simulink model "Adaptive_CT_ur10v"  (R2021b)
settings: Solver=VariableStepAuto  StartTime=0.0  StopTime=15  FixedStep=1e-4  RelTol=1e1
values from neighbouring files (symbols this model uses):
  Kp = [100 0 0 0 0 0 0 250 0 0 0 0 ... (36 elements, 6x6)]    [ACT_workspace.mat]    (also in GuadagniControllore.m = 100 * diag([1 1 2 4 5 5]))
  Kv = [100 0 0 0 0 0 0 100 0 0 0 0 ... (36 elements, 6x6)]    [ACT_workspace.mat]    (also in GuadagniControllore.m = 100 * diag([1 1 3 3 5 5]))
  l1 = 0.1273    [ACT_workspace.mat]
  l2 = -0.612    [ACT_workspace.mat]
  l3 = -0.5723    [ACT_workspace.mat]
  l4 = 0.1639    [ACT_workspace.mat]
  l5 = 0.1157    [ACT_workspace.mat]
  l6 = 0.0922    [ACT_workspace.mat]
  m1 = 7.1    [ACT_workspace.mat]
  m2 = 12.7    [ACT_workspace.mat]
  m3 = 4.27    [ACT_workspace.mat]
  m4 = 2    [ACT_workspace.mat]
  m5 = 2    [ACT_workspace.mat]
  m6 = 0.365    [ACT_workspace.mat]
  q0 = [0 0 0 0 0 0]    [ACT_workspace.mat]
  r = 0.02    [ACT_workspace.mat]
undefined symbols (not defined in the file or in its folder): B, Spline
libraries: roblocks x2, robotcorelib x1, simulink x1
(part 17 of 20)

== matlab function Adaptive_CT_ur10v/CTA control/Subsystem/reg ==
  data: q input; Y output; qd input; qdd input
function Y = reg(q, qd, qdd)
%#codegen
q1 = q(1);
q2 = q(2);
q3 = q(3);
q4 = q(4);
q5 = q(5);
q6 = q(6);
qd1 = qd(1);
qd2 = qd(2);
qd3 = qd(3);
qd4 = qd(4);
qd5 = qd(5);
qd6 = qd(6);
qdd1 = qdd(1);
qdd2 = qdd(2);
qdd3 = qdd(3);
qdd4 = qdd(4);
qdd5 = qdd(5);
qdd6 = qdd(6);

%    This function was generated by the Symbolic Math Toolbox version 9.0.
%    26-Sep-2022 09:29:38

t2 = cos(q1);
t3 = cos(q2);
t4 = cos(q3);
t5 = cos(q4);
t6 = cos(q5);
t7 = cos(q6);
t8 = sin(q1);
t9 = sin(q2);
t10 = sin(q3);
t11 = sin(q4);
t12 = sin(q5);
t13 = sin(q6);
t14 = q2+q3;
t23 = -q5;
t15 = t2.^2;
t16 = t6.^2;
t17 = t8.^2;
t18 = t9.^2;
t19 = t12.^2;
t20 = cos(t14);
t21 = q4+t14;
t22 = sin(t14);
t24 = t2.*t6;
t26 = t2.*t12;
t27 = t6.*t8;
t30 = t8.*t12;
t33 = t3.*6.12e+3;
t34 = t9.*6.12e+3;
t56 = t3.*(1.53e+2./2.5e+2);
t57 = t2.*(1.53e+2./5.0e+2);
t63 = t9.*(1.53e+2./2.5e+2);
t64 = t8.*(1.53e+2./5.0e+2);
t90 = t2.*t3.*(-1.53e+2./2.5e+2);
t91 = t3.*t8.*(-1.53e+2./2.5e+2);
t92 = t2.*1.639e-1;
t93 = t2.*2.8615e-1;
t94 = t8.*1.639e-1;
t95 = t8.*2.8615e-1;
t119 = t3.*6.00372;
t138 = t8.*t9.*t10.*5.723e-1;
t148 = t2.*t3.*t4.*5.723e-1;
t152 = t2.*t3.*t10.*5.723e-1;
t153 = t2.*t4.*t9.*5.723e-1;
t154 = t3.*t4.*t8.*5.723e-1;
t157 = t2.*t9.*t10.*5.723e-1;
t158 = t3.*t8.*t10.*5.723e-1;
t159 = t4.*t8.*t9.*5.723e-1;
t25 = cos(t21);
t28 = q5+t21;
t29 = sin(t21);
t31 = t22.^2;
t41 = t21+t23;
t42 = t20.*5.723e+3;
t43 = t22.*5.723e+3;
t44 = t15+t17;
t71 = t2.*t56;
t74 = t2.*t63;
t75 = t8.*t56;
t79 = t8.*t63;
t109 = t20.*5.723e-1;
t110 = t24.*1.383e-1;
t111 = t24.*5.785e-2;
t112 = t22.*5.723e-1;
t113 = t26.*1.383e-1;
t114 = t27.*1.383e-1;
t115 = t26.*5.785e-2;
t116 = t27.*5.785e-2;
t117 = t30.*1.383e-1;
t118 = t30.*5.785e-2;
t122 = t5.*t20.*9.22e-2;
t123 = t11.*t20.*9.22e-2;
t124 = t5.*t22.*9.22e-2;
t125 = t11.*t22.*9.22e-2;
t127 = -t119;
t147 = t5.*t20.*1.157e-1;
t149 = t11.*t20.*1.157e-1;
t150 = t5.*t22.*1.157e-1;
t155 = t11.*t22.*1.157e-1;
t161 = -t138;
t172 = -t148;
t175 = t2.*t22.*(-5.723e-1);
t177 = t8.*t22.*(-5.723e-1);
t196 = t20.*5.614263;
t215 = t8.*t11.*t20.*(-1.157e-1);
t216 = t2.*t11.*t22.*(-1.157e-1);
t217 = t5.*t8.*t22.*(-1.157e-1);
t218 = t8.*t11.*t22.*(-1.157e-1);
t259 = t57+t91;
t32 = sin(t28);
t35 = t25.^2;
t36 = t29.^2;
t37 = t7.*t25;
t38 = t13.*t25;
t39 = t7.*t29;
t40 = t13.*t29;
t45 = sin(t41);
t46 = t24.*t25;
t49 = t25.*t26;
t50 = t25.*t27;
t58 = t25.*t30;
t87 = t25.*t29.*2.0;
t96 = t6.*t25.*t29;
t97 = t12.*t25.*t29;
t126 = -t109;
t128 = t25.*1.157e-1;
t129 = t25.*8.195e-2;
t130 = t29.*1.157e-1;
t131 = t29.*8.195e-2;
t137 = -t125;
t139 = t12.*t25.*4.61e-2;
t140 = t6.*t29.*4.61e-2;
t141 = t12.*t29.*4.61e-2;
t145 = t33+t42;
t146 = t34+t43;
t151 = t2.*t112;
t156 = t8.*t112;
t164 = t12.*t25.*5.785e-2;
t167 = t12.*t29.*5.785e-2;
t173 = -t149;
t174 = -t150;
t176 = -t155;
t178 = t15.*t112;
t179 = t17.*t112;
t181 = t8.*t29.*(-8.195e-2);
t182 = t2.*t147;
t183 = t2.*t149;
t184 = t8.*t147;
t185 = t2.*t150;
t186 = t8.*t149;
t187 = t2.*t155;
t188 = t8.*t150;
t191 = t8.*t155;
t206 = t29.*t113;
t208 = t29.*t115;
t209 = t29.*t117;
t210 = t29.*t118;
t211 = (t15.*t44)./5.0e+3;
t212 = (t17.*t44)./5.0e+3;
t220 = -t196;
t228 = t29.*1.135017;
t229 = t29.*8.039295e-1;
t234 = (t19.*t25.*t29)./2.5e+3;
t235 = (t19.*t25.*t29)./5.0e+3;
t251 = t64+t71;
t274 = t56+t109;
t275 = t63+t112;
t297 = t8.*t259;
t332 = t123+t124;
t345 = t17.*t25.*t29.*3.35790125e-3;
t346 = t17.*t25.*t29.*1.007370375e-2;
t354 = t15.*t25.*t29.*3.35790125e-3;
t355 = t15.*t25.*t29.*1.007370375e-2;
t374 = t3.*t57.*t259;
t375 = t74.*t259;
t480 = t25.*t29.*4.277201666666666e-3;
t487 = t25.*t29.*2.138600833333333e-3;
t514 = t25.*t29.*1.215540833333333e-3;
t515 = t25.*t29.*2.431081666666667e-3;
t519 = t15.*t44.*2.338600833333333e-3;
t521 = t17.*t44.*2.338600833333333e-3;
t47 = t2.*t37;
t48 = t6.*t37;
t51 = t2.*t38;
t52 = t8.*t37;
t53 = t2.*t39;
t54 = t6.*t38;
t55 = t6.*t39;
t59 = t8.*t38;
t60 = t2.*t40;
t61 = t8.*t39;
t62 = t6.*t40;
t65 = t8.*t40;
t66 = t6.*t35;
t67 = t12.*t35;
t68 = t6.*t36;
t69 = t12.*t36;
t70 = t24.*t39;
t72 = t24.*t40;
t73 = t27.*t39;
t76 = t15.*t36;
t78 = t27.*t40;
t80 = t17.*t36;
t81 = t19.*t36;
t82 = -t49;
t83 = -t50;
t98 = -t87;
t120 = t12.*t29.*t37;
t121 = t12.*t29.*t38;
t132 = t24+t58;
t133 = t30+t46;
t134 = t15.*t87;
t135 = t17.*t87;
t136 = t19.*t87;
t142 = -t128;
t143 = -t130;
t144 = -t131;
t163 = t2.*t129;
t165 = t8.*t129;
t166 = t2.*t131;
t168 = t8.*t131;
t180 = -t164;
t199 = t46.*1.383e-1;
t200 = t46.*5.785e-2;
t201 = t49.*1.383e-1;
t202 = t50.*1.383e-1;
t203 = t49.*5.785e-2;
t204 = t50.*5.785e-2;
t205 = t58.*1.383e-1;
t207 = t58.*5.785e-2;
t213 = t15.*t129;
t214 = t17.*t129;
t240 = t36.*t111;
t241 = t36.*t116;
t242 = -t234;
t243 = -t235;
t244 = t32.*6.783615e-1;
t245 = t32.*2.8375425e-1;
t250 = t27.*t36.*(-5.785e-2);
t264 = t45.*6.783615e-1;
t265 = t45.*2.8375425e-1;
t277 = t2.*t251;
t294 = (t2.*t145)./1.0e+4;
t295 = (t8.*t145)./1.0e+4;
t296 = (t2.*t146)./1.0e+4;
t299 = (t8.*t146)./1.0e+4;
t300 = t275.^2;
t315 = (t15.*t146)./1.0e+4;
t320 = (t17.*t146)./1.0e+4;
t322 = -t297;
t339 = t122+t137;
t342 = t112+t129;
t351 = t126+t131;
t357 = t6.*t332;
t358 = t12.*t332;
t361 = t128+t167;
t365 = t3.*t64.*t251;
t366 = t79.*t251;
t387 = t178+t179;
t405 = t129+t275;
t444 = t179.*t275;
t450 = t15.*t22.*t274.*2.8615e-1;
t452 = t15.*t20.*t275.*2.8615e-1;
t453 = t17.*t22.*t274.*2.8615e-1;
t458 = t178.*t275;
t459 = t17.*t20.*t275.*2.8615e-1;
t478 = t35.*1.215540833333333e-3;
t490 = t2.*t36.*1.215540833333333e-3;
t492 = t8.*t36.*1.215540833333333e-3;
t516 = t16.*t36.*1.215540833333333e-3;
t524 = -t515;
t525 = -t514;
t534 = t2.*t514;
t535 = t8.*t514;
t549 = t16.*t514;
t550 = t16.*t515;
t574 = t182+t206+t216;
t575 = t182+t208+t216;
t576 = t184+t209+t218;
t577 = t184+t210+t218;
t646 = t92+t154+t161+t181;
t77 = -t48;
t84 = -t60;
t85 = -t61;
t86 = -t62;
t88 = -t68;
t89 = -t69;
t99 = t12.*t68.*2.0;
t100 = t17.*t69;
t101 = t13.*t81;
t102 = -t72;
t103 = -t78;
t105 = t15.*t68;
t106 = t17.*t68;
t107 = t15.*t69;
t108 = t7.*t81;
t160 = t132.^2;
t162 = t81./5.0e+3;
t169 = (t12.*t68)./2.5e+3;
t170 = t26+t83;
t171 = t27+t82;
t189 = t2.*t132;
t190 = t7.*t133;
t192 = t38+t55;
t193 = t39+t54;
t194 = t8.*t133;
t195 = t13.*t133;
t221 = -t201;
t222 = -t202;
t223 = -t203;
t224 = -t204;
t249 = t51+t70;
t252 = t59+t73;
t255 = -t244;
t256 = -t245;
t257 = t8.*t81.*1.383e-1;
t258 = t8.*t29.*t132;
t260 = t2.*t25.*t133;
t261 = t2.*t81.*1.383e-1;
t262 = t8.*t25.*t132;
t263 = t2.*t29.*t133;
t278 = t61.*t132;
t282 = t65.*t132;
t298 = t29.*t30.*t132.*2.0;
t303 = -t295;
t308 = -t296;
t311 = -t299;
t323 = (t12.*t29.*t132)./5.0e+3;
t324 = (t12.*t29.*t133)./5.0e+3;
t327 = (t12.*t25.*t132)./5.0e+3;
t328 = (t6.*t29.*t132)./5.0e+3;
t338 = t35+t76+t80;
t356 = t342.^2;
t362 = t12.*t339;
t368 = t130+t180;
t369 = t110+t205;
t370 = t117+t199;
t371 = t118+t200;
t376 = t132.*t206;
t377 = t361.^2;
t400 = t95+t294;
t402 = t213+t214;
t420 = t144+t274;
t421 = t2.*t25.*t361;
t422 = t8.*t25.*t361;
t423 = t2.*t29.*t361;
t424 = t8.*t29.*t361;
t429 = t405.^2;
t431 = -t2.*(t296-t2.*t9.*(1.53e+2./2.5e+2));
t437 = -t8.*(t299-t8.*t9.*(1.53e+2./2.5e+2));
t461 = t98+t134+t135;
t479 = t112+t361;
t481 = t109+t143+t164;
t488 = t2.*t478;
t489 = t8.*t478;
t491 = t140+t357;
t493 = t213.*t342;
t494 = t214.*t342;
t495 = t15.*t131.*t342;
t496 = t15.*t29.*t342.*4.0975e-2;
t498 = t17.*t131.*t342;
t499 = t17.*t29.*t342.*4.0975e-2;
t500 = -t490;
t501 = -t492;
t502 = t152+t153+t163;
t505 = t213.*t351;
t506 = t15.*t25.*t351.*4.0975e-2;
t507 = t214.*t351;
t508 = t17.*t25.*t351.*4.0975e-2;
t513 = t158+t159+t165;
t536 = t277+t322;
t537 = t16.*t490;
t538 = t16.*t492;
t558 = t6.*t15.*t29.*t361.*5.785e-2;
t559 = t6.*t15.*t29.*t361.*2.8925e-2;
t560 = t6.*t17.*t29.*t361.*5.785e-2;
t561 = t6.*t17.*t29.*t361.*2.8925e-2;
t568 = t315+t320;
t580 = t275+t361;
t581 = t143+t164+t274;
t583 = t213.*t405;
t584 = t214.*t405;
t585 = t15.*t131.*t405;
t586 = t15.*t29.*t405.*4.0975e-2;
t588 = t17.*t131.*t405;
t589 = t17.*t29.*t405.*4.0975e-2;
t590 = t2.*t574;
t591 = t2.*t575;
t592 = t8.*t576;
t593 = t8.*t577;
t613 = t6.*t25.*t133.*1.215540833333333e-3;
t614 = t6.*t29.*t132.*1.015540833333333e-3;
t615 = t6.*t29.*t133.*1.215540833333333e-3;
t616 = t12.*t29.*t133.*1.015540833333333e-3;
t618 = t25.*t574;
t619 = t25.*t575;
t620 = t25.*t576;
t621 = t25.*t577;
t632 = t94+t157+t166+t172;
t639 = t8.*t29.*t574;
t640 = t8.*t29.*t575;
t642 = t2.*t29.*t576;
t643 = t2.*t29.*t577;
t654 = t8.*t646;
t667 = t365+t374;
t674 = t366+t375;
t690 = t111+t207+t215+t217;
t700 = t15.*t342.*t405;
t701 = t17.*t342.*t405;
t702 = t75+t646;
t752 = (t15.*t351.*t405)./2.0;
t754 = (t17.*t351.*t405)./2.0;
t773 = t141+t147+t176+t358;
t828 = t158+t159+t576;
t829 = t158+t159+t577;
t835 = t152+t153+t574;
t836 = t152+t153+t575;
t886 = (t8.*t361.*t575)./2.0;
t887 = (t2.*t361.*t577)./2.0;
t1073 = t234+t524+t550;
t104 = -t99;
t197 = t171.^2;
t198 = t8.*t162;
t219 = t2.*t162;
t225 = t7.*t160;
t226 = t192.^2;
t227 = t13.*t160;
t230 = t7.*t189;
t231 = t13.*t189;
t232 = t2.*t170;
t233 = t7.*t170;
t236 = t37+t86;
t237 = t40+t77;
t238 = t8.*t171;
t239 = t13.*t170;
t266 = t25.*t192;
t267 = t25.*t193;
t268 = t29.*t192;
t269 = t47+t102;
t270 = t52+t103;
t271 = -t261;
t272 = t8.*t29.*t170;
t273 = -t258;
t276 = t8.*t249;
t279 = t2.*t252;
t280 = t2.*t25.*t171;
t281 = -t260;
t283 = t8.*t25.*t170;
t284 = t2.*t29.*t171;
t285 = -t262;
t286 = -t263;
t290 = t12.*t29.*t193;
t301 = t53.*t171;
t304 = t60.*t171;
t305 = t85.*t132;
t309 = -t298;
t310 = -t282;
t321 = t26.*t29.*t171.*2.0;
t325 = t53+t195;
t329 = -t323;
t330 = -t324;
t331 = t8.*t29.*t252;
t334 = t2.*t29.*t249;
t335 = -t327;
t336 = (t12.*t29.*t170)./5.0e+3;
t337 = (t12.*t29.*t171)./5.0e+3;
t340 = t84+t190;
t343 = (t12.*t25.*t171)./5.0e+3;
t344 = (t6.*t29.*t171)./5.0e+3;
t364 = -t8.*(t60-t190);
t372 = t132.*t170.*2.0;
t373 = t133.*t171.*2.0;
t378 = t113+t222;
t379 = t114+t221;
t380 = t115+t224;
t384 = t171.*t209;
t385 = t2.*t370;
t386 = t2.*t371;
t388 = t132.*t252;
t390 = -t2.*t25.*(t60-t190);
t392 = -t2.*t29.*(t60-t190);
t399 = t74+t308;
t401 = t79+t311;
t403 = t25.*t370;
t404 = t25.*t371;
t406 = t93+t303;
t407 = t171.*t249;
t410 = -t26.*t29.*(t60-t190);
t411 = t2.*t29.*(t60-t190);
t425 = t8.*t29.*t370;
t426 = t12.*t29.*t369;
t427 = t12.*t29.*t370;
t428 = t8.*t29.*t371;
t432 = t2.*t29.*t368;
t433 = t2.*t400;
t434 = t8.*t29.*t368;
t436 = t26.*t29.*(t60-t190);
t440 = t12.*t25.*t369;
t441 = t6.*t29.*t369;
t445 = -t421;
t446 = -t422;
t447 = -t423;
t463 = t26.*t29.*t369;
t474 = -t133.*(t60-t190);
t482 = -t171.*(t60-t190);
t483 = t133.*(t60-t190);
t497 = t479.^2;
t509 = -t496;
t510 = t132.*t370;
t511 = t133.*t369;
t512 = -t499;
t517 = t90+t400;
t520 = -t506;
t522 = -t508;
t532 = t171.*t369;
t547 = t2.*t502;
t548 = t8.*t513;
t562 = t8.*t109.*t400;
t563 = t20.*t95.*t400;
t565 = t156.*t400;
t578 = t2.*t29.*t491;
Y = ft_1({qd1,qd2,qd3,qd4,qd5,qd6,qdd1,qdd2,qdd3,qdd4,qdd5,qdd6,t100,t101,t104,t105,t106,t107,t1073,t108,t109,t111,t112,t116,t12,t120,t121,t127,t13,t130,t132,t133,t136,t139,t142,t144,t146,t15,t151,t154,t157,t160,t161,t162,t163,t165,t166,t168,t169,t17,t170,t171,t172,t173,t174,t175,t177,t178,t179,t18,t183,t185,t189,t190,t192,t193,t194,t197,t198,t2,t20,t211,t212,t213,t214,t215,t217,t219,t22,t220,t223,t225,t226,t227,t228,t229,t230,t231,t232,t233,t235,t236,t237,t238,t239,t24,t240,t241,t242,t243,t249,t25,t250,t251,t252,t255,t256,t257,t259,t26,t261,t264,t265,t266,t267,t268,t269,t27,t270,t271,t272,t273,t274,t275,t276,t277,t279,t280,t281,t283,t284,t285,t286,t29,t290,t294,t296,t297,t299,t3,t30,t300,t301,t303,t304,t305,t309,t31,t310,t321,t323,t324,t325,t328,t329,t330,t331,t334,t335,t336,t337,t338,t342,t343,t344,t345,t346,t35,t351,t354,t355,t356,t36,t361,t362,t364,t368,t369,t370,t371,t372,t373,t376,t377,t378,t379,t380,t384,t385,t386,t387,t388,t39,t390,t399,t40,t400,t401,t402,t403,t404,t405,t406,t407,t411,t420,t421,t423,t424,t425,t426,t427,t428,t429,t431,t432,t433,t434,t436,t437,t440,t441,t444,t445,t446,t447,t450,t452,t453,t458,t459,t461,t463,t478,t479,t480,t481,t482,t483,t487,t488,t489,t491,t493,t494,t495,t496,t497,t498,t499,t500,t501,t502,t505,t506,t507,t508,t509,t510,t511,t512,t513,t516,t517,t519,t520,t521,t522,t525,t532,t534,t535,t536,t537,t538,t547,t548,t549,t558,t559,t560,t561,t562,t563,t565,t568,t574,t575,t576,t577,t578,t580,t581,t583,t584,t585,t586,t588,t589,t590,t591,t592,t593,t6,t60,t61,t613,t614,t615,t616,t618,t619,t620,t621,t63,t632,t639,t640,t642,t643,t65,t654,t66,t667,t67,t674,t68,t690,t7,t700,t701,t702,t71,t74,t75,t752,t754,t773,t79,t8,t81,t828,t829,t835,t836,t85,t88,t886,t887,t89,t9,t90,t92,t93,t94,t96,t97});
end
function Y = ft_1(ct)
qd1 = ct{1};
qd2 = ct{2};
qd3 = ct{3};
qd4 = ct{4};
qd5 = ct{5};
qd6 = ct{6};
qdd1 = ct{7};
qdd2 = ct{8};
qdd3 = ct{9};
qdd4 = ct{10};
qdd5 = ct{11};
qdd6 = ct{12};
t100 = ct{13};
t101 = ct{14};
t104 = ct{15};
t105 = ct{16};
t106 = ct{17};
t107 = ct{18};
t1073 = ct{19};
t108 = ct{20};
t109 = ct{21};
t111 = ct{22};
t112 = ct{23};
t116 = ct{24};
t12 = ct{25};
t120 = ct{26};
t121 = ct{27};
t127 = ct{28};
t13 = ct{29};
t130 = ct{30};
t132 = ct{31};
t133 = ct{32};
t136 = ct{33};
t139 = ct{34};
t142 = ct{35};
t144 = ct{36};
t146 = ct{37};
t15 = ct{38};
t151 = ct{39};
t154 = ct{40};
t157 = ct{41};
t160 = ct{42};
t161 = ct{43};
t162 = ct{44};
t163 = ct{45};
t165 = ct{46};
t166 = ct{47};
t168 = ct{48};
t169 = ct{49};
t17 = ct{50};
t170 = ct{51};
t171 = ct{52};
t172 = ct{53};
t173 = ct{54};
t174 = ct{55};
t175 = ct{56};
t177 = ct{57};
t178 = ct{58};
t179 = ct{59};
t18 = ct{60};
t183 = ct{61};
t185 = ct{62};
t189 = ct{63};
t190 = ct{64};
t192 = ct{65};
t193 = ct{66};
t194 = ct{67};
t197 = ct{68};
t198 = ct{69};
t2 = ct{70};
t20 = ct{71};
t211 = ct{72};
t212 = ct{73};
t213 = ct{74};
t214 = ct{75};
t215 = ct{76};
t217 = ct{77};
t219 = ct{78};
t22 = ct{79};
t220 = ct{80};
t223 = ct{81};
t225 = ct{82};
t226 = ct{83};
t227 = ct{84};
t228 = ct{85};
t229 = ct{86};
t230 = ct{87};
t231 = ct{88};
t232 = ct{89};
t233 = ct{90};
t235 = ct{91};
t236 = ct{92};
t237 = ct{93};
t238 = ct{94};
t239 = ct{95};
t24 = ct{96};
t240 = ct{97};
t241 = ct{98};
t242 = ct{99};
t243 = ct{100};
t249 = ct{101};
t25 = ct{102};
t250 = ct{103};
t251 = ct{104};
t252 = ct{105};
t255 = ct{106};
t256 = ct{107};
t257 = ct{108};
t259 = ct{109};
t26 = ct{110};
t261 = ct{111};
t264 = ct{112};
t265 = ct{113};
t266 = ct{114};
t267 = ct{115};
t268 = ct{116};
t269 = ct{117};
t27 = ct{118};
t270 = ct{119};
t271 = ct{120};
t272 = ct{121};
t273 = ct{122};
t274 = ct{123};
t275 = ct{124};
t276 = ct{125};
t277 = ct{126};
t279 = ct{127};
t280 = ct{128};
t281 = ct{129};
t283 = ct{130};
t284 = ct{131};
t285 = ct{132};
t286 = ct{133};
t29 = ct{134};
t290 = ct{135};
t294 = ct{136};
t296 = ct{137};
t297 = ct{138};
t299 = ct{139};
t3 = ct{140};
t30 = ct{141};
t300 = ct{142};
t301 = ct{143};
t303 = ct{144};
t304 = ct{145};
t305 = ct{146};
t309 = ct{147};
t31 = ct{148};
t310 = ct{149};
t321 = ct{150};
t323 = ct{151};
t324 = ct{152};
t325 = ct{153};
t328 = ct{154};
t329 = ct{155};
t330 = ct{156};
t331 = ct{157};
t334 = ct{158};
t335 = ct{159};
t336 = ct{160};
t337 = ct{161};
t338 = ct{162};
t342 = ct{163};
t343 = ct{164};
t344 = ct{165};
t345 = ct{166};
t346 = ct{167};
t35 = ct{168};
t351 = ct{169};
t354 = ct{170};
t355 = ct{171};
t356 = ct{172};
t36 = ct{173};
t361 = ct{174};
t362 = ct{175};
t364 = ct{176};
t368 = ct{177};
t369 = ct{178};
t370 = ct{179};
t371 = ct{180};
t372 = ct{181};
t373 = ct{182};
t376 = ct{183};
t377 = ct{184};
t378 = ct{185};
t379 = ct{186};
t380 = ct{187};
t384 = ct{188};
t385 = ct{189};
t386 = ct{190};
t387 = ct{191};
t388 = ct{192};
t39 = ct{193};
t390 = ct{194};
t399 = ct{195};
t40 = ct{196};
t400 = ct{197};
t401 = ct{198};
t402 = ct{199};
t403 = ct{200};
t404 = ct{201};
t405 = ct{202};
t406 = ct{203};
t407 = ct{204};
t411 = ct{205};
t420 = ct{206};
t421 = ct{207};
t423 = ct{208};
t424 = ct{209};
t425 = ct{210};
t426 = ct{211};
t427 = ct{212};
t428 = ct{213};
t429 = ct{214};
t431 = ct{215};
t432 = ct{216};
t433 = ct{217};
t434 = ct{218};
t436 = ct{219};
t437 = ct{220};
t440 = ct{221};
t441 = ct{222};
t444 = ct{223};
t445 = ct{224};
t446 = ct{225};
t447 = ct{226};
t450 = ct{227};
t452 = ct{228};
t453 = ct{229};
t458 = ct{230};
t459 = ct{231};
t461 = ct{232};
t463 = ct{233};
t478 = ct{234};
t479 = ct{235};
t480 = ct{236};
t481 = ct{237};
t482 = ct{238};
t483 = ct{239};
t487 = ct{240};
t488 = ct{241};
t489 = ct{242};
t491 = ct{243};
t493 = ct{244};
t494 = ct{245};
t495 = ct{246};
t496 = ct{247};
t497 = ct{248};
t498 = ct{249};
t499 = ct{250};
t500 = ct{251};
t501 = ct{252};
t502 = ct{253};
t505 = ct{254};
t506 = ct{255};
t507 = ct{256};
t508 = ct{257};
t509 = ct{258};
t510 = ct{259};
t511 = ct{260};
t512 = ct{261};
t513 = ct{262};
t516 = ct{263};
t517 = ct{264};
t519 = ct{265};
t520 = ct{266};
t521 = ct{267};
t522 = ct{268};
t525 = ct{269};
t532 = ct{270};
t534 = ct{271};
t535 = ct{272};
t536 = ct{273};
t537 = ct{274};
t538 = ct{275};
t547 = ct{276};
t548 = ct{277};
t549 = ct{278};
t558 = ct{279};
t559 = ct{280};
t560 = ct{281};
t561 = ct{282};
t562 = ct{283};
t563 = ct{284};
t565 = ct{285};
t568 = ct{286};
t574 = ct{287};
t575 = ct{288};
t576 = ct{289};
t577 = ct{290};
t578 = ct{291};
t580 = ct{292};
t581 = ct{293};
t583 = ct{294};
t584 = ct{295};
t585 = ct{296};
t586 = ct{297};
t588 = ct{298};
t589 = ct{299};
t590 = ct{300};
t591 = ct{301};
t592 = ct{302};
t593 = ct{303};
t6 = ct{304};
t60 = ct{305};
t61 = ct{306};
t613 = ct{307};
t614 = ct{308};
t615 = ct{309};
t616 = ct{310};
t618 = ct{311};
t619 = ct{312};
t620 = ct{313};
t621 = ct{314};
t63 = ct{315};
t632 = ct{316};
t639 = ct{317};
t640 = ct{318};
t642 = ct{319};
t643 = ct{320};
t65 = ct{321};
t654 = ct{322};
t66 = ct{323};
t667 = ct{324};
t67 = ct{325};
t674 = ct{326};
t68 = ct{327};
t690 = ct{328};
t7 = ct{329};
t700 = ct{330};
t701 = ct{331};
t702 = ct{332};
t71 = ct{333};
t74 = ct{334};
t75 = ct{335};
t752 = ct{336};
t754 = ct{337};
t773 = ct{338};
t79 = ct{339};
t8 = ct{340};
t81 = ct{341};
t828 = ct{342};
t829 = ct{343};
t835 = ct{344};
t836 = ct{345};
t85 = ct{346};
t88 = ct{347};
t886 = ct{348};
t887 = ct{349};
t89 = ct{350};
t9 = ct{351};
t90 = ct{352};
t92 = ct{353};
t93 = ct{354};
t94 = ct{355};
t96 = ct{356};
t97 = ct{357};
t579 = t8.*t29.*t491;
t587 = t580.^2;
t594 = t15.*t25.*t420.*4.0975e-2;
t595 = t17.*t25.*t420.*4.0975e-2;
t596 = -t586;
t597 = -t589;
t605 = t74+t502;
t606 = t79+t513;
t628 = -t613;
t629 = -t614;
t630 = -t615;
t635 = t6.*t25.*t170.*1.215540833333333e-3;
t636 = t6.*t29.*t170.*1.215540833333333e-3;
t637 = t6.*t29.*t171.*1.015540833333333e-3;
t638 = t12.*t29.*t170.*1.015540833333333e-3;
t641 = -t618;
t647 = t132.*t491;
t649 = t2.*t632;
t650 = t8.*t275.*t400;
t651 = -t642;
t652 = -t643;
t653 = t171.*t491;
t656 = t175+t502;
t657 = t177+t513;
t660 = t165.*t502;
t661 = t8.*t25.*t502.*4.0975e-2;
t662 = t12.*t39.*t192.*1.616806666666667e-3;
t663 = t163.*t513;
t664 = t2.*t25.*t513.*4.0975e-2;
t668 = t8.*t25.*t502.*(-8.195e-2);
t669 = t6.*t15.*t29.*t479.*5.785e-2;
t670 = t6.*t15.*t29.*t479.*2.8925e-2;
t672 = t6.*t17.*t29.*t479.*5.785e-2;
t673 = t6.*t17.*t29.*t479.*2.8925e-2;
t675 = -t654;
t676 = (t8.*t274.*t400)./2.0;
t679 = t8.*t361.*t371;
t687 = t116+t183+t185+t223;
t689 = t215+t217+t369;
t696 = (t15.*t361.*t368)./2.0;
t697 = t15.*t361.*t368.*(3.0./2.0);
t698 = (t17.*t361.*t368)./2.0;
t699 = t17.*t361.*t368.*(3.0./2.0);
t707 = t7.*t132.*t192.*8.084033333333334e-4;
t708 = t90+t632;
t709 = t25.*t338.*1.215540833333333e-3;
t710 = t29.*t338.*6.077704166666666e-4;
t711 = t29.*t338.*1.215540833333333e-3;
t723 = t6.*t15.*t29.*t580.*5.785e-2;
t724 = t6.*t15.*t29.*t580.*2.8925e-2;
t726 = t6.*t17.*t29.*t580.*5.785e-2;
t727 = t6.*t17.*t29.*t580.*2.8925e-2;
t730 = t7.*t171.*t192.*8.084033333333334e-4;
t734 = t25.*t690;
t737 = t29.*t690;
t744 = t8.*t702;
t750 = (t15.*t342.*t420)./2.0;
t753 = (t17.*t342.*t420)./2.0;
t761 = t12.*t39.*(t60-t190).*(-8.084033333333334e-4);
t770 = t192.*t249.*8.084033333333334e-4;
t771 = t192.*t252.*8.084033333333334e-4;
t776 = t8.*t371.*t479;
t777 = t773.^2;
t781 = t431+t437;
t785 = t139+t173+t174+t362;
t786 = t15.*t361.*t479;
t788 = t17.*t361.*t479;
t793 = t15.*t361.*t481;
t794 = t15.*t368.*t479;
t795 = t17.*t361.*t481;
t796 = t17.*t368.*t479;
t797 = (t8.*t342.*t502)./2.0;
t800 = (t2.*t342.*t513)./2.0;
t830 = t25.*t461.*6.077704166666666e-4;
t831 = t25.*t461.*1.215540833333333e-3;
t833 = t192.*(t60-t190).*(-8.084033333333334e-4);
t839 = t2.*t25.*t773;
t840 = t8.*t25.*t773;
t841 = t2.*t29.*t773;
t842 = t8.*t29.*t773;
t843 = t192.*(t60-t190).*8.084033333333334e-4;
t846 = t2.*t29.*t461.*1.215540833333333e-3;
t847 = t8.*t29.*t461.*1.215540833333333e-3;
t853 = t2.*t835;
t854 = t2.*t836;
t859 = t8.*t828;
t860 = t8.*t829;
t862 = t2.*t405.*t513;
t866 = t163.*t702;
t867 = t166.*t702;
t868 = t2.*t29.*t702.*4.0975e-2;
t870 = t8.*t405.*t502;
t873 = t8.*t371.*t580;
t874 = t15.*t361.*t580;
t876 = t17.*t361.*t580;
t884 = t15.*t368.*t580;
t885 = t17.*t368.*t580;
t890 = t112+t773;
t895 = -t886;
t905 = (t15.*t361.*t581)./2.0;
t906 = (t17.*t361.*t581)./2.0;
t910 = t142+t773;
t915 = t74+t835;
t916 = t74+t836;
t917 = t79+t828;
t918 = t79+t829;
t927 = t303+t702;
t939 = t177+t828;
t940 = t177+t829;
t942 = t275+t773;
t944 = t175+t835;
t945 = t175+t836;
t951 = t8.*t479.*t575;
t952 = t2.*t479.*t577;
t961 = t2.*t342.*t702;
t962 = t15.*t479.*t580;
t965 = t17.*t479.*t580;
t968 = t2.*t351.*t702;
t992 = (t15.*t479.*t581)./2.0;
t993 = (t15.*t481.*t580)./2.0;
t994 = (t17.*t479.*t581)./2.0;
t995 = (t17.*t481.*t580)./2.0;
t1006 = t2.*t577.*t580;
t1009 = t162+t478+t516;
t1020 = t8.*t575.*t580;
t1022 = t92+t154+t161+t690;
t1028 = t2.*t405.*t702;
t1039 = t8.*t370.*t773;
t1040 = t590+t592;
t1041 = t591+t593;
t1053 = (t2.*t420.*t702)./2.0;
t1067 = t8.*t361.*t836;
t1072 = t2.*t361.*t829;
t1124 = t25.*t1073;
t1139 = t15.*t491.*t773;
t1140 = t17.*t491.*t773;
t1166 = (t8.*t479.*t836)./2.0;
t1167 = (t2.*t479.*t829)./2.0;
t1175 = (t8.*t574.*t773)./2.0;
t1176 = (t2.*t576.*t773)./2.0;
t1191 = t2.*t580.*t829;
t1200 = t8.*t580.*t836;
t1337 = t8.*t773.*t835;
t1338 = t2.*t773.*t828;
t246 = t7.*t197;
t247 = t236.^2;
t248 = t13.*t197;
t253 = t7.*t238;
t254 = t13.*t238;
t287 = t12.*t266;
t288 = t6.*t268;
t289 = t12.*t268;
t291 = t25.*t236;
t292 = t25.*t237;
t293 = t29.*t236;
t302 = t8.*t269;
t306 = t2.*t270;
t307 = -t279;
t317 = t12.*t29.*t237;
t319 = -t290;
t341 = t65+t233;
t347 = -t336;
t348 = t8.*t29.*t270;
t349 = -t331;
t350 = t8.*t325;
t352 = t2.*t29.*t269;
t353 = -t334;
t359 = t85+t239;
t381 = -t2.*(t61-t239);
t382 = t2.*t25.*t325;
t383 = t2.*t29.*t325;
t389 = t26.*t29.*t325;
t394 = t8.*t378;
t395 = t8.*t380;
t397 = t189+t238;
t398 = t194+t232;
t408 = t132.*t270;
t409 = -t388;
t413 = -t8.*t25.*(t61-t239);
t417 = -t8.*t29.*(t61-t239);
t418 = t25.*t378;
t419 = t25.*t380;
t430 = t171.*t269;
t438 = -t29.*t30.*(t61-t239);
t439 = t8.*t29.*(t61-t239);
t442 = t12.*t29.*t378;
t443 = t12.*t29.*t379;
t448 = t8.*t406;
t454 = t2.*t29.*t378;
t455 = t12.*t25.*t379;
t456 = t6.*t29.*t379;
t457 = t2.*t29.*t380;
t460 = -t426;
t462 = t29.*t30.*(t61-t239);
t464 = -t440;
t465 = -t441;
t467 = t133.*t325;
t469 = t29.*t30.*t379;
t472 = -t463;
t473 = t171.*t325;
t485 = -t132.*(t61-t239);
t486 = t81+t160+t197;
t503 = -t170.*(t61-t239);
t518 = t75+t406;
t523 = t132.*t379;
t529 = t170.*(t61-t239);
t533 = -t511;
t545 = t170.*t379;
t546 = t171.*t378;
t555 = t2.*t517;
t556 = -t532;
t570 = t2.*t109.*t406;
t571 = t20.*t93.*t406;
t572 = t151.*t406;
t582 = -t579;
t601 = t226.*8.084033333333334e-4;
t602 = t240+t404;
t622 = t96+t272+t286;
t624 = t97+t273+t284;
t634 = t8.*t606;
t644 = t2.*t605;
t648 = -t637;
t655 = t2.*t275.*t406;
t665 = t120+t301+t305;
t666 = t121+t304+t310;
t671 = -t662;
t677 = t12.*t40.*t236.*1.616806666666667e-3;
t678 = t136+t309+t321;
t680 = (t2.*t274.*t406)./2.0;
t683 = t2.*t656;
t684 = t8.*t657;
t685 = t2.*t361.*t380;
t686 = t183+t185+t379;
t693 = t679./2.0;
t714 = -t707;
t716 = t25.*t687;
t718 = t29.*t687;
t719 = -t711;
t720 = -t710;
t731 = t12.*t40.*t325.*8.084033333333334e-4;
t732 = t13.*t132.*t236.*8.084033333333334e-4;
t733 = t25.*t689;
t735 = t2.*t709;
t736 = t29.*t689;
t738 = t8.*t709;
t739 = t2.*t711;
t740 = t8.*t711;
t741 = t2.*t708;
t742 = t163.*t606;
t743 = t2.*t25.*t606.*4.0975e-2;
t747 = -t730;
t755 = t192.*t237.*8.084033333333334e-4;
t756 = t192.*t237.*1.616806666666667e-3;
t757 = t193.*t236.*8.084033333333334e-4;
t758 = t193.*t236.*1.616806666666667e-3;
t759 = t165.*t605;
t760 = t8.*t25.*t605.*4.0975e-2;
t763 = t2.*t734;
t765 = t13.*t171.*t236.*8.084033333333334e-4;
t767 = t2.*t737;
t768 = t8.*t25.*t605.*(-8.195e-2);
t769 = -t744;
t772 = t12.*t40.*(t61-t239).*(-8.084033333333334e-4);
t774 = t104+t372+t373;
t779 = t236.*t269.*8.084033333333334e-4;
t780 = t236.*t270.*8.084033333333334e-4;
t787 = t2.*t380.*t479;
t809 = t776./2.0;
t810 = t193.*t325.*8.084033333333334e-4;
t811 = -t797;
t820 = t399+t502;
t823 = t401+t513;
t824 = t793./2.0;
t825 = t794./2.0;
t826 = t795./2.0;
t827 = t796./2.0;
t832 = t236.*t325.*8.084033333333334e-4;
t848 = t237.*(t60-t190).*(-8.084033333333334e-4);
t850 = t193.*(t61-t239).*(-8.084033333333334e-4);
t855 = t2.*t29.*t785;
t856 = t8.*t29.*t785;
t857 = -t840;
t858 = -t841;
t863 = t165.*t708;
t864 = t168.*t708;
t865 = t8.*t29.*t708.*4.0975e-2;
t869 = t236.*(t61-t239).*(-8.084033333333334e-4);
t875 = t2.*t380.*t580;
t880 = t8.*t342.*t605;
t881 = -t870;
t882 = t2.*t342.*t606;
t883 = t862./2.0;
t889 = t870./2.0;
t891 = t873./2.0;
t899 = t66+t88+t105+t106+t281+t283;
t901 = t67+t89+t100+t107+t280+t285;
t902 = t403+t578;
t904 = t109+t785;
t907 = t884./2.0;
t908 = t885./2.0;
t909 = t890.^2;
t913 = t130+t785;
t920 = t294+t708;
t928 = t2.*t915;
t929 = t2.*t916;
t930 = t8.*t917;
t931 = t8.*t918;
t937 = t8.*t927;
t947 = (t8.*t405.*t605)./2.0;
t948 = t547+t548;
t949 = (t2.*t405.*t606)./2.0;
t953 = t274+t785;
t955 = t26.*t29.*t910;
t956 = t942.^2;
t957 = t29.*t30.*t910;
t958 = t8.*t342.*t708;
t959 = t2.*t944;
t960 = t2.*t945;
t963 = t8.*t939;
t964 = t8.*t940;
t966 = -t951;
t967 = t8.*t351.*t708;
t974 = t951./2.0;
t975 = t952./2.0;
t990 = t968./2.0;
t1001 = t132.*t910;
t1002 = t133.*t910;
t1011 = t94+t157+t172+t687;
t1012 = t170.*t910;
t1013 = t171.*t910;
t1021 = t92+t154+t161+t689;
t1027 = t8.*t405.*t708;
t1030 = -t1020;
t1031 = t1006./2.0;
t1036 = t424+t734;
t1038 = t1020./2.0;
t1047 = t8.*t1022;
t1049 = t2.*t378.*t773;
t1052 = (t8.*t420.*t708)./2.0;
t1054 = t29.*t1009;
t1057 = t1039./2.0;
t1079 = t401+t828;
t1080 = t401+t829;
t1081 = -t1067;
t1088 = t399+t835;
t1089 = t399+t836;
t1091 = t1067./2.0;
t1093 = t1072./2.0;
t1098 = t629+t638;
t1102 = t75+t1022;
t1116 = -t2.*(t614-t638);
t1125 = t8.*t370.*t890;
t1129 = t2.*(t614-t638).*(-1.0./2.0);
t1131 = t1124./2.0;
t1132 = t2.*t378.*t890;
t1133 = (t2.*(t614-t638))./2.0;
t1137 = t8.*t361.*t916;
t1138 = t649+t675;
t1141 = t2.*t361.*t918;
t1152 = t1139./2.0;
t1155 = t1140./2.0;
t1168 = t8.*t370.*t942;
t1169 = -t1167;
t1170 = t2.*t378.*t942;
t1181 = -t1175;
t1183 = t337+t534+t630;
t1184 = t329+t535+t636;
t1207 = -t1191;
t1208 = t8.*t479.*t916;
t1212 = t15.*t491.*t890;
t1213 = t17.*t491.*t890;
t1214 = t2.*t479.*t918;
t1215 = t1191./2.0;
t1220 = t1200./2.0;
t1246 = t8.*t574.*t890;
t1247 = t2.*t576.*t890;
t1268 = t15.*t491.*t942;
t1270 = t17.*t491.*t942;
t1287 = (t2.*t580.*t918)./2.0;
t1292 = (t8.*t580.*t916)./2.0;
t1304 = t8.*t574.*t942;
t1306 = t2.*t576.*t942;
t1339 = (t15.*t773.*t785)./2.0;
t1340 = t15.*t773.*t785.*(3.0./2.0);
t1341 = (t17.*t773.*t785)./2.0;
t1342 = t17.*t773.*t785.*(3.0./2.0);
t1348 = t1337./2.0;
t1350 = t1338./2.0;
t1392 = t15.*t773.*t890;
t1393 = t17.*t773.*t890;
t1395 = t853+t859;
t1396 = t854+t860;
t1402 = t8.*t773.*t915;
t1406 = t2.*t773.*t917;
t1407 = t15.*t785.*t890;
t1409 = t17.*t785.*t890;
t1440 = (t8.*t835.*t890)./2.0;
t1441 = (t2.*t828.*t890)./2.0;
t1448 = t15.*t773.*t942;
t1449 = t17.*t773.*t942;
t1454 = t17.*t785.*t942;
t1458 = t15.*t785.*t942;
t1465 = t8.*t835.*t942;
t1468 = t2.*t828.*t942;
t1476 = t8.*t890.*t915;
t1478 = t2.*t890.*t917;
t1493 = t15.*t890.*t942;
t1494 = t17.*t890.*t942;
t1506 = (t2.*t917.*t942)./2.0;
t1512 = (t8.*t915.*t942)./2.0;
t1566 = t434+t446+t621+t737;
t1675 = t219+t343+t488+t500+t537+t628;
t1677 = t198+t335+t489+t501+t538+t635;
t312 = t12.*t291;
t313 = t6.*t293;
t314 = -t288;
t316 = t12.*t293;
t318 = -t289;
t326 = -t306;
t333 = -t317;
t360 = -t348;
t363 = t2.*t341;
t367 = -t352;
t391 = -t382;
t393 = t8.*t25.*t341;
t396 = t8.*t29.*t341;
t412 = t29.*t30.*t341;
t415 = -t394;
t416 = -t395;
t435 = -t408;
t449 = t230+t253;
t451 = t231+t254;
t466 = -t443;
t468 = -t448;
t470 = -t455;
t471 = -t456;
t475 = -t467;
t476 = t132.*t341;
t477 = -t469;
t484 = t170.*t341;
t526 = t276+t307;
t527 = (t12.*t25.*t397)./5.0e+3;
t528 = (t6.*t29.*t397)./5.0e+3;
t530 = (t12.*t29.*t397)./5.0e+3;
t531 = (t12.*t29.*t398)./5.0e+3;
t540 = (t12.*t25.*t397)./1.0e+4;
t541 = (t6.*t29.*t397)./1.0e+4;
t544 = (t12.*t29.*t398)./1.0e+4;
t551 = (t26.*t29.*t397)./5.0e+3;
t552 = (t29.*t30.*t397)./5.0e+3;
t557 = t8.*t518;
t567 = -t546;
t598 = (t132.*t397)./5.0e+3;
t599 = (t133.*t397)./5.0e+3;
t600 = (t132.*t398)./5.0e+3;
t607 = (t12.*t25.*t486)./5.0e+3;
t608 = (t6.*t29.*t486)./5.0e+3;
t609 = (t12.*t29.*t486)./5.0e+3;
t610 = (t170.*t397)./5.0e+3;
t611 = (t171.*t397)./5.0e+3;
t612 = (t171.*t398)./5.0e+3;
t617 = t247.*8.084033333333334e-4;
t623 = (t12.*t25.*t486)./1.0e+4;
t625 = t250+t419;
t631 = (t26.*t29.*t486)./5.0e+3;
t633 = (t29.*t30.*t486)./5.0e+3;
t658 = t350+t381;
t681 = (t132.*t486)./5.0e+3;
t682 = (t133.*t486)./5.0e+3;
t691 = (t170.*t486)./5.0e+3;
t692 = (t171.*t486)./5.0e+3;
t695 = t685./2.0;
t703 = (t12.*t25.*t624)./5.0e+3;
t704 = (t6.*t29.*t624)./5.0e+3;
t705 = (t12.*t29.*t622)./5.0e+3;
t706 = (t12.*t29.*t624)./5.0e+3;
t713 = (t12.*t25.*t624)./1.0e+4;
t715 = t25.*t686;
t717 = t29.*t686;
t725 = (t26.*t29.*t624)./5.0e+3;
t728 = (t29.*t30.*t624)./5.0e+3;
t746 = t8.*t716;
t749 = t8.*t718;
t751 = -t718;
t762 = t2.*t733;
t764 = t12.*t39.*t341.*8.084033333333334e-4;
t766 = t2.*t736;
t775 = (t12.*t29.*t678)./5.0e+3;
t778 = (t12.*t29.*t678)./1.0e+4;
t782 = (t132.*t622)./5.0e+3;
t783 = (t132.*t624)./5.0e+3;
t784 = (t133.*t624)./5.0e+3;
t789 = t425+t454;
t790 = t428+t457;
t798 = t6.*t25.*t398.*6.077704166666666e-4;
t799 = t6.*t25.*t398.*1.215540833333333e-3;
t801 = t6.*t29.*t397.*5.077704166666666e-4;
t802 = t6.*t29.*t397.*1.015540833333333e-3;
t803 = t6.*t29.*t398.*1.215540833333333e-3;
t804 = (t171.*t622)./5.0e+3;
Y = ft_2({qd1,qd2,qd3,qd4,qd5,qd6,qdd1,qdd2,qdd3,qdd4,qdd5,qdd6,t1001,t1002,t1006,t1009,t101,t1011,t1012,t1013,t1021,t1027,t1028,t1030,t1031,t1036,t1038,t1039,t1040,t1041,t1047,t1049,t1052,t1053,t1054,t1057,t1072,t1073,t1079,t108,t1080,t1081,t1088,t1089,t109,t1091,t1093,t1102,t111,t1116,t1124,t1125,t1129,t1131,t1132,t1133,t1137,t1138,t1139,t1140,t1141,t1152,t1155,t116,t1166,t1168,t1169,t1170,t1176,t1181,t1183,t1184,t12,t1200,t1207,t1208,t1212,t1213,t1214,t1215,t1220,t1246,t1247,t1268,t127,t1270,t1287,t1292,t13,t130,t1304,t1306,t132,t133,t1337,t1338,t1339,t1340,t1341,t1342,t1348,t1350,t1392,t1393,t1395,t1396,t1402,t1406,t1407,t1409,t144,t1440,t1441,t1448,t1449,t1454,t1458,t146,t1465,t1468,t1476,t1478,t1493,t1494,t15,t1506,t151,t1512,t1566,t157,t162,t163,t1675,t1677,t169,t17,t170,t171,t172,t177,t178,t179,t18,t190,t192,t193,t198,t2,t20,t211,t212,t213,t214,t219,t22,t220,t225,t227,t228,t229,t235,t236,t237,t239,t24,t241,t242,t243,t246,t248,t249,t25,t251,t252,t255,t256,t257,t259,t26,t261,t264,t265,t266,t267,t268,t269,t27,t270,t271,t274,t275,t277,t287,t289,t29,t291,t292,t293,t294,t296,t297,t299,t3,t30,t300,t302,t303,t31,t312,t313,t314,t316,t318,t319,t323,t324,t325,t326,t328,t329,t330,t331,t333,t334,t335,t337,t341,t342,t343,t344,t345,t346,t347,t348,t349,t35,t351,t352,t353,t354,t355,t356,t36,t360,t361,t363,t364,t367,t368,t370,t371,t376,t377,t378,t380,t382,t383,t384,t385,t386,t387,t389,t39,t390,t391,t393,t396,t397,t398,t40,t400,t402,t405,t406,t407,t409,t411,t412,t413,t415,t416,t418,t419,t420,t421,t423,t426,t427,t429,t430,t432,t433,t435,t436,t439,t441,t442,t443,t444,t445,t447,t448,t449,t450,t451,t452,t453,t455,t458,t459,t460,t462,t464,t465,t466,t468,t470,t471,t472,t473,t475,t476,t477,t479,t480,t481,t482,t483,t484,t485,t486,t487,t491,t493,t494,t495,t496,t497,t498,t499,t502,t505,t506,t507,t508,t509,t510,t512,t513,t519,t520,t521,t522,t523,t525,t526,t527,t528,t529,t530,t531,t533,t536,t540,t541,t544,t545,t549,t551,t552,t555,t556,t557,t558,t559,t560,t561,t562,t563,t565,t567,t568,t570,t571,t572,t574,t575,t576,t577,t580,t581,t582,t583,t584,t585,t586,t587,t588,t589,t594,t595,t596,t597,t598,t599,t6,t60,t600,t601,t602,t605,t606,t607,t608,t609,t61,t610,t611,t612,t614,t616,t617,t619,t620,t622,t623,t624,t63,t631,t633,t634,t638,t639,t640,t641,t644,t647,t648,t650,t651,t652,t653,t655,t658,t661,t662,t663,t664,t665,t666,t667,t668,t669,t670,t671,t672,t673,t674,t676,t677,t678,t679,t68,t680,t681,t682,t683,t684,t685,t686,t691,t692,t693,t695,t696,t697,t698,t699,t7,t700,t701,t702,t703,t704,t705,t706,t708,t709,t71,t710,t711,t713,t714,t715,t716,t717,t718,t719,t723,t724,t725,t726,t727,t728,t730,t731,t732,t733,t735,t736,t738,t739,t740,t741,t742,t743,t744,t746,t747,t749,t75,t750,t751,t752,t753,t754,t755,t756,t757,t758,t760,t761,t762,t763,t764,t765,t766,t767,t768,t769,t770,t771,t772,t773,t774,t775,t776,t777,t778,t779,t780,t782,t783,t784,t785,t786,t787,t788,t789,t79,t790,t793,t794,t795,t796,t798,t799,t8,t800,t801,t802,t803,t804,t809,t810,t811,t820,t823,t824,t825,t826,t827,t828,t829,t830,t831,t832,t835,t836,t839,t842,t843,t846,t847,t848,t850,t855,t856,t857,t858,t862,t863,t864,t865,t866,t867,t868,t869,t873,t874,t875,t876,t880,t881,t882,t883,t884,t885,t887,t889,t890,t891,t895,t899,t9,t90,t901,t902,t904,t905,t906,t907,t908,t909,t913,t915,t916,t917,t918,t92,t920,t928,t929,t930,t931,t937,t94,t942,t947,t948,t949,t952,t953,t955,t956,t957,t958,t959,t960,t961,t962,t963,t964,t965,t966,t967,t968,t974,t975,t990,t992,t993,t994,t995});
end
function Y = ft_2(ct)
qd1 = ct{1};
qd2 = ct{2};
qd3 = ct{3};
qd4 = ct{4};
qd5 = ct{5};
qd6 = ct{6};
qdd1 = ct{7};
qdd2 = ct{8};
qdd3 = ct{9};
qdd4 = ct{10};
qdd5 = ct{11};
qdd6 = ct{12};
t1001 = ct{13};
t1002 = ct{14};
t1006 = ct{15};
t1009 = ct{16};
t101 = ct{17};
t1011 = ct{18};
t1012 = ct{19};
t1013 = ct{20};
t1021 = ct{21};
t1027 = ct{22};
t1028 = ct{23};
t1030 = ct{24};
t1031 = ct{25};
t1036 = ct{26};
t1038 = ct{27};
t1039 = ct{28};
t1040 = ct{29};
t1041 = ct{30};
t1047 = ct{31};
t1049 = ct{32};
t1052 = ct{33};
t1053 = ct{34};
t1054 = ct{35};
t1057 = ct{36};
t1072 = ct{37};
t1073 = ct{38};
t1079 = ct{39};
t108 = ct{40};
t1080 = ct{41};
t1081 = ct{42};
t1088 = ct{43};
t1089 = ct{44};
t109 = ct{45};
t1091 = ct{46};
t1093 = ct{47};
t1102 = ct{48};
t111 = ct{49};
t1116 = ct{50};
t1124 = ct{51};
t1125 = ct{52};
t1129 = ct{53};
t1131 = ct{54};
t1132 = ct{55};
t1133 = ct{56};
t1137 = ct{57};
t1138 = ct{58};
t1139 = ct{59};
t1140 = ct{60};
t1141 = ct{61};
t1152 = ct{62};
t1155 = ct{63};
t116 = ct{64};
t1166 = ct{65};
t1168 = ct{66};
t1169 = ct{67};
t1170 = ct{68};
t1176 = ct{69};
t1181 = ct{70};
t1183 = ct{71};
t1184 = ct{72};
t12 = ct{73};
t1200 = ct{74};
t1207 = ct{75};
t1208 = ct{76};
t1212 = ct{77};
t1213 = ct{78};
t1214 = ct{79};
t1215 = ct{80};
t1220 = ct{81};
t1246 = ct{82};
t1247 = ct{83};
t1268 = ct{84};
t127 = ct{85};
t1270 = ct{86};
t1287 = ct{87};
t1292 = ct{88};
t13 = ct{89};
t130 = ct{90};
t1304 = ct{91};
t1306 = ct{92};
t132 = ct{93};
t133 = ct{94};
t1337 = ct{95};
t1338 = ct{96};
t1339 = ct{97};
t1340 = ct{98};
t1341 = ct{99};
t1342 = ct{100};
t1348 = ct{101};
t1350 = ct{102};
t1392 = ct{103};
t1393 = ct{104};
t1395 = ct{105};
t1396 = ct{106};
t1402 = ct{107};
t1406 = ct{108};
t1407 = ct{109};
t1409 = ct{110};
t144 = ct{111};
t1440 = ct{112};
t1441 = ct{113};
t1448 = ct{114};
t1449 = ct{115};
t1454 = ct{116};
t1458 = ct{117};
t146 = ct{118};
t1465 = ct{119};
t1468 = ct{120};
t1476 = ct{121};
t1478 = ct{122};
t1493 = ct{123};
t1494 = ct{124};
t15 = ct{125};
t1506 = ct{126};
t151 = ct{127};
t1512 = ct{128};
t1566 = ct{129};
t157 = ct{130};
t162 = ct{131};
t163 = ct{132};
t1675 = ct{133};
t1677 = ct{134};
t169 = ct{135};
t17 = ct{136};
t170 = ct{137};
t171 = ct{138};
t172 = ct{139};
t177 = ct{140};
t178 = ct{141};
t179 = ct{142};
t18 = ct{143};
t190 = ct{144};
t192 = ct{145};
t193 = ct{146};
t198 = ct{147};
t2 = ct{148};
t20 = ct{149};
t211 = ct{150};
t212 = ct{151};
t213 = ct{152};
t214 = ct{153};
t219 = ct{154};
t22 = ct{155};
t220 = ct{156};
t225 = ct{157};
t227 = ct{158};
t228 = ct{159};
t229 = ct{160};
t235 = ct{161};
t236 = ct{162};
t237 = ct{163};
t239 = ct{164};
t24 = ct{165};
t241 = ct{166};
t242 = ct{167};
t243 = ct{168};
t246 = ct{169};
t248 = ct{170};
t249 = ct{171};
t25 = ct{172};
t251 = ct{173};
t252 = ct{174};
t255 = ct{175};
t256 = ct{176};
t257 = ct{177};
t259 = ct{178};
t26 = ct{179};
t261 = ct{180};
t264 = ct{181};
t265 = ct{182};
t266 = ct{183};
t267 = ct{184};
t268 = ct{185};
t269 = ct{186};
t27 = ct{187};
t270 = ct{188};
t271 = ct{189};
t274 = ct{190};
t275 = ct{191};
t277 = ct{192};
t287 = ct{193};
t289 = ct{194};
t29 = ct{195};
t291 = ct{196};
t292 = ct{197};
t293 = ct{198};
t294 = ct{199};
t296 = ct{200};
t297 = ct{201};
t299 = ct{202};
t3 = ct{203};
t30 = ct{204};
t300 = ct{205};
t302 = ct{206};
t303 = ct{207};
t31 = ct{208};
t312 = ct{209};
t313 = ct{210};
t314 = ct{211};
t316 = ct{212};
t318 = ct{213};
t319 = ct{214};
t323 = ct{215};
t324 = ct{216};
t325 = ct{217};
t326 = ct{218};
t328 = ct{219};
t329 = ct{220};
t330 = ct{221};
t331 = ct{222};
t333 = ct{223};
t334 = ct{224};
t335 = ct{225};
t337 = ct{226};
t341 = ct{227};
t342 = ct{228};
t343 = ct{229};
t344 = ct{230};
t345 = ct{231};
t346 = ct{232};
t347 = ct{233};
t348 = ct{234};
t349 = ct{235};
t35 = ct{236};
t351 = ct{237};
t352 = ct{238};
t353 = ct{239};
t354 = ct{240};
t355 = ct{241};
t356 = ct{242};
t36 = ct{243};
t360 = ct{244};
t361 = ct{245};
t363 = ct{246};
t364 = ct{247};
t367 = ct{248};
t368 = ct{249};
t370 = ct{250};
t371 = ct{251};
t376 = ct{252};
t377 = ct{253};
t378 = ct{254};
t380 = ct{255};
t382 = ct{256};
t383 = ct{257};
t384 = ct{258};
t385 = ct{259};
t386 = ct{260};
t387 = ct{261};
t389 = ct{262};
t39 = ct{263};
t390 = ct{264};
t391 = ct{265};
t393 = ct{266};
t396 = ct{267};
t397 = ct{268};
t398 = ct{269};
t40 = ct{270};
t400 = ct{271};
t402 = ct{272};
t405 = ct{273};
t406 = ct{274};
t407 = ct{275};
t409 = ct{276};
t411 = ct{277};
t412 = ct{278};
t413 = ct{279};
t415 = ct{280};
t416 = ct{281};
t418 = ct{282};
t419 = ct{283};
t420 = ct{284};
t421 = ct{285};
t423 = ct{286};
t426 = ct{287};
t427 = ct{288};
t429 = ct{289};
t430 = ct{290};
t432 = ct{291};
t433 = ct{292};
t435 = ct{293};
t436 = ct{294};
t439 = ct{295};
t441 = ct{296};
t442 = ct{297};
t443 = ct{298};
t444 = ct{299};
t445 = ct{300};
t447 = ct{301};
t448 = ct{302};
t449 = ct{303};
t450 = ct{304};
t451 = ct{305};
t452 = ct{306};
t453 = ct{307};
t455 = ct{308};
t458 = ct{309};
t459 = ct{310};
t460 = ct{311};
t462 = ct{312};
t464 = ct{313};
t465 = ct{314};
t466 = ct{315};
t468 = ct{316};
t470 = ct{317};
t471 = ct{318};
t472 = ct{319};
t473 = ct{320};
t475 = ct{321};
t476 = ct{322};
t477 = ct{323};
t479 = ct{324};
t480 = ct{325};
t481 = ct{326};
t482 = ct{327};
t483 = ct{328};
t484 = ct{329};
t485 = ct{330};
t486 = ct{331};
t487 = ct{332};
t491 = ct{333};
t493 = ct{334};
t494 = ct{335};
t495 = ct{336};
t496 = ct{337};
t497 = ct{338};
t498 = ct{339};
t499 = ct{340};
t502 = ct{341};
t505 = ct{342};
t506 = ct{343};
t507 = ct{344};
t508 = ct{345};
t509 = ct{346};
t510 = ct{347};
t512 = ct{348};
t513 = ct{349};
t519 = ct{350};
t520 = ct{351};
t521 = ct{352};
t522 = ct{353};
t523 = ct{354};
t525 = ct{355};
t526 = ct{356};
t527 = ct{357};
t528 = ct{358};
t529 = ct{359};
t530 = ct{360};
t531 = ct{361};
t533 = ct{362};
t536 = ct{363};
t540 = ct{364};
t541 = ct{365};
t544 = ct{366};
t545 = ct{367};
t549 = ct{368};
t551 = ct{369};
t552 = ct{370};
t555 = ct{371};
t556 = ct{372};
t557 = ct{373};
t558 = ct{374};
t559 = ct{375};
t560 = ct{376};
t561 = ct{377};
t562 = ct{378};
t563 = ct{379};
t565 = ct{380};
t567 = ct{381};
t568 = ct{382};
t570 = ct{383};
t571 = ct{384};
t572 = ct{385};
t574 = ct{386};
t575 = ct{387};
t576 = ct{388};
t577 = ct{389};
t580 = ct{390};
t581 = ct{391};
t582 = ct{392};
t583 = ct{393};
t584 = ct{394};
t585 = ct{395};
t586 = ct{396};
t587 = ct{397};
t588 = ct{398};
t589 = ct{399};
t594 = ct{400};
t595 = ct{401};
t596 = ct{402};
t597 = ct{403};
t598 = ct{404};
t599 = ct{405};
t6 = ct{406};
t60 = ct{407};
t600 = ct{408};
t601 = ct{409};
t602 = ct{410};
t605 = ct{411};
t606 = ct{412};
t607 = ct{413};
t608 = ct{414};
t609 = ct{415};
t61 = ct{416};
t610 = ct{417};
t611 = ct{418};
t612 = ct{419};
t614 = ct{420};
t616 = ct{421};
t617 = ct{422};
t619 = ct{423};
t620 = ct{424};
t622 = ct{425};
t623 = ct{426};
t624 = ct{427};
t63 = ct{428};
t631 = ct{429};
t633 = ct{430};
t634 = ct{431};
t638 = ct{432};
t639 = ct{433};
t640 = ct{434};
t641 = ct{435};
t644 = ct{436};
t647 = ct{437};
t648 = ct{438};
t650 = ct{439};
t651 = ct{440};
t652 = ct{441};
t653 = ct{442};
t655 = ct{443};
t658 = ct{444};
t661 = ct{445};
t662 = ct{446};
t663 = ct{447};
t664 = ct{448};
t665 = ct{449};
t666 = ct{450};
t667 = ct{451};
t668 = ct{452};
t669 = ct{453};
t670 = ct{454};
t671 = ct{455};
t672 = ct{456};
t673 = ct{457};
t674 = ct{458};
t676 = ct{459};
t677 = ct{460};
t678 = ct{461};
t679 = ct{462};
t68 = ct{463};
t680 = ct{464};
t681 = ct{465};
t682 = ct{466};
t683 = ct{467};
t684 = ct{468};
t685 = ct{469};
t686 = ct{470};
t691 = ct{471};
t692 = ct{472};
t693 = ct{473};
t695 = ct{474};
t696 = ct{475};
t697 = ct{476};
t698 = ct{477};
t699 = ct{478};
t7 = ct{479};
t700 = ct{480};
t701 = ct{481};
t702 = ct{482};
t703 = ct{483};
t704 = ct{484};
t705 = ct{485};
t706 = ct{486};
t708 = ct{487};
t709 = ct{488};
t71 = ct{489};
t710 = ct{490};
t711 = ct{491};
t713 = ct{492};
t714 = ct{493};
t715 = ct{494};
t716 = ct{495};
t717 = ct{496};
t718 = ct{497};
t719 = ct{498};
t723 = ct{499};
t724 = ct{500};
t725 = ct{501};
t726 = ct{502};
t727 = ct{503};
t728 = ct{504};
t730 = ct{505};
t731 = ct{506};
t732 = ct{507};
t733 = ct{508};
t735 = ct{509};
t736 = ct{510};
t738 = ct{511};
t739 = ct{512};
t740 = ct{513};
t741 = ct{514};
t742 = ct{515};
t743 = ct{516};
t744 = ct{517};
t746 = ct{518};
t747 = ct{519};
t749 = ct{520};
t75 = ct{521};
t750 = ct{522};
t751 = ct{523};
t752 = ct{524};
t753 = ct{525};
t754 = ct{526};
t755 = ct{527};
t756 = ct{528};
t757 = ct{529};
t758 = ct{530};
t760 = ct{531};
t761 = ct{532};
t762 = ct{533};
t763 = ct{534};
t764 = ct{535};
t765 = ct{536};
t766 = ct{537};
t767 = ct{538};
t768 = ct{539};
t769 = ct{540};
t770 = ct{541};
t771 = ct{542};
t772 = ct{543};
t773 = ct{544};
t774 = ct{545};
t775 = ct{546};
t776 = ct{547};
t777 = ct{548};
t778 = ct{549};
t779 = ct{550};
t780 = ct{551};
t782 = ct{552};
t783 = ct{553};
t784 = ct{554};
t785 = ct{555};
t786 = ct{556};
t787 = ct{557};
t788 = ct{558};
t789 = ct{559};
t79 = ct{560};
t790 = ct{561};
t793 = ct{562};
t794 = ct{563};
t795 = ct{564};
t796 = ct{565};
t798 = ct{566};
t799 = ct{567};
t8 = ct{568};
t800 = ct{569};
t801 = ct{570};
t802 = ct{571};
t803 = ct{572};
t804 = ct{573};
t809 = ct{574};
t810 = ct{575};
t811 = ct{576};
t820 = ct{577};
t823 = ct{578};
t824 = ct{579};
t825 = ct{580};
t826 = ct{581};
t827 = ct{582};
t828 = ct{583};
t829 = ct{584};
t830 = ct{585};
t831 = ct{586};
t832 = ct{587};
t835 = ct{588};
t836 = ct{589};
t839 = ct{590};
t842 = ct{591};
t843 = ct{592};
t846 = ct{593};
t847 = ct{594};
t848 = ct{595};
t850 = ct{596};
t855 = ct{597};
t856 = ct{598};
t857 = ct{599};
t858 = ct{600};
t862 = ct{601};
t863 = ct{602};
t864 = ct{603};
t865 = ct{604};
t866 = ct{605};
t867 = ct{606};
t868 = ct{607};
t869 = ct{608};
t873 = ct{609};
t874 = ct{610};
t875 = ct{611};
t876 = ct{612};
t880 = ct{613};
t881 = ct{614};
t882 = ct{615};
t883 = ct{616};
t884 = ct{617};
t885 = ct{618};
t887 = ct{619};
t889 = ct{620};
t890 = ct{621};
t891 = ct{622};
t895 = ct{623};
t899 = ct{624};
t9 = ct{625};
t90 = ct{626};
t901 = ct{627};
t902 = ct{628};
t904 = ct{629};
t905 = ct{630};
t906 = ct{631};
t907 = ct{632};
t908 = ct{633};
t909 = ct{634};
t913 = ct{635};
t915 = ct{636};
t916 = ct{637};
t917 = ct{638};
t918 = ct{639};
t92 = ct{640};
t920 = ct{641};
t928 = ct{642};
t929 = ct{643};
t930 = ct{644};
t931 = ct{645};
t937 = ct{646};
t94 = ct{647};
t942 = ct{648};
t947 = ct{649};
t948 = ct{650};
t949 = ct{651};
t952 = ct{652};
t953 = ct{653};
t955 = ct{654};
t956 = ct{655};
t957 = ct{656};
t958 = ct{657};
t959 = ct{658};
t960 = ct{659};
t961 = ct{660};
t962 = ct{661};
t963 = ct{662};
t964 = ct{663};
t965 = ct{664};
t966 = ct{665};
t967 = ct{666};
t968 = ct{667};
t974 = ct{668};
t975 = ct{669};
t990 = ct{670};
t992 = ct{671};
t993 = ct{672};
t994 = ct{673};
t995 = ct{674};
t805 = t12.*t29.*t398.*5.077704166666666e-4;
t806 = t12.*t29.*t398.*1.015540833333333e-3;
t807 = (t170.*t624)./5.0e+3;
t808 = (t171.*t624)./5.0e+3;
t818 = t787./2.0;
t819 = -t810;
t821 = t24.*t29.*t398.*1.215540833333333e-3;
t822 = t27.*t29.*t398.*1.215540833333333e-3;
t834 = t192.*t341.*8.084033333333334e-4;
t837 = -t825;
t838 = -t827;
t845 = t8.*t823;
t849 = t237.*t341.*8.084033333333334e-4;
t851 = t2.*t820;
t852 = (t132.*t678)./5.0e+3;
t871 = (t171.*t678)./5.0e+3;
t872 = -t856;
t877 = t133.*t397.*1.015540833333333e-3;
t878 = t132.*t398.*1.015540833333333e-3;
t879 = t133.*t398.*1.215540833333333e-3;
t888 = (t12.*t29.*t774)./5.0e+3;
t892 = t170.*t397.*1.015540833333333e-3;
t893 = t170.*t398.*1.215540833333333e-3;
t894 = t171.*t398.*1.015540833333333e-3;
t897 = -t880;
t898 = t875./2.0;
t900 = t880./2.0;
t903 = t882./2.0;
t911 = -t907;
t912 = -t908;
t914 = t418+t582;
t919 = (t8.*t361.*t602)./2.0;
t924 = t2.*t361.*(t241-t419).*(-1.0./2.0);
t934 = (t132.*t774)./5.0e+3;
t935 = t291+t383+t439;
t936 = t2.*t920;
t941 = (t171.*t774)./5.0e+3;
t943 = t523+t556;
t954 = -t949;
t969 = t6.*t25.*t622.*6.077704166666666e-4;
t970 = t6.*t25.*t622.*1.215540833333333e-3;
t971 = t6.*t29.*t622.*1.215540833333333e-3;
t972 = t6.*t29.*t624.*1.015540833333333e-3;
t973 = t12.*t29.*t622.*1.015540833333333e-3;
t976 = -t957;
t979 = (t12.*t29.*t901)./5.0e+3;
t981 = t565+t572;
t983 = (t12.*t29.*t901)./1.0e+4;
t984 = t24.*t29.*t622.*1.215540833333333e-3;
t985 = t27.*t29.*t622.*1.215540833333333e-3;
t987 = t562+t570;
t988 = t563+t571;
t989 = t967./2.0;
t1003 = (t8.*t479.*t602)./2.0;
t1004 = t132.*t913;
t1010 = t94+t157+t172+t686;
t1014 = -t1002;
t1015 = t2.*t479.*(t241-t419).*(-1.0./2.0);
t1023 = t171.*t913;
t1024 = t132.*t622.*1.015540833333333e-3;
t1025 = t133.*t622.*1.215540833333333e-3;
t1026 = t133.*t624.*1.015540833333333e-3;
t1029 = -t1012;
t1035 = t2.*t1011;
t1037 = (t132.*t901)./5.0e+3;
t1042 = t170.*t622.*1.215540833333333e-3;
t1043 = t171.*t622.*1.015540833333333e-3;
t1044 = t170.*t624.*1.015540833333333e-3;
t1045 = t447+t716;
t1046 = t8.*t1021;
t1051 = (t171.*t901)./5.0e+3;
t1056 = -t1047;
t1062 = t1049./2.0;
t1063 = -t1054;
t1065 = (t8.*t580.*t602)./2.0;
t1070 = t1054./2.0;
t1078 = t2.*t580.*(t241-t419).*(-1.0./2.0);
t1083 = t192.*t665.*8.084033333333334e-4;
t1097 = t616+t648;
t1100 = t90+t1011;
t1101 = t75+t1021;
t1103 = t236.*t666.*8.084033333333334e-4;
t1106 = t2.*t1088;
t1107 = t2.*t1089;
t1108 = t634+t644;
t1110 = t8.*t1079;
t1111 = t8.*t1080;
t1123 = t8.*t1102;
t1128 = t650+t655;
t1135 = t1125./2.0;
t1142 = t325.*t666.*8.084033333333334e-4;
t1143 = t1132./2.0;
t1146 = -t1137;
t1147 = t29.*t111.*t1036;
t1148 = t24.*t29.*t1036.*2.8925e-2;
t1149 = t665.*(t60-t190).*(-8.084033333333334e-4);
t1150 = t341.*t665.*8.084033333333334e-4;
t1151 = t1137./2.0;
t1153 = -t29.*t116.*(t423-t716);
t1154 = t27.*t29.*(t423-t716).*(-2.8925e-2);
t1156 = t1141./2.0;
t1161 = t27.*t29.*(t423-t716).*2.8925e-2;
t1162 = t676+t680;
t1163 = t666.*(t61-t239).*(-8.084033333333334e-4);
t1165 = t683+t684;
t1173 = t6.*t29.*t899.*6.077704166666666e-4;
t1174 = t6.*t29.*t899.*1.215540833333333e-3;
t1180 = t1168./2.0;
t1182 = t1170./2.0;
t1189 = t29.*t111.*t1102;
t1190 = t24.*t29.*t1102.*2.8925e-2;
t1197 = t24.*t29.*t1102.*(-5.785e-2);
t1204 = t2.*t1184;
t1205 = t8.*t1183;
t1225 = -t1214;
t1227 = t1208./2.0;
t1228 = t1212./2.0;
t1229 = t1213./2.0;
t1230 = t1214./2.0;
t1231 = t133.*t899.*1.215540833333333e-3;
t1235 = t2.*t25.*t1183;
t1238 = t8.*t25.*t1184;
t1239 = t2.*t361.*t1036;
t1241 = t303+t1102;
t1242 = t169+t671+t677;
t1243 = t170.*t899.*1.215540833333333e-3;
t1244 = -t8.*t361.*(t423-t716);
t1245 = t2.*t368.*t1036;
t1248 = -t8.*t368.*(t423-t716);
t1256 = t371.*(t423-t716).*(-1.0./2.0);
t1259 = (t380.*t1036)./2.0;
t1260 = t8.*t368.*(t423-t716);
t1262 = t1246./2.0;
t1265 = t1247./2.0;
t1266 = t460+t1001;
t1274 = t741+t769;
t1284 = t1268./2.0;
t1286 = t1270./2.0;
t1294 = -t1287;
t1299 = t2.*t361.*t1102;
t1307 = t2.*t368.*t1102;
t1314 = t733+t842;
t1315 = t1304./2.0;
t1317 = t1306./2.0;
t1319 = t2.*t479.*t1036;
t1322 = -t8.*t479.*(t423-t716);
t1323 = t2.*t481.*t1036;
t1325 = -t8.*t481.*(t423-t716);
t1333 = t8.*t481.*(t423-t716).*(-1.0./2.0);
t1343 = -t1340;
t1344 = -t1342;
t1346 = t402.*t1138;
t1349 = t577.*t1036;
t1351 = -t575.*(t423-t716);
t1353 = t2.*t479.*t1102;
t1354 = t242+t756+t758;
t1356 = t2.*t580.*t1036;
t1360 = -t8.*t580.*(t423-t716);
t1363 = t2.*t481.*t1102;
t1364 = t575.*(t423-t716).*(-1.0./2.0);
t1377 = (t2.*t581.*t1036)./2.0;
t1387 = t8.*t581.*(t423-t716).*(-1.0./2.0);
t1401 = (t8.*t773.*t902)./2.0;
t1405 = t15.*t773.*t904;
t1408 = t17.*t773.*t904;
t1410 = t864+t867;
t1411 = t865+t868;
t1415 = t863+t866;
t1423 = t2.*t580.*t1102;
t1424 = t1402./2.0;
t1427 = t1406./2.0;
t1428 = t1407./2.0;
t1430 = t1409./2.0;
t1443 = (t2.*t581.*t1102)./2.0;
t1445 = -t1440;
t1459 = -t378.*(t426-t1001);
t1461 = t1102.*(t241-t419).*(-1.0./2.0);
t1462 = -t370.*(t443-t1013);
t1463 = t1454./2.0;
t1467 = (t15.*t773.*t953)./2.0;
t1469 = (t17.*t773.*t953)./2.0;
t1470 = t1458./2.0;
t1471 = t378.*(t426-t1001).*(-1.0./2.0);
t1475 = (t8.*t890.*t902)./2.0;
t1481 = t370.*(t443-t1013).*(-1.0./2.0);
t1482 = t1465./2.0;
t1483 = t1468./2.0;
t1487 = t1476./2.0;
t1489 = t1478./2.0;
t1495 = t928+t930;
t1496 = t929+t931;
t1499 = t829.*t1036;
t1500 = (t8.*t902.*t942)./2.0;
t1501 = t337+t832+t843;
t1502 = -t836.*(t423-t716);
t1504 = -t2.*t491.*(t426-t1001);
t1507 = (t17.*t904.*t942)./2.0;
t1513 = (t15.*t890.*t953)./2.0;
t1514 = (t15.*t904.*t942)./2.0;
t1515 = (t17.*t890.*t953)./2.0;
t1517 = -t1512;
t1519 = t836.*(t423-t716).*(-1.0./2.0);
t1520 = t2.*t491.*(t426-t1001).*(-1.0./2.0);
t1521 = -t8.*t491.*(t443-t1013);
t1527 = t8.*t491.*(t443-t1013).*(-1.0./2.0);
t1528 = -t576.*(t426-t1001);
t1532 = t958+t961;
t1534 = t959+t963;
t1535 = t960+t964;
t1536 = -t574.*(t443-t1013);
t1538 = t576.*(t426-t1001).*(-1.0./2.0);
t1543 = t918.*t1036;
t1551 = -t916.*(t423-t716);
t1552 = t574.*(t443-t1013).*(-1.0./2.0);
t1565 = t916.*(t423-t716).*(-1.0./2.0);
t1590 = t1027+t1028;
t1610 = -t2.*t773.*(t426-t1001);
t1614 = -t2.*t785.*(t426-t1001);
t1616 = -t8.*t773.*(t443-t1013);
t1617 = t2.*t785.*(t426-t1001).*(-1.0./2.0);
t1618 = -t8.*t785.*(t443-t1013);
t1619 = -t828.*(t426-t1001);
t1620 = t1036.*t1102;
t1625 = t8.*t785.*(t443-t1013).*(-1.0./2.0);
t1626 = -t835.*(t443-t1013);
t1628 = t828.*(t426-t1001).*(-1.0./2.0);
t1632 = t835.*(t443-t1013).*(-1.0./2.0);
t1635 = t236.*(-t267-t293+t348+t352+t382+t8.*t25.*(t61-t239)).*(-4.042016666666667e-4);
t1636 = t236.*(-t267-t293+t348+t352+t382+t8.*t25.*(t61-t239)).*(-8.084033333333334e-4);
t1642 = -t2.*t890.*(t426-t1001);
t1647 = -t2.*t904.*(t426-t1001);
t1651 = -t917.*(t426-t1001);
t1653 = -t8.*t890.*(t443-t1013);
t1656 = t2.*t361.*t1566;
t1659 = -t8.*t361.*(t421-t432-t619+t718);
t1662 = t2.*t904.*(t426-t1001).*(-1.0./2.0);
t1663 = -t8.*t904.*(t443-t1013);
t1664 = t902.*(t443-t1013).*(-1.0./2.0);
t1666 = -t915.*(t443-t1013);
t1667 = t325.*(-t267-t293+t348+t352+t382+t8.*t25.*(t61-t239)).*(-8.084033333333334e-4);
t1670 = t917.*(t426-t1001).*(-1.0./2.0);
t1671 = t325.*(-t267-t293+t348+t352+t382+t8.*t25.*(t61-t239)).*8.084033333333334e-4;
t1673 = t8.*t361.*(t421-t432-t619+t718).*(-1.0./2.0);
t1676 = t8.*t904.*(t443-t1013).*(-1.0./2.0);
t1678 = t915.*(t443-t1013).*(-1.0./2.0);
t1682 = (t61-t239).*(-t267-t293+t348+t352+t382+t8.*t25.*(t61-t239)).*8.084033333333334e-4;
t1683 = -t2.*t942.*(t426-t1001);
t1686 = t8.*t1675;
t1687 = t2.*t1677;
t1700 = -t8.*t942.*(t443-t1013);
t1710 = t2.*t953.*(t426-t1001).*(-1.0./2.0);
t1714 = t2.*t29.*t1675;
t1716 = t8.*t29.*t1677;
t1719 = t8.*t953.*(t443-t1013).*(-1.0./2.0);
t1720 = t2.*t479.*t1566;
t1723 = -t8.*t479.*(t421-t432-t619+t718);
t1730 = t8.*t479.*(t421-t432-t619+t718).*(-1.0./2.0);
t1734 = (t8.*t479.*(t421-t432-t619+t718))./2.0;
t1746 = t2.*t580.*t1566;
t1747 = -t8.*t580.*(t421-t432-t619+t718);
t1756 = t8.*t580.*(t421-t432-t619+t718).*(-1.0./2.0);
t1763 = (t8.*t580.*(t421-t432-t619+t718))./2.0;
t1828 = t1036.*t1566;
t1839 = (t423-t716).*(t421-t432-t619+t718);
t1863 = t1102.*t1566;
t1867 = -t2.*t773.*(t441-t442-t647+t1012);
t1879 = t2.*t773.*(t441-t442-t647+t1012).*(-1.0./2.0);
t1895 = -t2.*t890.*(t441-t442-t647+t1012);
t1897 = t2.*t890.*(t441-t442-t647+t1012).*(-1.0./2.0);
t1903 = t330+t344+t731+t747+t761+t765;
t1908 = -t8.*(t324-t344+t730-t731-t765+t12.*t39.*(t60-t190).*8.084033333333334e-4);
t1910 = -t2.*t942.*(t441-t442-t647+t1012);
t1917 = t8.*(t324-t344+t730-t731-t765+t12.*t39.*(t60-t190).*8.084033333333334e-4).*(-1.0./2.0);
t1919 = t2.*t942.*(t441-t442-t647+t1012).*(-1.0./2.0);
t414 = -t393;
t504 = -t484;
t539 = -t527;
t542 = -t530;
t543 = -t531;
t553 = -t540;
t554 = -t544;
t564 = -t551;
t566 = -t552;
t569 = t302+t326;
t573 = -t557;
t603 = -t599;
t604 = -t600;
t626 = -t610;
t627 = -t612;
t645 = -t633;
t659 = t363+t364;
t688 = -t682;
t694 = -t691;
t712 = -t703;
t721 = t385+t415;
t722 = t386+t416;
t729 = -t713;
t745 = t8.*t715;
t748 = t8.*t717;
t791 = -t783;
t792 = -t784;
t812 = t433+t468;
t813 = -t799;
t814 = -t798;
t815 = -t801;
t816 = -t806;
t817 = -t807;
t844 = -t834;
t861 = -t849;
t896 = -t888;
t921 = t192.*t449.*4.042016666666667e-4;
t922 = t192.*t449.*8.084033333333334e-4;
t923 = t266+t396+t411;
t932 = t236.*t451.*4.042016666666667e-4;
t933 = t236.*t451.*8.084033333333334e-4;
t938 = -t934;
t946 = -t936;
t950 = -t941;
t977 = t192.*t526.*4.042016666666667e-4;
t978 = t192.*t526.*8.084033333333334e-4;
t982 = -t979;
t986 = t325.*t451.*8.084033333333334e-4;
t991 = -t983;
t996 = t449.*(t60-t190).*(-8.084033333333334e-4);
t997 = t341.*t449.*8.084033333333334e-4;
t998 = qd3.*t987;
t999 = qd1.*t988;
t1000 = qd3.*t988;
t1005 = t451.*(t61-t239).*(-8.084033333333334e-4);
t1018 = t12.*t40.*t658.*4.042016666666667e-4;
t1019 = t12.*t40.*t658.*8.084033333333334e-4;
t1032 = -t1025;
t1033 = -t1026;
t1034 = t2.*t1010;
t1048 = -t1037;
t1050 = -t1044;
t1055 = -t1046;
t1058 = t526.*(t60-t190).*(-8.084033333333334e-4);
t1059 = t316+t473+t485;
t1060 = t318+t476+t482;
t1061 = t341.*t526.*8.084033333333334e-4;
t1064 = t526.*(t60-t190).*8.084033333333334e-4;
t1069 = t13.*t132.*t658.*8.084033333333334e-4;
t1074 = -t1070;
t1075 = t193.*t658.*4.042016666666667e-4;
t1076 = t193.*t658.*8.084033333333334e-4;
t1084 = t13.*t171.*t658.*8.084033333333334e-4;
t1092 = -t1083;
t1094 = t236.*t658.*8.084033333333334e-4;
t1099 = t90+t1010;
t1117 = t8.*t1097;
t1119 = t2.*t1100;
t1120 = t269.*t658.*8.084033333333334e-4;
t1121 = t270.*t658.*8.084033333333334e-4;
t1122 = t8.*t1101;
t1127 = -t1123;
t1136 = t325.*t658.*8.084033333333334e-4;
t1157 = -t1148;
t1158 = t658.*(t61-t239).*(-8.084033333333334e-4);
t1164 = t162+t601+t617;
t1178 = -t25.*(t530-t803);
t1179 = -t29.*(t530-t803);
t1186 = t29.*(t530-t803);
t1187 = t29.*t116.*t1100;
t1188 = t27.*t29.*t1100.*2.8925e-2;
t1195 = t27.*t29.*t1100.*(-5.785e-2);
t1198 = -t1190;
t1202 = t8.*(t551-t821).*(-1.0./2.0);
t1203 = t2.*(t552-t822).*(-1.0./2.0);
t1209 = (t8.*(t551-t821))./2.0;
t1211 = (t2.*(t552-t822))./2.0;
t1219 = -t2.*t29.*(t551-t821);
t1221 = -t1205;
t1222 = -t8.*t29.*(t552-t822);
t1226 = t12.*t40.*t935.*8.084033333333334e-4;
t1233 = t294+t1100;
t1234 = t2.*t29.*(t551-t821).*(-1.0./2.0);
t1236 = t8.*t29.*(t552-t822).*(-1.0./2.0);
t1237 = -t1231;
t1240 = t303+t1101;
t1251 = t1235./2.0;
t1252 = t1238./2.0;
t1253 = t598+t893;
t1254 = t611+t879;
t1255 = -t1245;
t1258 = t8.*t1241;
t1261 = t1245./2.0;
t1264 = t749+t767;
t1267 = t1260.*(-1.0./2.0);
t1275 = t1260./2.0;
t1281 = t13.*t132.*t935.*8.084033333333334e-4;
t1282 = t466+t1013;
t1283 = t376+t384+t472+t477;
t1288 = t193.*t935.*4.042016666666667e-4;
t1289 = t193.*t935.*8.084033333333334e-4;
t1293 = t13.*t171.*t935.*8.084033333333334e-4;
t1297 = t236.*t935.*8.084033333333334e-4;
t1298 = t8.*t361.*t1100;
t1305 = t8.*t368.*t1100;
t1310 = t269.*t935.*8.084033333333334e-4;
t1311 = t270.*t935.*8.084033333333334e-4;
t1318 = t1307./2.0;
t1321 = t715+t858;
t1327 = t12.*t39.*(t289-t476+t171.*(t60-t190)).*(-8.084033333333334e-4);
t1329 = t325.*t935.*8.084033333333334e-4;
t1332 = t1323./2.0;
t1347 = t935.*(t61-t239).*(-8.084033333333334e-4);
t1352 = -t1346;
t1355 = -t1349;
t1357 = t1346./2.0;
t1358 = t8.*t479.*t1100;
t1359 = t1349./2.0;
t1362 = t8.*t481.*t1100;
t1365 = t7.*t132.*(t289-t476+t171.*(t60-t190)).*(-8.084033333333334e-4);
t1369 = t2.*t491.*t1101;
t1371 = t101+t227+t248+t313+t475+t529;
t1372 = t192.*(t289-t476+t171.*(t60-t190)).*(-8.084033333333334e-4);
t1375 = t845+t851;
t1376 = t7.*t171.*(t289-t476+t171.*(t60-t190)).*(-8.084033333333334e-4);
t1381 = t192.*(t289-t476+t171.*(t60-t190)).*8.084033333333334e-4;
t1386 = t1363./2.0;
t1390 = t237.*(t289-t476+t171.*(t60-t190)).*(-4.042016666666667e-4);
t1391 = t237.*(t289-t476+t171.*(t60-t190)).*(-8.084033333333334e-4);
t1398 = t25.*t1354;
t1403 = t249.*(t289-t476+t171.*(t60-t190)).*(-8.084033333333334e-4);
t1404 = t252.*(t289-t476+t171.*(t60-t190)).*(-8.084033333333334e-4);
t1413 = t249.*(t289-t476+t171.*(t60-t190)).*8.084033333333334e-4;
t1414 = t12.*t29.*t1354;
t1420 = t8.*t580.*t1100;
t1422 = (t2.*t773.*t914)./2.0;
t1426 = t1405./2.0;
t1429 = t1408./2.0;
t1431 = qd4.*t1410;
t1432 = qd1.*t1411;
t1435 = -t1428;
t1437 = -t1430;
t1442 = (t8.*t581.*t1100)./2.0;
t1446 = t877+t894;
t1447 = t878+t892;
t1450 = (t60-t190).*(t289-t476+t171.*(t60-t190)).*8.084033333333334e-4;
t1451 = t341.*(t289-t476+t171.*(t60-t190)).*(-8.084033333333334e-4);
t1452 = (t602.*t1100)./2.0;
t1453 = t267+t293+t360+t367+t391+t413;
t1455 = (t789.*t943)./2.0;
t1472 = -t1463;
t1474 = -t1470;
t1480 = t402.*t1274;
t1486 = (t2.*t890.*t914)./2.0;
t1498 = (t378.*t1314)./2.0;
t1503 = t510+t533+t545+t567;
t1505 = -t1499;
t1508 = t1499./2.0;
t1511 = (t2.*t914.*t942)./2.0;
t1518 = t8.*t1501;
t1523 = t2.*t773.*t1101;
t1524 = -t2.*(t329+t834+t236.*(t61-t239).*8.084033333333334e-4);
t1526 = t2.*t785.*t1101;
t1529 = t287+t333+t407+t409+t412+t436;
t1530 = t2.*t25.*t1501;
t1539 = t26.*t29.*t1501;
t1542 = -t8.*t25.*(t329+t834+t236.*(t61-t239).*8.084033333333334e-4);
t1545 = t312+t319+t389+t430+t435+t462;
t1546 = t2.*t491.*t1314;
t1550 = -t29.*t30.*(t329+t834+t236.*(t61-t239).*8.084033333333334e-4);
t1553 = -t1543;
t1556 = t8.*t25.*(t329+t834+t236.*(t61-t239).*8.084033333333334e-4).*(-1.0./2.0);
t1557 = t1543./2.0;
t1564 = t29.*t30.*(t329+t834+t236.*(t61-t239).*8.084033333333334e-4).*(-1.0./2.0);
t1568 = t576.*t1314;
t1569 = t432+t445+t619+t751;
t1570 = t943.*t1040;
t1573 = t2.*t890.*t1101;
t1579 = t2.*t904.*t1101;
t1585 = (t914.*t1101)./2.0;
t1591 = t2.*t942.*t1101;
t1603 = t1035+t1056;
t1605 = (t2.*t953.*t1101)./2.0;
t1607 = -t8.*(t1026-t1043);
t1612 = t8.*(t1026-t1043);
t1621 = t192.*(-t268-t292+t331+t334+t393+t2.*t25.*(t60-t190)).*(-4.042016666666667e-4);
t1622 = t192.*(-t268-t292+t331+t334+t393+t2.*t25.*(t60-t190)).*(-8.084033333333334e-4);
t1623 = -t1100.*(t423-t716);
t1627 = -t402.*(t936-t937);
t1631 = t2.*t773.*t1314;
t1633 = t402.*(t936-t937).*(-1.0./2.0);
t1638 = (t402.*(t936-t937))./2.0;
t1639 = t2.*t785.*t1314;
t1641 = t828.*t1314;
t1648 = t1106+t1110;
t1649 = t1107+t1111;
t1654 = (t60-t190).*(-t268-t292+t331+t334+t393+t2.*t25.*(t60-t190)).*8.084033333333334e-4;
t1655 = t341.*(-t268-t292+t331+t334+t393+t2.*t25.*(t60-t190)).*(-8.084033333333334e-4);
t1658 = t706+t709+t971;
t1660 = t341.*(-t268-t292+t331+t334+t393+t2.*t25.*(t60-t190)).*8.084033333333334e-4;
t1665 = t914.*(t426-t1001).*(-1.0./2.0);
t1668 = -t1656;
t1672 = t1656./2.0;
t1685 = t2.*t890.*t1314;
t1689 = t943.*(t384+t472+t477+t26.*t29.*t132.*1.383e-1);
t1690 = (t1108.*t1138)./2.0;
Y = ft_3({qd1,qd2,qd3,qd4,qd5,qd6,qdd1,qdd2,qdd3,qdd4,qdd5,qdd6,t1000,t1001,t1003,t1004,t1005,t1006,t1009,t1012,t1013,t1014,t1015,t1018,t1019,t1023,t1024,t1026,t1029,t1030,t1031,t1032,t1033,t1034,t1036,t1038,t1039,t1040,t1041,t1042,t1043,t1048,t1049,t1050,t1051,t1052,t1053,t1054,t1055,t1057,t1059,t1061,t1062,t1064,t1065,t1069,t1070,t1072,t1073,t1074,t1075,t1076,t1078,t108,t1081,t1083,t1084,t109,t1091,t1092,t1093,t1094,t1097,t1099,t1100,t1101,t1102,t1103,t1108,t1116,t1117,t1119,t1120,t1121,t1122,t1124,t1125,t1127,t1128,t1129,t1131,t1132,t1133,t1135,t1136,t1138,t1139,t1140,t1141,t1142,t1143,t1146,t1147,t1148,t1149,t1150,t1151,t1152,t1153,t1154,t1155,t1156,t1157,t1158,t1161,t1162,t1163,t1164,t1165,t1166,t1168,t1169,t1170,t1173,t1174,t1176,t1178,t1179,t1180,t1181,t1182,t1183,t1184,t1186,t1187,t1188,t1189,t1190,t1198,t12,t1200,t1202,t1203,t1204,t1207,t1208,t1209,t1211,t1212,t1213,t1215,t1220,t1221,t1225,t1226,t1227,t1228,t1229,t1230,t1233,t1234,t1235,t1236,t1237,t1238,t1239,t1240,t1242,t1243,t1244,t1246,t1247,t1251,t1252,t1253,t1254,t1255,t1256,t1258,t1259,t1260,t1261,t1262,t1264,t1265,t1267,t1268,t127,t1270,t1274,t1275,t1281,t1284,t1286,t1288,t1289,t1292,t1293,t1294,t1297,t1298,t1299,t13,t130,t1304,t1305,t1306,t1307,t1310,t1311,t1314,t1315,t1317,t1318,t1319,t132,t1321,t1322,t1323,t1325,t1327,t1329,t133,t1332,t1333,t1337,t1338,t1339,t1341,t1343,t1344,t1346,t1347,t1348,t1349,t1350,t1352,t1353,t1354,t1356,t1357,t1358,t1359,t1360,t1362,t1363,t1365,t1369,t1371,t1375,t1376,t1377,t1381,t1386,t1387,t1390,t1391,t1392,t1393,t1395,t1396,t1398,t1401,t1402,t1404,t1405,t1406,t1407,t1408,t1409,t1410,t1411,t1413,t1414,t1415,t1420,t1422,t1423,t1424,t1426,t1427,t1428,t1429,t1430,t1431,t1432,t1435,t1437,t144,t1441,t1442,t1443,t1445,t1446,t1447,t1448,t1449,t1450,t1451,t1452,t1454,t1455,t1458,t146,t1461,t1463,t1465,t1467,t1468,t1469,t1470,t1472,t1474,t1475,t1476,t1478,t1480,t1482,t1483,t1486,t1487,t1489,t1493,t1494,t1495,t1496,t1498,t1499,t15,t1500,t1501,t1502,t1503,t1505,t1506,t1507,t1508,t151,t1511,t1513,t1514,t1515,t1517,t1518,t1523,t1526,t1528,t1529,t1530,t1532,t1534,t1535,t1538,t1539,t1542,t1543,t1545,t1546,t1551,t1553,t1556,t1557,t1565,t1568,t1570,t1573,t1579,t1585,t1590,t1591,t1603,t1605,t1610,t1612,t1614,t1616,t1617,t1618,t1619,t1620,t1622,t1623,t1625,t1627,t1628,t163,t1631,t1633,t1636,t1638,t1639,t1641,t1642,t1647,t1648,t1649,t1651,t1653,t1654,t1656,t1658,t1659,t1660,t1662,t1663,t1664,t1665,t1668,t1670,t1671,t1672,t1673,t1676,t1682,t1683,t1685,t1686,t1687,t1689,t169,t1690,t17,t170,t1700,t171,t1710,t1714,t1716,t1719,t1720,t1723,t1730,t1734,t1746,t1747,t1756,t1763,t177,t178,t179,t18,t1828,t1839,t1863,t190,t1908,t192,t193,t198,t2,t20,t211,t212,t213,t214,t219,t22,t220,t225,t228,t229,t235,t236,t237,t239,t241,t243,t246,t249,t25,t251,t252,t255,t256,t257,t259,t26,t261,t264,t265,t267,t268,t269,t270,t271,t274,t275,t277,t289,t29,t292,t293,t294,t296,t297,t299,t3,t30,t300,t31,t314,t323,t324,t325,t328,t329,t331,t334,t335,t341,t342,t343,t344,t345,t346,t347,t348,t349,t35,t351,t352,t353,t354,t355,t356,t36,t361,t368,t370,t371,t377,t378,t380,t382,t384,t387,t39,t390,t393,t40,t400,t405,t406,t414,t419,t420,t421,t423,t426,t427,t429,t432,t433,t441,t442,t443,t444,t448,t449,t450,t451,t452,t453,t455,t458,t459,t464,t465,t470,t471,t472,t476,t477,t479,t480,t481,t483,t486,t487,t491,t493,t494,t495,t496,t497,t498,t499,t502,t504,t505,t506,t507,t508,t509,t512,t513,t519,t520,t521,t522,t525,t527,t528,t530,t536,t539,t540,t541,t542,t543,t549,t551,t552,t553,t554,t555,t558,t559,t560,t561,t564,t566,t568,t569,t573,t574,t575,t576,t577,t580,t581,t583,t584,t585,t586,t587,t588,t589,t594,t595,t596,t597,t598,t599,t6,t60,t600,t602,t603,t604,t605,t606,t607,t608,t609,t61,t610,t611,t612,t614,t619,t620,t622,t623,t624,t626,t627,t63,t631,t633,t638,t639,t640,t641,t645,t647,t651,t652,t653,t659,t661,t662,t663,t664,t665,t666,t667,t668,t669,t670,t672,t673,t674,t677,t679,t68,t681,t682,t685,t688,t691,t692,t693,t694,t695,t696,t697,t698,t699,t7,t700,t701,t702,t703,t704,t705,t706,t708,t71,t710,t711,t712,t713,t714,t716,t717,t718,t719,t721,t722,t723,t724,t725,t726,t727,t728,t729,t730,t731,t732,t735,t736,t738,t739,t740,t742,t743,t744,t745,t746,t748,t75,t750,t752,t753,t754,t755,t757,t760,t762,t763,t764,t765,t766,t768,t770,t771,t772,t773,t774,t775,t776,t777,t778,t779,t780,t782,t783,t784,t785,t786,t787,t788,t789,t79,t790,t791,t792,t793,t794,t795,t796,t798,t799,t8,t800,t801,t802,t803,t804,t805,t806,t808,t809,t811,t812,t813,t814,t815,t816,t817,t818,t819,t821,t822,t824,t825,t826,t827,t828,t829,t830,t831,t834,t835,t836,t837,t838,t839,t844,t846,t847,t848,t850,t852,t855,t857,t861,t862,t869,t871,t872,t873,t874,t875,t876,t881,t882,t883,t884,t885,t887,t888,t889,t890,t891,t895,t896,t897,t898,t9,t900,t902,t903,t904,t905,t906,t907,t908,t909,t911,t912,t914,t915,t916,t917,t918,t919,t92,t921,t922,t923,t924,t932,t933,t934,t935,t936,t937,t938,t941,t942,t943,t946,t947,t948,t950,t952,t953,t954,t955,t956,t962,t965,t966,t967,t968,t969,t970,t972,t973,t974,t975,t976,t977,t978,t979,t981,t982,t983,t984,t985,t986,t987,t988,t989,t990,t991,t992,t993,t994,t995,t996,t997,t998,t999});
end
function Y = ft_3(ct)
qd1 = ct{1};
qd2 = ct{2};
qd3 = ct{3};
qd4 = ct{4};
qd5 = ct{5};
qd6 = ct{6};
qdd1 = ct{7};
qdd2 = ct{8};
qdd3 = ct{9};
qdd4 = ct{10};
qdd5 = ct{11};
qdd6 = ct{12};
t1000 = ct{13};
t1001 = ct{14};
t1003 = ct{15};
t1004 = ct{16};
t1005 = ct{17};
t1006 = ct{18};
t1009 = ct{19};
t1012 = ct{20};
t1013 = ct{21};
t1014 = ct{22};
t1015 = ct{23};
t1018 = ct{24};
t1019 = ct{25};
t1023 = ct{26};
t1024 = ct{27};
t1026 = ct{28};
t1029 = ct{29};
t1030 = ct{30};
t1031 = ct{31};
t1032 = ct{32};
t1033 = ct{33};
t1034 = ct{34};
t1036 = ct{35};
t1038 = ct{36};
t1039 = ct{37};
t1040 = ct{38};
t1041 = ct{39};
t1042 = ct{40};
t1043 = ct{41};
t1048 = ct{42};
t1049 = ct{43};
t1050 = ct{44};
t1051 = ct{45};
t1052 = ct{46};
t1053 = ct{47};
t1054 = ct{48};
t1055 = ct{49};
t1057 = ct{50};
t1059 = ct{51};
t1061 = ct{52};
t1062 = ct{53};
t1064 = ct{54};
t1065 = ct{55};
t1069 = ct{56};
t1070 = ct{57};
t1072 = ct{58};
t1073 = ct{59};
t1074 = ct{60};
t1075 = ct{61};
t1076 = ct{62};
t1078 = ct{63};
t108 = ct{64};
t1081 = ct{65};
t1083 = ct{66};
t1084 = ct{67};
t109 = ct{68};
t1091 = ct{69};
t1092 = ct{70};
t1093 = ct{71};
t1094 = ct{72};
t1097 = ct{73};
t1099 = ct{74};
t1100 = ct{75};
t1101 = ct{76};
t1102 = ct{77};
t1103 = ct{78};
t1108 = ct{79};
t1116 = ct{80};
t1117 = ct{81};
t1119 = ct{82};
t1120 = ct{83};
t1121 = ct{84};
t1122 = ct{85};
t1124 = ct{86};
t1125 = ct{87};
t1127 = ct{88};
t1128 = ct{89};
t1129 = ct{90};
t1131 = ct{91};
t1132 = ct{92};
t1133 = ct{93};
t1135 = ct{94};
t1136 = ct{95};
t1138 = ct{96};
t1139 = ct{97};
t1140 = ct{98};
t1141 = ct{99};
t1142 = ct{100};
t1143 = ct{101};
t1146 = ct{102};
t1147 = ct{103};
t1148 = ct{104};
t1149 = ct{105};
t1150 = ct{106};
t1151 = ct{107};
t1152 = ct{108};
t1153 = ct{109};
t1154 = ct{110};
t1155 = ct{111};
t1156 = ct{112};
t1157 = ct{113};
t1158 = ct{114};
t1161 = ct{115};
t1162 = ct{116};
t1163 = ct{117};
t1164 = ct{118};
t1165 = ct{119};
t1166 = ct{120};
t1168 = ct{121};
t1169 = ct{122};
t1170 = ct{123};
t1173 = ct{124};
t1174 = ct{125};
t1176 = ct{126};
t1178 = ct{127};
t1179 = ct{128};
t1180 = ct{129};
t1181 = ct{130};
t1182 = ct{131};
t1183 = ct{132};
t1184 = ct{133};
t1186 = ct{134};
t1187 = ct{135};
t1188 = ct{136};
t1189 = ct{137};
t1190 = ct{138};
t1198 = ct{139};
t12 = ct{140};
t1200 = ct{141};
t1202 = ct{142};
t1203 = ct{143};
t1204 = ct{144};
t1207 = ct{145};
t1208 = ct{146};
t1209 = ct{147};
t1211 = ct{148};
t1212 = ct{149};
t1213 = ct{150};
t1215 = ct{151};
t1220 = ct{152};
t1221 = ct{153};
t1225 = ct{154};
t1226 = ct{155};
t1227 = ct{156};
t1228 = ct{157};
t1229 = ct{158};
t1230 = ct{159};
t1233 = ct{160};
t1234 = ct{161};
t1235 = ct{162};
t1236 = ct{163};
t1237 = ct{164};
t1238 = ct{165};
t1239 = ct{166};
t1240 = ct{167};
t1242 = ct{168};
t1243 = ct{169};
t1244 = ct{170};
t1246 = ct{171};
t1247 = ct{172};
t1251 = ct{173};
t1252 = ct{174};
t1253 = ct{175};
t1254 = ct{176};
t1255 = ct{177};
t1256 = ct{178};
t1258 = ct{179};
t1259 = ct{180};
t1260 = ct{181};
t1261 = ct{182};
t1262 = ct{183};
t1264 = ct{184};
t1265 = ct{185};
t1267 = ct{186};
t1268 = ct{187};
t127 = ct{188};
t1270 = ct{189};
t1274 = ct{190};
t1275 = ct{191};
t1281 = ct{192};
t1284 = ct{193};
t1286 = ct{194};
t1288 = ct{195};
t1289 = ct{196};
t1292 = ct{197};
t1293 = ct{198};
t1294 = ct{199};
t1297 = ct{200};
t1298 = ct{201};
t1299 = ct{202};
t13 = ct{203};
t130 = ct{204};
t1304 = ct{205};
t1305 = ct{206};
t1306 = ct{207};
t1307 = ct{208};
t1310 = ct{209};
t1311 = ct{210};
t1314 = ct{211};
t1315 = ct{212};
t1317 = ct{213};
t1318 = ct{214};
t1319 = ct{215};
t132 = ct{216};
t1321 = ct{217};
t1322 = ct{218};
t1323 = ct{219};
t1325 = ct{220};
t1327 = ct{221};
t1329 = ct{222};
t133 = ct{223};
t1332 = ct{224};
t1333 = ct{225};
t1337 = ct{226};
t1338 = ct{227};
t1339 = ct{228};
t1341 = ct{229};
t1343 = ct{230};
t1344 = ct{231};
t1346 = ct{232};
t1347 = ct{233};
t1348 = ct{234};
t1349 = ct{235};
t1350 = ct{236};
t1352 = ct{237};
t1353 = ct{238};
t1354 = ct{239};
t1356 = ct{240};
t1357 = ct{241};
t1358 = ct{242};
t1359 = ct{243};
t1360 = ct{244};
t1362 = ct{245};
t1363 = ct{246};
t1365 = ct{247};
t1369 = ct{248};
t1371 = ct{249};
t1375 = ct{250};
t1376 = ct{251};
t1377 = ct{252};
t1381 = ct{253};
t1386 = ct{254};
t1387 = ct{255};
t1390 = ct{256};
t1391 = ct{257};
t1392 = ct{258};
t1393 = ct{259};
t1395 = ct{260};
t1396 = ct{261};
t1398 = ct{262};
t1401 = ct{263};
t1402 = ct{264};
t1404 = ct{265};
t1405 = ct{266};
t1406 = ct{267};
t1407 = ct{268};
t1408 = ct{269};
t1409 = ct{270};
t1410 = ct{271};
t1411 = ct{272};
t1413 = ct{273};
t1414 = ct{274};
t1415 = ct{275};
t1420 = ct{276};
t1422 = ct{277};
t1423 = ct{278};
t1424 = ct{279};
t1426 = ct{280};
t1427 = ct{281};
t1428 = ct{282};
t1429 = ct{283};
t1430 = ct{284};
t1431 = ct{285};
t1432 = ct{286};
t1435 = ct{287};
t1437 = ct{288};
t144 = ct{289};
t1441 = ct{290};
t1442 = ct{291};
t1443 = ct{292};
t1445 = ct{293};
t1446 = ct{294};
t1447 = ct{295};
t1448 = ct{296};
t1449 = ct{297};
t1450 = ct{298};
t1451 = ct{299};
t1452 = ct{300};
t1454 = ct{301};
t1455 = ct{302};
t1458 = ct{303};
t146 = ct{304};
t1461 = ct{305};
t1463 = ct{306};
t1465 = ct{307};
t1467 = ct{308};
t1468 = ct{309};
t1469 = ct{310};
t1470 = ct{311};
t1472 = ct{312};
t1474 = ct{313};
t1475 = ct{314};
t1476 = ct{315};
t1478 = ct{316};
t1480 = ct{317};
t1482 = ct{318};
t1483 = ct{319};
t1486 = ct{320};
t1487 = ct{321};
t1489 = ct{322};
t1493 = ct{323};
t1494 = ct{324};
t1495 = ct{325};
t1496 = ct{326};
t1498 = ct{327};
t1499 = ct{328};
t15 = ct{329};
t1500 = ct{330};
t1501 = ct{331};
t1502 = ct{332};
t1503 = ct{333};
t1505 = ct{334};
t1506 = ct{335};
t1507 = ct{336};
t1508 = ct{337};
t151 = ct{338};
t1511 = ct{339};
t1513 = ct{340};
t1514 = ct{341};
t1515 = ct{342};
t1517 = ct{343};
t1518 = ct{344};
t1523 = ct{345};
t1526 = ct{346};
t1528 = ct{347};
t1529 = ct{348};
t1530 = ct{349};
t1532 = ct{350};
t1534 = ct{351};
t1535 = ct{352};
t1538 = ct{353};
t1539 = ct{354};
t1542 = ct{355};
t1543 = ct{356};
t1545 = ct{357};
t1546 = ct{358};
t1551 = ct{359};
t1553 = ct{360};
t1556 = ct{361};
t1557 = ct{362};
t1565 = ct{363};
t1568 = ct{364};
t1570 = ct{365};
t1573 = ct{366};
t1579 = ct{367};
t1585 = ct{368};
t1590 = ct{369};
t1591 = ct{370};
t1603 = ct{371};
t1605 = ct{372};
t1610 = ct{373};
t1612 = ct{374};
t1614 = ct{375};
t1616 = ct{376};
t1617 = ct{377};
t1618 = ct{378};
t1619 = ct{379};
t1620 = ct{380};
t1622 = ct{381};
t1623 = ct{382};
t1625 = ct{383};
t1627 = ct{384};
t1628 = ct{385};
t163 = ct{386};
t1631 = ct{387};
t1633 = ct{388};
t1636 = ct{389};
t1638 = ct{390};
t1639 = ct{391};
t1641 = ct{392};
t1642 = ct{393};
t1647 = ct{394};
t1648 = ct{395};
t1649 = ct{396};
t1651 = ct{397};
t1653 = ct{398};
t1654 = ct{399};
t1656 = ct{400};
t1658 = ct{401};
t1659 = ct{402};
t1660 = ct{403};
t1662 = ct{404};
t1663 = ct{405};
t1664 = ct{406};
t1665 = ct{407};
t1668 = ct{408};
t1670 = ct{409};
t1671 = ct{410};
t1672 = ct{411};
t1673 = ct{412};
t1676 = ct{413};
t1682 = ct{414};
t1683 = ct{415};
t1685 = ct{416};
t1686 = ct{417};
t1687 = ct{418};
t1689 = ct{419};
t169 = ct{420};
t1690 = ct{421};
t17 = ct{422};
t170 = ct{423};
t1700 = ct{424};
t171 = ct{425};
t1710 = ct{426};
t1714 = ct{427};
t1716 = ct{428};
t1719 = ct{429};
t1720 = ct{430};
t1723 = ct{431};
t1730 = ct{432};
t1734 = ct{433};
t1746 = ct{434};
t1747 = ct{435};
t1756 = ct{436};
t1763 = ct{437};
t177 = ct{438};
t178 = ct{439};
t179 = ct{440};
t18 = ct{441};
t1828 = ct{442};
t1839 = ct{443};
t1863 = ct{444};
t190 = ct{445};
t1908 = ct{446};
t192 = ct{447};
t193 = ct{448};
t198 = ct{449};
t2 = ct{450};
t20 = ct{451};
t211 = ct{452};
t212 = ct{453};
t213 = ct{454};
t214 = ct{455};
t219 = ct{456};
t22 = ct{457};
t220 = ct{458};
t225 = ct{459};
t228 = ct{460};
t229 = ct{461};
t235 = ct{462};
t236 = ct{463};
t237 = ct{464};
t239 = ct{465};
t241 = ct{466};
t243 = ct{467};
t246 = ct{468};
t249 = ct{469};
t25 = ct{470};
t251 = ct{471};
t252 = ct{472};
t255 = ct{473};
t256 = ct{474};
t257 = ct{475};
t259 = ct{476};
t26 = ct{477};
t261 = ct{478};
t264 = ct{479};
t265 = ct{480};
t267 = ct{481};
t268 = ct{482};
t269 = ct{483};
t270 = ct{484};
t271 = ct{485};
t274 = ct{486};
t275 = ct{487};
t277 = ct{488};
t289 = ct{489};
t29 = ct{490};
t292 = ct{491};
t293 = ct{492};
t294 = ct{493};
t296 = ct{494};
t297 = ct{495};
t299 = ct{496};
t3 = ct{497};
t30 = ct{498};
t300 = ct{499};
t31 = ct{500};
t314 = ct{501};
t323 = ct{502};
t324 = ct{503};
t325 = ct{504};
t328 = ct{505};
t329 = ct{506};
t331 = ct{507};
t334 = ct{508};
t335 = ct{509};
t341 = ct{510};
t342 = ct{511};
t343 = ct{512};
t344 = ct{513};
t345 = ct{514};
t346 = ct{515};
t347 = ct{516};
t348 = ct{517};
t349 = ct{518};
t35 = ct{519};
t351 = ct{520};
t352 = ct{521};
t353 = ct{522};
t354 = ct{523};
t355 = ct{524};
t356 = ct{525};
t36 = ct{526};
t361 = ct{527};
t368 = ct{528};
t370 = ct{529};
t371 = ct{530};
t377 = ct{531};
t378 = ct{532};
t380 = ct{533};
t382 = ct{534};
t384 = ct{535};
t387 = ct{536};
t39 = ct{537};
t390 = ct{538};
t393 = ct{539};
t40 = ct{540};
t400 = ct{541};
t405 = ct{542};
t406 = ct{543};
t414 = ct{544};
t419 = ct{545};
t420 = ct{546};
t421 = ct{547};
t423 = ct{548};
t426 = ct{549};
t427 = ct{550};
t429 = ct{551};
t432 = ct{552};
t433 = ct{553};
t441 = ct{554};
t442 = ct{555};
t443 = ct{556};
t444 = ct{557};
t448 = ct{558};
t449 = ct{559};
t450 = ct{560};
t451 = ct{561};
t452 = ct{562};
t453 = ct{563};
t455 = ct{564};
t458 = ct{565};
t459 = ct{566};
t464 = ct{567};
t465 = ct{568};
t470 = ct{569};
t471 = ct{570};
t472 = ct{571};
t476 = ct{572};
t477 = ct{573};
t479 = ct{574};
t480 = ct{575};
t481 = ct{576};
t483 = ct{577};
t486 = ct{578};
t487 = ct{579};
t491 = ct{580};
t493 = ct{581};
t494 = ct{582};
t495 = ct{583};
t496 = ct{584};
t497 = ct{585};
t498 = ct{586};
t499 = ct{587};
t502 = ct{588};
t504 = ct{589};
t505 = ct{590};
t506 = ct{591};
t507 = ct{592};
t508 = ct{593};
t509 = ct{594};
t512 = ct{595};
t513 = ct{596};
t519 = ct{597};
t520 = ct{598};
t521 = ct{599};
t522 = ct{600};
t525 = ct{601};
t527 = ct{602};
t528 = ct{603};
t530 = ct{604};
t536 = ct{605};
t539 = ct{606};
t540 = ct{607};
t541 = ct{608};
t542 = ct{609};
t543 = ct{610};
t549 = ct{611};
t551 = ct{612};
t552 = ct{613};
t553 = ct{614};
t554 = ct{615};
t555 = ct{616};
t558 = ct{617};
t559 = ct{618};
t560 = ct{619};
t561 = ct{620};
t564 = ct{621};
t566 = ct{622};
t568 = ct{623};
t569 = ct{624};
t573 = ct{625};
t574 = ct{626};
t575 = ct{627};
t576 = ct{628};
t577 = ct{629};
t580 = ct{630};
t581 = ct{631};
t583 = ct{632};
t584 = ct{633};
t585 = ct{634};
t586 = ct{635};
t587 = ct{636};
t588 = ct{637};
t589 = ct{638};
t594 = ct{639};
t595 = ct{640};
t596 = ct{641};
t597 = ct{642};
t598 = ct{643};
t599 = ct{644};
t6 = ct{645};
t60 = ct{646};
t600 = ct{647};
t602 = ct{648};
t603 = ct{649};
t604 = ct{650};
t605 = ct{651};
t606 = ct{652};
t607 = ct{653};
t608 = ct{654};
t609 = ct{655};
t61 = ct{656};
t610 = ct{657};
t611 = ct{658};
t612 = ct{659};
t614 = ct{660};
t619 = ct{661};
t620 = ct{662};
t622 = ct{663};
t623 = ct{664};
t624 = ct{665};
t626 = ct{666};
t627 = ct{667};
t63 = ct{668};
t631 = ct{669};
t633 = ct{670};
t638 = ct{671};
t639 = ct{672};
t640 = ct{673};
t641 = ct{674};
t645 = ct{675};
t647 = ct{676};
t651 = ct{677};
t652 = ct{678};
t653 = ct{679};
t659 = ct{680};
t661 = ct{681};
t662 = ct{682};
t663 = ct{683};
t664 = ct{684};
t665 = ct{685};
t666 = ct{686};
t667 = ct{687};
t668 = ct{688};
t669 = ct{689};
t670 = ct{690};
t672 = ct{691};
t673 = ct{692};
t674 = ct{693};
t677 = ct{694};
t679 = ct{695};
t68 = ct{696};
t681 = ct{697};
t682 = ct{698};
t685 = ct{699};
t688 = ct{700};
t691 = ct{701};
t692 = ct{702};
t693 = ct{703};
t694 = ct{704};
t695 = ct{705};
t696 = ct{706};
t697 = ct{707};
t698 = ct{708};
t699 = ct{709};
t7 = ct{710};
t700 = ct{711};
t701 = ct{712};
t702 = ct{713};
t703 = ct{714};
t704 = ct{715};
t705 = ct{716};
t706 = ct{717};
t708 = ct{718};
t71 = ct{719};
t710 = ct{720};
t711 = ct{721};
t712 = ct{722};
t713 = ct{723};
t714 = ct{724};
t716 = ct{725};
t717 = ct{726};
t718 = ct{727};
t719 = ct{728};
t721 = ct{729};
t722 = ct{730};
t723 = ct{731};
t724 = ct{732};
t725 = ct{733};
t726 = ct{734};
t727 = ct{735};
t728 = ct{736};
t729 = ct{737};
t730 = ct{738};
t731 = ct{739};
t732 = ct{740};
t735 = ct{741};
t736 = ct{742};
t738 = ct{743};
t739 = ct{744};
t740 = ct{745};
t742 = ct{746};
t743 = ct{747};
t744 = ct{748};
t745 = ct{749};
t746 = ct{750};
t748 = ct{751};
t75 = ct{752};
t750 = ct{753};
t752 = ct{754};
t753 = ct{755};
t754 = ct{756};
t755 = ct{757};
t757 = ct{758};
t760 = ct{759};
t762 = ct{760};
t763 = ct{761};
t764 = ct{762};
t765 = ct{763};
t766 = ct{764};
t768 = ct{765};
t770 = ct{766};
t771 = ct{767};
t772 = ct{768};
t773 = ct{769};
t774 = ct{770};
t775 = ct{771};
t776 = ct{772};
t777 = ct{773};
t778 = ct{774};
t779 = ct{775};
t780 = ct{776};
t782 = ct{777};
t783 = ct{778};
t784 = ct{779};
t785 = ct{780};
t786 = ct{781};
t787 = ct{782};
t788 = ct{783};
t789 = ct{784};
t79 = ct{785};
t790 = ct{786};
t791 = ct{787};
t792 = ct{788};
t793 = ct{789};
t794 = ct{790};
t795 = ct{791};
t796 = ct{792};
t798 = ct{793};
t799 = ct{794};
t8 = ct{795};
t800 = ct{796};
t801 = ct{797};
t802 = ct{798};
t803 = ct{799};
t804 = ct{800};
t805 = ct{801};
t806 = ct{802};
t808 = ct{803};
t809 = ct{804};
t811 = ct{805};
t812 = ct{806};
t813 = ct{807};
t814 = ct{808};
t815 = ct{809};
t816 = ct{810};
t817 = ct{811};
t818 = ct{812};
t819 = ct{813};
t821 = ct{814};
t822 = ct{815};
t824 = ct{816};
t825 = ct{817};
t826 = ct{818};
t827 = ct{819};
t828 = ct{820};
t829 = ct{821};
t830 = ct{822};
t831 = ct{823};
t834 = ct{824};
t835 = ct{825};
t836 = ct{826};
t837 = ct{827};
t838 = ct{828};
t839 = ct{829};
t844 = ct{830};
t846 = ct{831};
t847 = ct{832};
t848 = ct{833};
t850 = ct{834};
t852 = ct{835};
t855 = ct{836};
t857 = ct{837};
t861 = ct{838};
t862 = ct{839};
t869 = ct{840};
t871 = ct{841};
t872 = ct{842};
t873 = ct{843};
t874 = ct{844};
t875 = ct{845};
t876 = ct{846};
t881 = ct{847};
t882 = ct{848};
t883 = ct{849};
t884 = ct{850};
t885 = ct{851};
t887 = ct{852};
t888 = ct{853};
t889 = ct{854};
t890 = ct{855};
t891 = ct{856};
t895 = ct{857};
t896 = ct{858};
t897 = ct{859};
t898 = ct{860};
t9 = ct{861};
t900 = ct{862};
t902 = ct{863};
t903 = ct{864};
t904 = ct{865};
t905 = ct{866};
t906 = ct{867};
t907 = ct{868};
t908 = ct{869};
t909 = ct{870};
t911 = ct{871};
t912 = ct{872};
t914 = ct{873};
t915 = ct{874};
t916 = ct{875};
t917 = ct{876};
t918 = ct{877};
t919 = ct{878};
t92 = ct{879};
t921 = ct{880};
t922 = ct{881};
t923 = ct{882};
t924 = ct{883};
t932 = ct{884};
t933 = ct{885};
t934 = ct{886};
t935 = ct{887};
t936 = ct{888};
t937 = ct{889};
t938 = ct{890};
t941 = ct{891};
t942 = ct{892};
t943 = ct{893};
t946 = ct{894};
t947 = ct{895};
t948 = ct{896};
t950 = ct{897};
t952 = ct{898};
t953 = ct{899};
t954 = ct{900};
t955 = ct{901};
t956 = ct{902};
t962 = ct{903};
t965 = ct{904};
t966 = ct{905};
t967 = ct{906};
t968 = ct{907};
t969 = ct{908};
t970 = ct{909};
t972 = ct{910};
t973 = ct{911};
t974 = ct{912};
t975 = ct{913};
t976 = ct{914};
t977 = ct{915};
t978 = ct{916};
t979 = ct{917};
t981 = ct{918};
t982 = ct{919};
t983 = ct{920};
t984 = ct{921};
t985 = ct{922};
t986 = ct{923};
t987 = ct{924};
t988 = ct{925};
t989 = ct{926};
t990 = ct{927};
t991 = ct{928};
t992 = ct{929};
t993 = ct{930};
t994 = ct{931};
t995 = ct{932};
t996 = ct{933};
t997 = ct{934};
t998 = ct{935};
t999 = ct{936};
t1691 = t917.*t1314;
t1693 = t2.*t904.*t1314;
t1694 = t442+t465+t647+t1029;
t1695 = t427+t471+t653+t1014;
t1697 = (t948.*t1274)./2.0;
t1698 = -t1686;
t1699 = -t1687;
t1705 = t1686./2.0;
t1706 = t1687./2.0;
t1724 = t1714./2.0;
t1725 = t1716./2.0;
t1726 = t2.*t942.*t1314;
t1727 = -t1720;
t1729 = t1720./2.0;
t1737 = (t1138.*t1165)./2.0;
t1739 = (t2.*t953.*t1314)./2.0;
t1750 = -t1746;
t1753 = t1746./2.0;
t1758 = -t1101.*(t426-t1001);
t1762 = t640+t652+t746+t763;
t1764 = t943.*t1395;
t1768 = t257+t464+t976+t1004;
t1772 = t271+t470+t955+t1023;
t1774 = t1138.*t1274;
t1775 = t1101.*t1314;
t1777 = t1165.*t1274;
t1789 = (t943.*t1495)./2.0;
t1795 = -t948.*(t936-t937);
t1803 = t948.*(t936-t937).*(-1.0./2.0);
t1807 = t641+t717+t839+t855;
t1808 = (t948.*(t936-t937))./2.0;
t1811 = t943.*t1534;
t1813 = t620+t736+t857+t872;
t1815 = -t1314.*(t426-t1001);
t1827 = t1108.*(t936-t937).*(-1.0./2.0);
t1833 = t1828.*2.0;
t1837 = -t1828;
t1849 = t1839.*2.0;
t1851 = -t1138.*(t936-t937);
t1858 = t1138.*(t936-t937);
t1866 = -t1100.*(t421-t432-t619+t718);
t1872 = -t1863;
t1874 = t1863./2.0;
t1878 = t1100.*(t421-t432-t619+t718).*(-1.0./2.0);
t1899 = -t1274.*(t936-t937);
t1902 = t1274.*(t936-t937);
t1904 = t328+t347+t714+t732+t764+t772;
t1912 = -t8.*t773.*(t261+t455-t955-t1023);
t1921 = t8.*t773.*(t261+t455-t955-t1023).*(-1.0./2.0);
t1922 = (t8.*t773.*(t261+t455-t955-t1023))./2.0;
t1931 = -t8.*t890.*(t261+t455-t955-t1023);
t1932 = t219+t343+t770+t779+t819+t848;
t1936 = t8.*t890.*(t261+t455-t955-t1023).*(-1.0./2.0);
t1941 = (t8.*t890.*(t261+t455-t955-t1023))./2.0;
t1945 = t800+t811+t989+t990;
t1951 = -t1101.*(t441-t442-t647+t1012);
t1958 = t1101.*(t441-t442-t647+t1012);
t1965 = -t8.*t942.*(t261+t455-t955-t1023);
t1975 = t8.*t942.*(t261+t455-t955-t1023).*(-1.0./2.0);
t1980 = (t8.*t942.*(t261+t455-t955-t1023))./2.0;
t2056 = t1314.*(t441-t442-t647+t1012).*(-1.0./2.0);
t2058 = (t1314.*(t441-t442-t647+t1012))./2.0;
t2089 = (t443-t1013).*(t261+t455-t955-t1023);
t2095 = t947+t954+t1052+t1053;
t2216 = t703+t719+t831+t970+t979+t1174;
t925 = -t922;
t926 = -t921;
t980 = t555+t573;
t1007 = t236.*t569.*4.042016666666667e-4;
t1008 = t236.*t569.*8.084033333333334e-4;
t1016 = t12.*t39.*t659.*4.042016666666667e-4;
t1017 = t12.*t39.*t659.*8.084033333333334e-4;
t1066 = t387.*t812;
t1068 = t7.*t132.*t659.*8.084033333333334e-4;
t1071 = t325.*t569.*8.084033333333334e-4;
t1077 = t192.*t659.*8.084033333333334e-4;
t1082 = t7.*t171.*t659.*8.084033333333334e-4;
t1085 = -t1076;
t1086 = -t1075;
t1095 = t237.*t659.*4.042016666666667e-4;
t1096 = t237.*t659.*8.084033333333334e-4;
t1104 = t569.*(t61-t239).*(-8.084033333333334e-4);
t1105 = -t1094;
t1109 = t249.*t659.*8.084033333333334e-4;
t1112 = t252.*t659.*8.084033333333334e-4;
t1113 = t569.*(t61-t239).*8.084033333333334e-4;
t1118 = t2.*t1099;
t1126 = -t1122;
t1130 = t1117./2.0;
t1144 = t659.*(t60-t190).*(-8.084033333333334e-4);
t1145 = t341.*t659.*8.084033333333334e-4;
t1159 = t539+t799;
t1160 = t542+t803;
t1171 = t564+t821;
t1172 = t566+t822;
t1177 = -t25.*(t527+t813);
t1185 = t29.*t1164;
t1192 = t25.*(t527+t813).*(-1.0./2.0);
t1194 = t1186.*(-1.0./2.0);
t1196 = -t1188;
t1199 = t12.*t25.*t1164;
t1201 = t1186./2.0;
t1217 = t12.*t39.*t923.*8.084033333333334e-4;
t1232 = t294+t1099;
t1250 = t2.*t1233;
t1257 = t8.*t1240;
t1263 = t748+t766;
t1269 = t7.*t132.*t923.*8.084033333333334e-4;
t1271 = -t1261;
t1273 = -t1258;
t1277 = t2.*t1253;
t1278 = t8.*t1254;
t1279 = t192.*t923.*8.084033333333334e-4;
t1280 = t7.*t171.*t923.*8.084033333333334e-4;
t1290 = t237.*t923.*4.042016666666667e-4;
t1291 = t237.*t923.*8.084033333333334e-4;
t1295 = t249.*t923.*8.084033333333334e-4;
t1296 = t252.*t923.*8.084033333333334e-4;
t1300 = t2.*t25.*t1254;
t1301 = t8.*t25.*t1253;
t1302 = t2.*t29.*t1254;
t1303 = t8.*t29.*t1253;
t1316 = t1305./2.0;
t1328 = t12.*t40.*t1059.*8.084033333333334e-4;
t1330 = t923.*(t60-t190).*(-8.084033333333334e-4);
t1331 = t341.*t923.*8.084033333333334e-4;
t1334 = t923.*(t60-t190).*8.084033333333334e-4;
t1335 = t802+t816;
t1345 = t812.*(t2.*(t296-t2.*t9.*(1.53e+2./2.5e+2))+t8.*(t299-t8.*t9.*(1.53e+2./2.5e+2))).*(-1.0./2.0);
t1366 = -t1359;
t1367 = t13.*t132.*t1059.*8.084033333333334e-4;
t1368 = t8.*t491.*t1099;
t1370 = t108+t225+t246+t314+t483+t504;
t1373 = t193.*t1059.*4.042016666666667e-4;
t1374 = t193.*t1059.*8.084033333333334e-4;
t1378 = t13.*t171.*t1059.*8.084033333333334e-4;
t1384 = t1362./2.0;
t1385 = -t1369;
t1389 = t236.*t1059.*8.084033333333334e-4;
t1394 = t1369./2.0;
t1397 = t721.*t943;
t1417 = t269.*t1059.*8.084033333333334e-4;
t1418 = t270.*t1059.*8.084033333333334e-4;
t1419 = t1398./2.0;
t1433 = t1414./2.0;
t1434 = -t1426;
t1436 = -t1429;
t1438 = t268+t292+t349+t353+t390+t414;
t1439 = -t1432;
t1444 = t325.*t1059.*8.084033333333334e-4;
t1456 = t2.*t1447;
t1457 = t8.*t1446;
t1460 = t1059.*(t61-t239).*(-8.084033333333334e-4);
t1477 = t2.*t29.*t1446;
t1479 = t8.*t29.*t1447;
t1485 = -t1480;
t1491 = t1480./2.0;
t1497 = (t370.*t1321)./2.0;
t1509 = t937+t946;
t1510 = t323+t844+t869;
t1516 = -t1508;
t1522 = t8.*t773.*t1099;
t1525 = t8.*t785.*t1099;
t1533 = t1526./2.0;
t1541 = -t1530;
t1544 = t1530./2.0;
t1547 = -t1539;
t1549 = t8.*t491.*t1321;
t1554 = t1539./2.0;
t1555 = -t1546;
t1560 = t1546./2.0;
t1561 = -t1557;
t1571 = t574.*t1321;
t1572 = t8.*t890.*t1099;
t1574 = t1568./2.0;
t1576 = t1570./2.0;
t1577 = t8.*t904.*t1099;
t1578 = (t902.*t1099)./2.0;
t1584 = t1579./2.0;
t1589 = t722.*t1264;
t1592 = t8.*t942.*t1099;
t1597 = t1024+t1050;
t1598 = t1033+t1043;
t1601 = t236.*t1371.*8.084033333333334e-4;
t1602 = t1034+t1055;
t1604 = (t8.*t953.*t1099)./2.0;
t1609 = -t1605;
t1615 = t1612.*(-1.0./2.0);
t1624 = t325.*t1371.*8.084033333333334e-4;
t1634 = t8.*t773.*t1321;
t1637 = t1371.*(t61-t239).*(-8.084033333333334e-4);
t1640 = t8.*t785.*t1321;
t1643 = t1639./2.0;
t1645 = t835.*t1321;
t1652 = t1641./2.0;
t1674 = -t1672;
t1681 = t1119+t1127;
t1684 = t29.*t1658;
t1688 = t8.*t890.*t1321;
t1696 = t1689.*2.0;
t1701 = t8.*t904.*t1321;
t1703 = t915.*t1321;
t1704 = -t1697;
t1708 = -t1705;
t1709 = t1691./2.0;
t1711 = -t1706;
t1712 = t1693./2.0;
t1721 = t192.*t1529.*4.042016666666667e-4;
t1722 = t192.*t1529.*8.084033333333334e-4;
t1728 = t8.*t942.*t1321;
t1731 = -t1729;
t1733 = t1041.*t1264;
t1735 = t236.*t1545.*4.042016666666667e-4;
t1736 = t236.*t1545.*8.084033333333334e-4;
t1738 = -t1737;
t1742 = (t8.*t953.*t1321)./2.0;
t1744 = t739+t808+t1032;
t1745 = t740+t791+t1042;
t1751 = t1529.*(t60-t190).*(-8.084033333333334e-4);
t1752 = t341.*t1529.*8.084033333333334e-4;
t1754 = t1529.*(t60-t190).*8.084033333333334e-4;
t1759 = -t1753;
t1760 = t325.*t1545.*8.084033333333334e-4;
t1761 = t639+t651+t745+t762;
t1765 = -t1099.*(t443-t1013);
t1769 = t1545.*(t61-t239).*(-8.084033333333334e-4);
t1770 = t1764./2.0;
t1776 = t1099.*t1321;
t1778 = -t1777;
t1779 = t1777./2.0;
t1794 = t1138.*t1375;
t1797 = t722.*t1603;
t1814 = t1811./2.0;
t1817 = (t790.*t1603)./2.0;
t1818 = -t1321.*(t443-t1013);
t1826 = t1264.*t1396;
t1834 = (t1274.*t1375)./2.0;
t1838 = -t1833;
t1868 = t8.*t773.*t1695;
t1877 = -t1874;
t1885 = t1041.*t1603;
t1891 = t943.*t1648;
t1893 = (t1264.*t1496)./2.0;
t1896 = t8.*t890.*t1695;
t1905 = t2.*t773.*t1768;
t1907 = t1264.*t1535;
t1909 = t2.*t1904;
t1911 = t8.*t942.*t1695;
t1930 = t2.*t890.*t1768;
t1935 = t198+t335+t771+t780+t850+t861;
t1940 = t8.*t1932;
t1952 = t1099.*t1695;
t1956 = t2.*t942.*t1768;
t1957 = t2.*t29.*t1932;
t1961 = t1264.*t1603;
t1964 = t1958.*(-1.0./2.0);
t1968 = t1958./2.0;
t1984 = t8.*t773.*t1807;
t1992 = t171.*t1932;
t1993 = t2.*t773.*t1813;
t2006 = t1264.*t1649;
t2007 = t1101.*t1768;
t2010 = t8.*t890.*t1807;
t2011 = -t1099.*(t261+t455-t955-t1023);
t2016 = t2.*t890.*t1813;
t2017 = t1099.*(t261+t455-t955-t1023);
t2031 = t8.*t942.*t1807;
t2036 = t2.*t942.*t1813;
t2061 = (t1321.*t1695)./2.0;
t2073 = t1264.*t1762;
t2078 = -t1768.*(t426-t1001);
t2079 = t1768.*(t426-t1001).*-2.0;
t2081 = (t1496.*t1603)./2.0;
t2082 = t1099.*t1807;
t2086 = t1101.*t1813;
t2091 = t2089.*2.0;
t2097 = t1314.*t1768;
t2099 = -t2.*(-t681+t1059.*(t61-t239).*8.084033333333334e-4+t341.*(t289-t476+t171.*(t60-t190)).*8.084033333333334e-4);
t2100 = -t1321.*(t261+t455-t955-t1023);
t2103 = (t1535.*t1603)./2.0;
t2105 = t1321.*(t261+t455-t955-t1023).*(-1.0./2.0);
t2106 = -t8.*t25.*(-t681+t1059.*(t61-t239).*8.084033333333334e-4+t341.*(t289-t476+t171.*(t60-t190)).*8.084033333333334e-4);
t2110 = -t29.*t30.*(-t681+t1059.*(t61-t239).*8.084033333333334e-4+t341.*(t289-t476+t171.*(t60-t190)).*8.084033333333334e-4);
t2112 = t8.*t25.*(-t681+t1059.*(t61-t239).*8.084033333333334e-4+t341.*(t289-t476+t171.*(t60-t190)).*8.084033333333334e-4).*(-1.0./2.0);
t2114 = t29.*t30.*(-t681+t1059.*(t61-t239).*8.084033333333334e-4+t341.*(t289-t476+t171.*(t60-t190)).*8.084033333333334e-4);
t2128 = -t1813.*(t426-t1001);
t2129 = -t1807.*(t443-t1013);
t2130 = t1813.*(t426-t1001);
t2131 = t1807.*(t443-t1013);
t2139 = t1321.*t1807;
t2141 = t1314.*t1813;
t2144 = t1603.*t1649;
t2162 = t1603.*t1762;
t2177 = t519+t521+t700+t701+t1774;
t2179 = t493+t494+t519+t521+t1858;
t2213 = t519+t521+t583+t584+t1902;
t2227 = t25.*t2216;
t2237 = t728+t738+t847+t985+t1048+t1243;
t2238 = t725+t735+t846+t984+t1051+t1237;
t1087 = -t1077;
t1090 = t1066./2.0;
t1114 = -t1109;
t1115 = -t1112;
t1134 = -t1130;
t1193 = t387.*t980;
t1206 = t1185./2.0;
t1210 = -t1199;
t1218 = t1199./2.0;
t1223 = -t1217;
t1249 = t2.*t1232;
t1272 = -t1257;
t1276 = -t1269;
t1285 = -t1280;
t1308 = -t1300;
t1309 = -t1302;
t1312 = t1300./2.0;
t1313 = t1301./2.0;
t1324 = (t568.*t980)./2.0;
t1336 = -t1331;
t1361 = t25.*t1335;
t1380 = -t1368;
t1382 = -t1374;
t1383 = -t1373;
t1388 = t1368./2.0;
t1400 = -t1394;
t1412 = -t1397;
t1416 = t1397./2.0;
t1425 = -t1418;
t1464 = t1456./2.0;
t1466 = t1457./2.0;
t1473 = t812.*t980;
t1484 = -t1477;
t1488 = t1477./2.0;
t1490 = t1479./2.0;
t1531 = t1525./2.0;
t1540 = -t1533;
t1548 = -t1544;
t1558 = -t1554;
t1559 = -t1549;
t1562 = t1549./2.0;
t1563 = -t1560;
t1575 = -t1571;
t1580 = t1571./2.0;
t1581 = -t1576;
t1583 = t1577./2.0;
t1587 = -t1584;
t1588 = t721.*t1263;
t1593 = -t1589;
t1595 = t1589./2.0;
t1596 = t192.*t1370.*8.084033333333334e-4;
t1606 = t2.*t1597;
t1608 = -t1604;
t1629 = t1370.*(t60-t190).*(-8.084033333333334e-4);
t1630 = t341.*t1370.*8.084033333333334e-4;
t1644 = t1640./2.0;
t1646 = -t1643;
t1657 = -t1645;
t1661 = t1645./2.0;
t1679 = t943.*t1263;
t1680 = t1118+t1126;
t1692 = -t1684;
t1702 = t1684./2.0;
t1713 = -t1703;
t1715 = t1701./2.0;
t1717 = t1703./2.0;
t1732 = t1040.*t1263;
t1741 = t1733./2.0;
t1748 = t2.*t1745;
t1749 = t8.*t1744;
t1755 = -t1752;
t1766 = t2.*t25.*t1744;
t1767 = t8.*t25.*t1745;
t1793 = t1250+t1273;
t1796 = t721.*t1602;
t1798 = -t1794;
t1800 = -t1797;
t1801 = t1794./2.0;
t1804 = t1263.*(t384+t472+t477+t26.*t29.*t132.*1.383e-1);
t1806 = t1797./2.0;
t1816 = (t789.*t1602)./2.0;
t1819 = t611+t1136+t1144;
t1820 = t598+t1145+t1158;
t1824 = t722.*t1681;
t1825 = t1263.*t1395;
t1845 = t1826./2.0;
t1852 = t943.*t1602;
t1865 = (t790.*t1681)./2.0;
t1880 = t1868./2.0;
t1884 = t1040.*t1602;
t1886 = -t1885;
t1888 = t1885./2.0;
t1892 = (t1263.*t1495)./2.0;
t1894 = t1891./2.0;
t1898 = t1896./2.0;
t1901 = (t1263.*t1503)./2.0;
t1906 = t1263.*t1534;
t1913 = t1905./2.0;
t1916 = t1907./2.0;
t1918 = t1909./2.0;
t1920 = t1911./2.0;
t1924 = t1041.*t1681;
t1933 = t1930./2.0;
t1937 = t943.*t1761;
t1944 = -t1940;
t1946 = t2.*t1935;
t1950 = t1940./2.0;
t1960 = t1263.*t1602;
t1962 = -t1952;
t1963 = t706+t1279+t1297;
t1966 = t1952./2.0;
t1967 = -t1957;
t1969 = t1956./2.0;
t1970 = t8.*t29.*t1935;
t1972 = t1957./2.0;
t1977 = t1602.*(t384+t472+t477+t26.*t29.*t132.*1.383e-1);
t1989 = -t1984;
t1991 = t1984./2.0;
t1994 = t132.*t1935;
t1998 = -t1992;
t1999 = -t1993;
t2000 = t1992./2.0;
t2001 = t1993./2.0;
t2005 = t1263.*t1648;
t2009 = t2006./2.0;
t2012 = -t2007;
t2014 = -t2010;
t2015 = t2007./2.0;
t2019 = t1264.*t1681;
t2020 = t2010./2.0;
t2022 = t2017.*(-1.0./2.0);
t2024 = -t2016;
t2025 = t2017./2.0;
t2026 = t2016./2.0;
t2027 = t609+t1381+t1389;
t2034 = t808+t1329+t1334;
t2035 = -t2031;
t2037 = t2031./2.0;
t2041 = -t2036;
t2044 = t2036./2.0;
t2048 = -t2.*(t791+t1331+t935.*(t61-t239).*8.084033333333334e-4);
t2051 = t2.*(t791+t1331+t935.*(t61-t239).*8.084033333333334e-4);
t2062 = -t8.*t25.*(t791+t1331+t935.*(t61-t239).*8.084033333333334e-4);
t2064 = -t2061;
t2067 = -t29.*t30.*(t791+t1331+t935.*(t61-t239).*8.084033333333334e-4);
t2069 = t8.*t25.*(t791+t1331+t935.*(t61-t239).*8.084033333333334e-4).*(-1.0./2.0);
t2071 = t29.*t30.*(t791+t1331+t935.*(t61-t239).*8.084033333333334e-4).*(-1.0./2.0);
t2072 = t1263.*t1761;
t2075 = t2073.*2.0;
t2080 = (t1495.*t1602)./2.0;
t2084 = (t1396.*t1681)./2.0;
t2085 = t1503.*t1602;
t2087 = t2082./2.0;
t2093 = t2086./2.0;
t2094 = t692+t1444+t1450;
t2096 = t681+t1451+t1460;
t2101 = t2097./2.0;
t2102 = (t1534.*t1602)./2.0;
t2115 = t2114.*(-1.0./2.0);
t2116 = t2114./2.0;
t2127 = t1535.*t1681;
t2134 = t2130.*(-1.0./2.0);
t2135 = t2131.*(-1.0./2.0);
t2137 = t2130./2.0;
t2138 = t2131./2.0;
t2140 = t2139.*2.0;
t2142 = t2141.*2.0;
t2143 = t1602.*t1648;
t2148 = t2144./2.0;
t2154 = t1603.*t1681;
t2158 = (t1649.*t1681)./2.0;
t2161 = t1602.*t1761;
t2165 = t527+t978+t1008+t1085+t1096;
t2167 = t2162./2.0;
t2174 = t528+t543+t925+t933+t1017+t1019;
t2184 = t1681.*t1762;
t2214 = t603+t627+t986+t996+t1082+t1084;
t2215 = t604+t626+t997+t1005+t1068+t1069;
t2217 = -t8.*(t599+t612-t986-t1082-t1084+t449.*(t60-t190).*8.084033333333334e-4);
t2218 = -t2.*(t600+t610-t997-t1068-t1069+t451.*(t61-t239).*8.084033333333334e-4);
t2221 = t8.*(t599+t612-t986-t1082-t1084+t449.*(t60-t190).*8.084033333333334e-4).*(-1.0./2.0);
t2222 = t2.*(t600+t610-t997-t1068-t1069+t451.*(t61-t239).*8.084033333333334e-4).*(-1.0./2.0);
t2225 = -t8.*t29.*(t600+t610-t997-t1068-t1069+t451.*(t61-t239).*8.084033333333334e-4);
t2226 = -t2.*t29.*(t599+t612-t986-t1082-t1084+t449.*(t60-t190).*8.084033333333334e-4);
t2228 = t8.*t29.*(t600+t610-t997-t1068-t1069+t451.*(t61-t239).*8.084033333333334e-4);
t2230 = t2.*t29.*(t599+t612-t986-t1082-t1084+t449.*(t60-t190).*8.084033333333334e-4).*(-1.0./2.0);
t2231 = t2227./2.0;
t2232 = (t2.*t29.*(t599+t612-t986-t1082-t1084+t449.*(t60-t190).*8.084033333333334e-4))./2.0;
t2233 = -t132.*(t600+t610-t997-t1068-t1069+t451.*(t61-t239).*8.084033333333334e-4);
t2234 = -t171.*(t599+t612-t986-t1082-t1084+t449.*(t60-t190).*8.084033333333334e-4);
t2235 = t132.*(t600+t610-t997-t1068-t1069+t451.*(t61-t239).*8.084033333333334e-4).*(-1.0./2.0);
t2236 = t171.*(t599+t612-t986-t1082-t1084+t449.*(t60-t190).*8.084033333333334e-4).*(-1.0./2.0);
t2239 = t8.*t2238;
t2240 = t2.*t2237;
t2245 = t2.*t29.*t2238;
t2246 = t8.*t29.*t2237;
t2252 = -t8.*(t784-t804-t1142+t1280-t1293+t665.*(t60-t190).*8.084033333333334e-4);
t2254 = t8.*(t784-t804-t1142+t1280-t1293+t665.*(t60-t190).*8.084033333333334e-4).*(-1.0./2.0);
t2257 = t712+t982+t1289+t1291+t1622+t1636;
t2258 = -t25.*(t703+t979-t1289-t1291+t192.*(-t268-t292+t331+t334+t393+t2.*t25.*(t60-t190)).*8.084033333333334e-4+t236.*(-t267-t293+t348+t352+t382+t8.*t25.*(t61-t239)).*8.084033333333334e-4);
t2259 = -t12.*t29.*(t703+t979-t1289-t1291+t192.*(-t268-t292+t331+t334+t393+t2.*t25.*(t60-t190)).*8.084033333333334e-4+t236.*(-t267-t293+t348+t352+t382+t8.*t25.*(t61-t239)).*8.084033333333334e-4);
Y = ft_4({qd1,qd2,qd3,qd4,qd5,qd6,qdd1,qdd2,qdd3,qdd4,qdd5,qdd6,t1000,t1001,t1003,t1006,t1007,t1009,t1012,t1013,t1015,t1016,t1018,t1023,t1026,t1030,t1031,t1036,t1038,t1039,t1040,t1041,t1043,t1048,t1049,t1051,t1054,t1057,t1059,t1061,t1062,t1064,t1065,t1066,t1068,t1069,t1070,t1071,t1072,t1073,t1074,t1077,t1078,t1081,t1082,t1083,t1084,t1086,t1087,t109,t1090,t1091,t1092,t1093,t1094,t1095,t1097,t1099,t1100,t1101,t1102,t1103,t1105,t1108,t1113,t1114,t1115,t1116,t1117,t1120,t1121,t1124,t1125,t1128,t1129,t1130,t1131,t1132,t1133,t1134,t1135,t1138,t1139,t1140,t1141,t1142,t1143,t1146,t1147,t1148,t1149,t1150,t1151,t1152,t1153,t1154,t1155,t1156,t1157,t1159,t1160,t1161,t1162,t1163,t1164,t1165,t1166,t1168,t1169,t1170,t1173,t1174,t1176,t1178,t1179,t1180,t1181,t1182,t1183,t1184,t1185,t1187,t1188,t1189,t1190,t1192,t1193,t1196,t1198,t1199,t12,t1200,t1201,t1202,t1203,t1204,t1206,t1207,t1208,t1209,t1211,t1212,t1213,t1215,t1217,t1218,t1220,t1221,t1223,t1225,t1226,t1227,t1228,t1229,t1230,t1234,t1235,t1236,t1238,t1239,t1242,t1244,t1246,t1247,t1249,t1251,t1252,t1255,t1256,t1259,t1260,t1261,t1262,t1263,t1264,t1265,t1267,t1268,t127,t1270,t1271,t1272,t1274,t1275,t1276,t1277,t1278,t1280,t1281,t1284,t1285,t1286,t1288,t1289,t1290,t1291,t1292,t1293,t1294,t1295,t1296,t1298,t1299,t130,t1300,t1301,t1302,t1303,t1304,t1305,t1306,t1307,t1309,t1310,t1311,t1312,t1313,t1314,t1315,t1316,t1317,t1318,t1319,t132,t1321,t1322,t1323,t1324,t1325,t1327,t1328,t133,t1331,t1332,t1333,t1335,t1336,t1337,t1338,t1339,t1341,t1343,t1344,t1345,t1346,t1347,t1348,t1349,t1350,t1352,t1353,t1354,t1356,t1357,t1358,t1359,t1360,t1361,t1362,t1363,t1365,t1367,t1370,t1371,t1375,t1376,t1377,t1378,t1380,t1382,t1383,t1384,t1385,t1386,t1387,t1388,t1390,t1391,t1392,t1393,t1394,t1395,t1396,t1397,t1398,t1400,t1401,t1402,t1404,t1405,t1406,t1407,t1408,t1409,t1410,t1411,t1413,t1414,t1415,t1416,t1417,t1418,t1419,t1420,t1422,t1423,t1424,t1425,t1426,t1427,t1428,t1429,t1430,t1431,t1432,t1433,t1434,t1435,t1436,t1437,t1439,t144,t1441,t1442,t1443,t1445,t1448,t1449,t1452,t1454,t1455,t1456,t1457,t1458,t146,t1461,t1463,t1464,t1465,t1466,t1467,t1468,t1469,t1470,t1472,t1473,t1474,t1475,t1476,t1478,t1479,t1480,t1482,t1483,t1484,t1485,t1486,t1487,t1488,t1489,t1490,t1491,t1493,t1494,t1495,t1496,t1497,t1498,t1499,t15,t1500,t1501,t1502,t1503,t1505,t1506,t1507,t1508,t151,t1511,t1513,t1514,t1515,t1517,t1518,t1522,t1523,t1525,t1526,t1528,t1531,t1532,t1534,t1535,t1538,t1539,t1540,t1541,t1542,t1543,t1545,t1546,t1548,t1549,t1551,t1553,t1554,t1556,t1557,t1560,t1561,t1562,t1563,t1565,t1568,t1570,t1571,t1572,t1573,t1574,t1575,t1576,t1577,t1578,t1579,t1580,t1583,t1585,t1587,t1588,t1590,t1591,t1592,t1593,t1595,t1596,t1597,t1601,t1602,t1603,t1606,t1608,t1609,t1610,t1612,t1614,t1615,t1616,t1617,t1618,t1619,t1620,t1623,t1624,t1625,t1627,t1628,t1629,t163,t1630,t1631,t1633,t1634,t1637,t1638,t1639,t1640,t1641,t1642,t1643,t1644,t1645,t1646,t1647,t1648,t1649,t1651,t1652,t1653,t1654,t1656,t1657,t1658,t1659,t1660,t1661,t1662,t1663,t1664,t1665,t1668,t1670,t1671,t1672,t1673,t1674,t1676,t1679,t1680,t1681,t1682,t1683,t1685,t1686,t1687,t1688,t1689,t169,t1690,t1691,t1692,t1693,t1695,t1696,t1697,t1698,t1699,t17,t170,t1700,t1701,t1702,t1703,t1704,t1705,t1706,t1708,t1709,t171,t1710,t1711,t1712,t1713,t1714,t1715,t1716,t1717,t1719,t1720,t1721,t1722,t1723,t1724,t1725,t1726,t1727,t1728,t1729,t1730,t1731,t1732,t1733,t1734,t1735,t1736,t1737,t1738,t1739,t1741,t1742,t1744,t1745,t1746,t1747,t1748,t1749,t1750,t1752,t1753,t1754,t1755,t1756,t1759,t1760,t1761,t1762,t1763,t1764,t1766,t1767,t1769,t177,t1770,t1775,t1776,t1778,t1779,t178,t1789,t179,t1793,t1795,t1796,t1797,t1798,t18,t1800,t1801,t1803,t1804,t1806,t1808,t1811,t1814,t1816,t1817,t1819,t1820,t1824,t1825,t1826,t1834,t1837,t1838,t1839,t1845,t1849,t1852,t1863,t1865,t1866,t1868,t1872,t1874,t1877,t1878,t1880,t1884,t1885,t1886,t1888,t1891,t1892,t1893,t1894,t1896,t1898,t190,t1901,t1904,t1905,t1906,t1907,t1908,t1909,t1911,t1912,t1913,t1916,t1918,t192,t1920,t1921,t1922,t1924,t1930,t1931,t1933,t1936,t1937,t1941,t1944,t1945,t1946,t1950,t1951,t1952,t1956,t1958,t1960,t1961,t1963,t1964,t1965,t1966,t1967,t1969,t1970,t1972,t1975,t1977,t1980,t1989,t1991,t1992,t1994,t1999,t2,t20,t2000,t2001,t2005,t2006,t2009,t2012,t2014,t2015,t2017,t2019,t2020,t2024,t2025,t2026,t2027,t2034,t2035,t2037,t2041,t2044,t2051,t2058,t2064,t2071,t2072,t2073,t2075,t2078,t2079,t2080,t2081,t2082,t2084,t2085,t2086,t2087,t2089,t2091,t2093,t2094,t2095,t2097,t2100,t2101,t2102,t2103,t2105,t2106,t211,t2114,t2116,t212,t2127,t2128,t2129,t213,t2130,t2131,t2134,t2135,t2137,t2138,t2139,t214,t2140,t2141,t2142,t2143,t2144,t2148,t2154,t2158,t2161,t2162,t2165,t2167,t2174,t2177,t2179,t2184,t22,t220,t2213,t2216,t2217,t2218,t2221,t2222,t2225,t2227,t2228,t2231,t2232,t2239,t2240,t2245,t2246,t2252,t228,t229,t235,t236,t239,t241,t243,t25,t251,t252,t255,t256,t259,t26,t261,t264,t265,t267,t268,t274,t275,t277,t289,t29,t292,t293,t296,t297,t299,t3,t30,t300,t31,t324,t329,t331,t334,t341,t342,t344,t345,t346,t348,t35,t351,t352,t354,t355,t356,t36,t361,t368,t370,t371,t377,t378,t380,t382,t384,t39,t393,t40,t400,t405,t406,t419,t420,t421,t423,t426,t429,t432,t433,t441,t442,t443,t444,t448,t449,t450,t451,t452,t453,t455,t458,t459,t472,t476,t477,t479,t480,t481,t486,t487,t491,t495,t496,t497,t498,t499,t502,t505,t506,t507,t508,t509,t512,t513,t519,t520,t521,t522,t525,t527,t530,t536,t540,t541,t542,t549,t551,t552,t553,t554,t558,t559,t560,t561,t568,t574,t575,t576,t577,t580,t581,t585,t586,t587,t588,t589,t594,t595,t596,t597,t599,t6,t60,t600,t602,t605,t606,t607,t608,t61,t610,t612,t614,t619,t622,t623,t624,t63,t631,t633,t638,t645,t647,t661,t662,t663,t664,t665,t666,t667,t668,t669,t670,t672,t673,t674,t677,t679,t68,t681,t682,t685,t688,t691,t693,t694,t695,t696,t697,t698,t699,t7,t702,t703,t704,t705,t708,t71,t710,t711,t712,t713,t716,t718,t721,t722,t723,t724,t725,t726,t727,t728,t729,t730,t731,t742,t743,t744,t75,t750,t752,t753,t754,t755,t757,t760,t765,t768,t773,t774,t775,t776,t777,t778,t782,t783,t784,t785,t786,t787,t788,t789,t79,t790,t791,t792,t793,t794,t795,t796,t798,t8,t801,t802,t803,t804,t805,t806,t809,t812,t813,t814,t815,t817,t818,t821,t822,t824,t825,t826,t827,t828,t829,t830,t831,t834,t835,t836,t837,t838,t852,t862,t871,t873,t874,t875,t876,t881,t882,t883,t884,t885,t887,t888,t889,t890,t891,t895,t896,t897,t898,t9,t900,t902,t903,t904,t905,t906,t907,t908,t909,t911,t912,t914,t915,t916,t917,t918,t919,t92,t923,t924,t926,t932,t934,t935,t936,t937,t938,t941,t942,t943,t948,t950,t952,t953,t955,t956,t962,t965,t966,t967,t968,t969,t970,t972,t973,t974,t975,t977,t979,t980,t981,t982,t983,t986,t987,t988,t989,t990,t991,t992,t993,t994,t995,t997,t998,t999});
end
function Y = ft_4(ct)
qd1 = ct{1};
qd2 = ct{2};
qd3 = ct{3};
qd4 = ct{4};
qd5 = ct{5};
qd6 = ct{6};
qdd1 = ct{7};
qdd2 = ct{8};
qdd3 = ct{9};
qdd4 = ct{10};
qdd5 = ct{11};
qdd6 = ct{12};
t1000 = ct{13};
t1001 = ct{14};
t1003 = ct{15};
t1006 = ct{16};
t1007 = ct{17};
t1009 = ct{18};
t1012 = ct{19};
t1013 = ct{20};
t1015 = ct{21};
t1016 = ct{22};
t1018 = ct{23};
t1023 = ct{24};
t1026 = ct{25};
t1030 = ct{26};
t1031 = ct{27};
t1036 = ct{28};
t1038 = ct{29};
t1039 = ct{30};
t1040 = ct{31};
t1041 = ct{32};
t1043 = ct{33};
t1048 = ct{34};
t1049 = ct{35};
t1051 = ct{36};
t1054 = ct{37};
t1057 = ct{38};
t1059 = ct{39};
t1061 = ct{40};
t1062 = ct{41};
t1064 = ct{42};
t1065 = ct{43};
t1066 = ct{44};
t1068 = ct{45};
t1069 = ct{46};
t1070 = ct{47};
t1071 = ct{48};
t1072 = ct{49};
t1073 = ct{50};
t1074 = ct{51};
t1077 = ct{52};
t1078 = ct{53};
t1081 = ct{54};
t1082 = ct{55};
t1083 = ct{56};
t1084 = ct{57};
t1086 = ct{58};
t1087 = ct{59};
t109 = ct{60};
t1090 = ct{61};
t1091 = ct{62};
t1092 = ct{63};
t1093 = ct{64};
t1094 = ct{65};
t1095 = ct{66};
t1097 = ct{67};
t1099 = ct{68};
t1100 = ct{69};
t1101 = ct{70};
t1102 = ct{71};
t1103 = ct{72};
t1105 = ct{73};
t1108 = ct{74};
t1113 = ct{75};
t1114 = ct{76};
t1115 = ct{77};
t1116 = ct{78};
t1117 = ct{79};
t1120 = ct{80};
t1121 = ct{81};
t1124 = ct{82};
t1125 = ct{83};
t1128 = ct{84};
t1129 = ct{85};
t1130 = ct{86};
t1131 = ct{87};
t1132 = ct{88};
t1133 = ct{89};
t1134 = ct{90};
t1135 = ct{91};
t1138 = ct{92};
t1139 = ct{93};
t1140 = ct{94};
t1141 = ct{95};
t1142 = ct{96};
t1143 = ct{97};
t1146 = ct{98};
t1147 = ct{99};
t1148 = ct{100};
t1149 = ct{101};
t1150 = ct{102};
t1151 = ct{103};
t1152 = ct{104};
t1153 = ct{105};
t1154 = ct{106};
t1155 = ct{107};
t1156 = ct{108};
t1157 = ct{109};
t1159 = ct{110};
t1160 = ct{111};
t1161 = ct{112};
t1162 = ct{113};
t1163 = ct{114};
t1164 = ct{115};
t1165 = ct{116};
t1166 = ct{117};
t1168 = ct{118};
t1169 = ct{119};
t1170 = ct{120};
t1173 = ct{121};
t1174 = ct{122};
t1176 = ct{123};
t1178 = ct{124};
t1179 = ct{125};
t1180 = ct{126};
t1181 = ct{127};
t1182 = ct{128};
t1183 = ct{129};
t1184 = ct{130};
t1185 = ct{131};
t1187 = ct{132};
t1188 = ct{133};
t1189 = ct{134};
t1190 = ct{135};
t1192 = ct{136};
t1193 = ct{137};
t1196 = ct{138};
t1198 = ct{139};
t1199 = ct{140};
t12 = ct{141};
t1200 = ct{142};
t1201 = ct{143};
t1202 = ct{144};
t1203 = ct{145};
t1204 = ct{146};
t1206 = ct{147};
t1207 = ct{148};
t1208 = ct{149};
t1209 = ct{150};
t1211 = ct{151};
t1212 = ct{152};
t1213 = ct{153};
t1215 = ct{154};
t1217 = ct{155};
t1218 = ct{156};
t1220 = ct{157};
t1221 = ct{158};
t1223 = ct{159};
t1225 = ct{160};
t1226 = ct{161};
t1227 = ct{162};
t1228 = ct{163};
t1229 = ct{164};
t1230 = ct{165};
t1234 = ct{166};
t1235 = ct{167};
t1236 = ct{168};
t1238 = ct{169};
t1239 = ct{170};
t1242 = ct{171};
t1244 = ct{172};
t1246 = ct{173};
t1247 = ct{174};
t1249 = ct{175};
t1251 = ct{176};
t1252 = ct{177};
t1255 = ct{178};
t1256 = ct{179};
t1259 = ct{180};
t1260 = ct{181};
t1261 = ct{182};
t1262 = ct{183};
t1263 = ct{184};
t1264 = ct{185};
t1265 = ct{186};
t1267 = ct{187};
t1268 = ct{188};
t127 = ct{189};
t1270 = ct{190};
t1271 = ct{191};
t1272 = ct{192};
t1274 = ct{193};
t1275 = ct{194};
t1276 = ct{195};
t1277 = ct{196};
t1278 = ct{197};
t1280 = ct{198};
t1281 = ct{199};
t1284 = ct{200};
t1285 = ct{201};
t1286 = ct{202};
t1288 = ct{203};
t1289 = ct{204};
t1290 = ct{205};
t1291 = ct{206};
t1292 = ct{207};
t1293 = ct{208};
t1294 = ct{209};
t1295 = ct{210};
t1296 = ct{211};
t1298 = ct{212};
t1299 = ct{213};
t130 = ct{214};
t1300 = ct{215};
t1301 = ct{216};
t1302 = ct{217};
t1303 = ct{218};
t1304 = ct{219};
t1305 = ct{220};
t1306 = ct{221};
t1307 = ct{222};
t1309 = ct{223};
t1310 = ct{224};
t1311 = ct{225};
t1312 = ct{226};
t1313 = ct{227};
t1314 = ct{228};
t1315 = ct{229};
t1316 = ct{230};
t1317 = ct{231};
t1318 = ct{232};
t1319 = ct{233};
t132 = ct{234};
t1321 = ct{235};
t1322 = ct{236};
t1323 = ct{237};
t1324 = ct{238};
t1325 = ct{239};
t1327 = ct{240};
t1328 = ct{241};
t133 = ct{242};
t1331 = ct{243};
t1332 = ct{244};
t1333 = ct{245};
t1335 = ct{246};
t1336 = ct{247};
t1337 = ct{248};
t1338 = ct{249};
t1339 = ct{250};
t1341 = ct{251};
t1343 = ct{252};
t1344 = ct{253};
t1345 = ct{254};
t1346 = ct{255};
t1347 = ct{256};
t1348 = ct{257};
t1349 = ct{258};
t1350 = ct{259};
t1352 = ct{260};
t1353 = ct{261};
t1354 = ct{262};
t1356 = ct{263};
t1357 = ct{264};
t1358 = ct{265};
t1359 = ct{266};
t1360 = ct{267};
t1361 = ct{268};
t1362 = ct{269};
t1363 = ct{270};
t1365 = ct{271};
t1367 = ct{272};
t1370 = ct{273};
t1371 = ct{274};
t1375 = ct{275};
t1376 = ct{276};
t1377 = ct{277};
t1378 = ct{278};
t1380 = ct{279};
t1382 = ct{280};
t1383 = ct{281};
t1384 = ct{282};
t1385 = ct{283};
t1386 = ct{284};
t1387 = ct{285};
t1388 = ct{286};
t1390 = ct{287};
t1391 = ct{288};
t1392 = ct{289};
t1393 = ct{290};
t1394 = ct{291};
t1395 = ct{292};
t1396 = ct{293};
t1397 = ct{294};
t1398 = ct{295};
t1400 = ct{296};
t1401 = ct{297};
t1402 = ct{298};
t1404 = ct{299};
t1405 = ct{300};
t1406 = ct{301};
t1407 = ct{302};
t1408 = ct{303};
t1409 = ct{304};
t1410 = ct{305};
t1411 = ct{306};
t1413 = ct{307};
t1414 = ct{308};
t1415 = ct{309};
t1416 = ct{310};
t1417 = ct{311};
t1418 = ct{312};
t1419 = ct{313};
t1420 = ct{314};
t1422 = ct{315};
t1423 = ct{316};
t1424 = ct{317};
t1425 = ct{318};
t1426 = ct{319};
t1427 = ct{320};
t1428 = ct{321};
t1429 = ct{322};
t1430 = ct{323};
t1431 = ct{324};
t1432 = ct{325};
t1433 = ct{326};
t1434 = ct{327};
t1435 = ct{328};
t1436 = ct{329};
t1437 = ct{330};
t1439 = ct{331};
t144 = ct{332};
t1441 = ct{333};
t1442 = ct{334};
t1443 = ct{335};
t1445 = ct{336};
t1448 = ct{337};
t1449 = ct{338};
t1452 = ct{339};
t1454 = ct{340};
t1455 = ct{341};
t1456 = ct{342};
t1457 = ct{343};
t1458 = ct{344};
t146 = ct{345};
t1461 = ct{346};
t1463 = ct{347};
t1464 = ct{348};
t1465 = ct{349};
t1466 = ct{350};
t1467 = ct{351};
t1468 = ct{352};
t1469 = ct{353};
t1470 = ct{354};
t1472 = ct{355};
t1473 = ct{356};
t1474 = ct{357};
t1475 = ct{358};
t1476 = ct{359};
t1478 = ct{360};
t1479 = ct{361};
t1480 = ct{362};
t1482 = ct{363};
t1483 = ct{364};
t1484 = ct{365};
t1485 = ct{366};
t1486 = ct{367};
t1487 = ct{368};
t1488 = ct{369};
t1489 = ct{370};
t1490 = ct{371};
t1491 = ct{372};
t1493 = ct{373};
t1494 = ct{374};
t1495 = ct{375};
t1496 = ct{376};
t1497 = ct{377};
t1498 = ct{378};
t1499 = ct{379};
t15 = ct{380};
t1500 = ct{381};
t1501 = ct{382};
t1502 = ct{383};
t1503 = ct{384};
t1505 = ct{385};
t1506 = ct{386};
t1507 = ct{387};
t1508 = ct{388};
t151 = ct{389};
t1511 = ct{390};
t1513 = ct{391};
t1514 = ct{392};
t1515 = ct{393};
t1517 = ct{394};
t1518 = ct{395};
t1522 = ct{396};
t1523 = ct{397};
t1525 = ct{398};
t1526 = ct{399};
t1528 = ct{400};
t1531 = ct{401};
t1532 = ct{402};
t1534 = ct{403};
t1535 = ct{404};
t1538 = ct{405};
t1539 = ct{406};
t1540 = ct{407};
t1541 = ct{408};
t1542 = ct{409};
t1543 = ct{410};
t1545 = ct{411};
t1546 = ct{412};
t1548 = ct{413};
t1549 = ct{414};
t1551 = ct{415};
t1553 = ct{416};
t1554 = ct{417};
t1556 = ct{418};
t1557 = ct{419};
t1560 = ct{420};
t1561 = ct{421};
t1562 = ct{422};
t1563 = ct{423};
t1565 = ct{424};
t1568 = ct{425};
t1570 = ct{426};
t1571 = ct{427};
t1572 = ct{428};
t1573 = ct{429};
t1574 = ct{430};
t1575 = ct{431};
t1576 = ct{432};
t1577 = ct{433};
t1578 = ct{434};
t1579 = ct{435};
t1580 = ct{436};
t1583 = ct{437};
t1585 = ct{438};
t1587 = ct{439};
t1588 = ct{440};
t1590 = ct{441};
t1591 = ct{442};
t1592 = ct{443};
t1593 = ct{444};
t1595 = ct{445};
t1596 = ct{446};
t1597 = ct{447};
t1601 = ct{448};
t1602 = ct{449};
t1603 = ct{450};
t1606 = ct{451};
t1608 = ct{452};
t1609 = ct{453};
t1610 = ct{454};
t1612 = ct{455};
t1614 = ct{456};
t1615 = ct{457};
t1616 = ct{458};
t1617 = ct{459};
t1618 = ct{460};
t1619 = ct{461};
t1620 = ct{462};
t1623 = ct{463};
t1624 = ct{464};
t1625 = ct{465};
t1627 = ct{466};
t1628 = ct{467};
t1629 = ct{468};
t163 = ct{469};
t1630 = ct{470};
t1631 = ct{471};
t1633 = ct{472};
t1634 = ct{473};
t1637 = ct{474};
t1638 = ct{475};
t1639 = ct{476};
t1640 = ct{477};
t1641 = ct{478};
t1642 = ct{479};
t1643 = ct{480};
t1644 = ct{481};
t1645 = ct{482};
t1646 = ct{483};
t1647 = ct{484};
t1648 = ct{485};
t1649 = ct{486};
t1651 = ct{487};
t1652 = ct{488};
t1653 = ct{489};
t1654 = ct{490};
t1656 = ct{491};
t1657 = ct{492};
t1658 = ct{493};
t1659 = ct{494};
t1660 = ct{495};
t1661 = ct{496};
t1662 = ct{497};
t1663 = ct{498};
t1664 = ct{499};
t1665 = ct{500};
t1668 = ct{501};
t1670 = ct{502};
t1671 = ct{503};
t1672 = ct{504};
t1673 = ct{505};
t1674 = ct{506};
t1676 = ct{507};
t1679 = ct{508};
t1680 = ct{509};
t1681 = ct{510};
t1682 = ct{511};
t1683 = ct{512};
t1685 = ct{513};
t1686 = ct{514};
t1687 = ct{515};
t1688 = ct{516};
t1689 = ct{517};
t169 = ct{518};
t1690 = ct{519};
t1691 = ct{520};
t1692 = ct{521};
t1693 = ct{522};
t1695 = ct{523};
t1696 = ct{524};
t1697 = ct{525};
t1698 = ct{526};
t1699 = ct{527};
t17 = ct{528};
t170 = ct{529};
t1700 = ct{530};
t1701 = ct{531};
t1702 = ct{532};
t1703 = ct{533};
t1704 = ct{534};
t1705 = ct{535};
t1706 = ct{536};
t1708 = ct{537};
t1709 = ct{538};
t171 = ct{539};
t1710 = ct{540};
t1711 = ct{541};
t1712 = ct{542};
t1713 = ct{543};
t1714 = ct{544};
t1715 = ct{545};
t1716 = ct{546};
t1717 = ct{547};
t1719 = ct{548};
t1720 = ct{549};
t1721 = ct{550};
t1722 = ct{551};
t1723 = ct{552};
t1724 = ct{553};
t1725 = ct{554};
t1726 = ct{555};
t1727 = ct{556};
t1728 = ct{557};
t1729 = ct{558};
t1730 = ct{559};
t1731 = ct{560};
t1732 = ct{561};
t1733 = ct{562};
t1734 = ct{563};
t1735 = ct{564};
t1736 = ct{565};
t1737 = ct{566};
t1738 = ct{567};
t1739 = ct{568};
t1741 = ct{569};
t1742 = ct{570};
t1744 = ct{571};
t1745 = ct{572};
t1746 = ct{573};
t1747 = ct{574};
t1748 = ct{575};
t1749 = ct{576};
t1750 = ct{577};
t1752 = ct{578};
t1753 = ct{579};
t1754 = ct{580};
t1755 = ct{581};
t1756 = ct{582};
t1759 = ct{583};
t1760 = ct{584};
t1761 = ct{585};
t1762 = ct{586};
t1763 = ct{587};
t1764 = ct{588};
t1766 = ct{589};
t1767 = ct{590};
t1769 = ct{591};
t177 = ct{592};
t1770 = ct{593};
t1775 = ct{594};
t1776 = ct{595};
t1778 = ct{596};
t1779 = ct{597};
t178 = ct{598};
t1789 = ct{599};
t179 = ct{600};
t1793 = ct{601};
t1795 = ct{602};
t1796 = ct{603};
t1797 = ct{604};
t1798 = ct{605};
t18 = ct{606};
t1800 = ct{607};
t1801 = ct{608};
t1803 = ct{609};
t1804 = ct{610};
t1806 = ct{611};
t1808 = ct{612};
t1811 = ct{613};
t1814 = ct{614};
t1816 = ct{615};
t1817 = ct{616};
t1819 = ct{617};
t1820 = ct{618};
t1824 = ct{619};
t1825 = ct{620};
t1826 = ct{621};
t1834 = ct{622};
t1837 = ct{623};
t1838 = ct{624};
t1839 = ct{625};
t1845 = ct{626};
t1849 = ct{627};
t1852 = ct{628};
t1863 = ct{629};
t1865 = ct{630};
t1866 = ct{631};
t1868 = ct{632};
t1872 = ct{633};
t1874 = ct{634};
t1877 = ct{635};
t1878 = ct{636};
t1880 = ct{637};
t1884 = ct{638};
t1885 = ct{639};
t1886 = ct{640};
t1888 = ct{641};
t1891 = ct{642};
t1892 = ct{643};
t1893 = ct{644};
t1894 = ct{645};
t1896 = ct{646};
t1898 = ct{647};
t190 = ct{648};
t1901 = ct{649};
t1904 = ct{650};
t1905 = ct{651};
t1906 = ct{652};
t1907 = ct{653};
t1908 = ct{654};
t1909 = ct{655};
t1911 = ct{656};
t1912 = ct{657};
t1913 = ct{658};
t1916 = ct{659};
t1918 = ct{660};
t192 = ct{661};
t1920 = ct{662};
t1921 = ct{663};
t1922 = ct{664};
t1924 = ct{665};
t1930 = ct{666};
t1931 = ct{667};
t1933 = ct{668};
t1936 = ct{669};
t1937 = ct{670};
t1941 = ct{671};
t1944 = ct{672};
t1945 = ct{673};
t1946 = ct{674};
t1950 = ct{675};
t1951 = ct{676};
t1952 = ct{677};
t1956 = ct{678};
t1958 = ct{679};
t1960 = ct{680};
t1961 = ct{681};
t1963 = ct{682};
t1964 = ct{683};
t1965 = ct{684};
t1966 = ct{685};
t1967 = ct{686};
t1969 = ct{687};
t1970 = ct{688};
t1972 = ct{689};
t1975 = ct{690};
t1977 = ct{691};
t1980 = ct{692};
t1989 = ct{693};
t1991 = ct{694};
t1992 = ct{695};
t1994 = ct{696};
t1999 = ct{697};
t2 = ct{698};
t20 = ct{699};
t2000 = ct{700};
t2001 = ct{701};
t2005 = ct{702};
t2006 = ct{703};
t2009 = ct{704};
t2012 = ct{705};
t2014 = ct{706};
t2015 = ct{707};
t2017 = ct{708};
t2019 = ct{709};
t2020 = ct{710};
t2024 = ct{711};
t2025 = ct{712};
t2026 = ct{713};
t2027 = ct{714};
t2034 = ct{715};
t2035 = ct{716};
t2037 = ct{717};
t2041 = ct{718};
t2044 = ct{719};
t2051 = ct{720};
t2058 = ct{721};
t2064 = ct{722};
t2071 = ct{723};
t2072 = ct{724};
t2073 = ct{725};
t2075 = ct{726};
t2078 = ct{727};
t2079 = ct{728};
t2080 = ct{729};
t2081 = ct{730};
t2082 = ct{731};
t2084 = ct{732};
t2085 = ct{733};
t2086 = ct{734};
t2087 = ct{735};
t2089 = ct{736};
t2091 = ct{737};
t2093 = ct{738};
t2094 = ct{739};
t2095 = ct{740};
t2097 = ct{741};
t2100 = ct{742};
t2101 = ct{743};
t2102 = ct{744};
t2103 = ct{745};
t2105 = ct{746};
t2106 = ct{747};
t211 = ct{748};
t2114 = ct{749};
t2116 = ct{750};
t212 = ct{751};
t2127 = ct{752};
t2128 = ct{753};
t2129 = ct{754};
t213 = ct{755};
t2130 = ct{756};
t2131 = ct{757};
t2134 = ct{758};
t2135 = ct{759};
t2137 = ct{760};
t2138 = ct{761};
t2139 = ct{762};
t214 = ct{763};
t2140 = ct{764};
t2141 = ct{765};
t2142 = ct{766};
t2143 = ct{767};
t2144 = ct{768};
t2148 = ct{769};
t2154 = ct{770};
t2158 = ct{771};
t2161 = ct{772};
t2162 = ct{773};
t2165 = ct{774};
t2167 = ct{775};
t2174 = ct{776};
t2177 = ct{777};
t2179 = ct{778};
t2184 = ct{779};
t22 = ct{780};
t220 = ct{781};
t2213 = ct{782};
t2216 = ct{783};
t2217 = ct{784};
t2218 = ct{785};
t2221 = ct{786};
t2222 = ct{787};
t2225 = ct{788};
t2227 = ct{789};
t2228 = ct{790};
t2231 = ct{791};
t2232 = ct{792};
t2239 = ct{793};
t2240 = ct{794};
t2245 = ct{795};
t2246 = ct{796};
t2252 = ct{797};
t228 = ct{798};
t229 = ct{799};
t235 = ct{800};
t236 = ct{801};
t239 = ct{802};
t241 = ct{803};
t243 = ct{804};
t25 = ct{805};
t251 = ct{806};
t252 = ct{807};
t255 = ct{808};
t256 = ct{809};
t259 = ct{810};
t26 = ct{811};
t261 = ct{812};
t264 = ct{813};
t265 = ct{814};
t267 = ct{815};
t268 = ct{816};
t274 = ct{817};
t275 = ct{818};
t277 = ct{819};
t289 = ct{820};
t29 = ct{821};
t292 = ct{822};
t293 = ct{823};
t296 = ct{824};
t297 = ct{825};
t299 = ct{826};
t3 = ct{827};
t30 = ct{828};
t300 = ct{829};
t31 = ct{830};
t324 = ct{831};
t329 = ct{832};
t331 = ct{833};
t334 = ct{834};
t341 = ct{835};
t342 = ct{836};
t344 = ct{837};
t345 = ct{838};
t346 = ct{839};
t348 = ct{840};
t35 = ct{841};
t351 = ct{842};
t352 = ct{843};
t354 = ct{844};
t355 = ct{845};
t356 = ct{846};
t36 = ct{847};
t361 = ct{848};
t368 = ct{849};
t370 = ct{850};
t371 = ct{851};
t377 = ct{852};
t378 = ct{853};
t380 = ct{854};
t382 = ct{855};
t384 = ct{856};
t39 = ct{857};
t393 = ct{858};
t40 = ct{859};
t400 = ct{860};
t405 = ct{861};
t406 = ct{862};
t419 = ct{863};
t420 = ct{864};
t421 = ct{865};
t423 = ct{866};
t426 = ct{867};
t429 = ct{868};
t432 = ct{869};
t433 = ct{870};
t441 = ct{871};
t442 = ct{872};
t443 = ct{873};
t444 = ct{874};
t448 = ct{875};
t449 = ct{876};
t450 = ct{877};
t451 = ct{878};
t452 = ct{879};
t453 = ct{880};
t455 = ct{881};
t458 = ct{882};
t459 = ct{883};
t472 = ct{884};
t476 = ct{885};
t477 = ct{886};
t479 = ct{887};
t480 = ct{888};
t481 = ct{889};
t486 = ct{890};
t487 = ct{891};
t491 = ct{892};
t495 = ct{893};
t496 = ct{894};
t497 = ct{895};
t498 = ct{896};
t499 = ct{897};
t502 = ct{898};
t505 = ct{899};
t506 = ct{900};
t507 = ct{901};
t508 = ct{902};
t509 = ct{903};
t512 = ct{904};
t513 = ct{905};
t519 = ct{906};
t520 = ct{907};
t521 = ct{908};
t522 = ct{909};
t525 = ct{910};
t527 = ct{911};
t530 = ct{912};
t536 = ct{913};
t540 = ct{914};
t541 = ct{915};
t542 = ct{916};
t549 = ct{917};
t551 = ct{918};
t552 = ct{919};
t553 = ct{920};
t554 = ct{921};
t558 = ct{922};
t559 = ct{923};
t560 = ct{924};
t561 = ct{925};
t568 = ct{926};
t574 = ct{927};
t575 = ct{928};
t576 = ct{929};
t577 = ct{930};
t580 = ct{931};
t581 = ct{932};
t585 = ct{933};
t586 = ct{934};
t587 = ct{935};
t588 = ct{936};
t589 = ct{937};
t594 = ct{938};
t595 = ct{939};
t596 = ct{940};
t597 = ct{941};
t599 = ct{942};
t6 = ct{943};
t60 = ct{944};
t600 = ct{945};
t602 = ct{946};
t605 = ct{947};
t606 = ct{948};
t607 = ct{949};
t608 = ct{950};
t61 = ct{951};
t610 = ct{952};
t612 = ct{953};
t614 = ct{954};
t619 = ct{955};
t622 = ct{956};
t623 = ct{957};
t624 = ct{958};
t63 = ct{959};
t631 = ct{960};
t633 = ct{961};
t638 = ct{962};
t645 = ct{963};
t647 = ct{964};
t661 = ct{965};
t662 = ct{966};
t663 = ct{967};
t664 = ct{968};
t665 = ct{969};
t666 = ct{970};
t667 = ct{971};
t668 = ct{972};
t669 = ct{973};
t670 = ct{974};
t672 = ct{975};
t673 = ct{976};
t674 = ct{977};
t677 = ct{978};
t679 = ct{979};
t68 = ct{980};
t681 = ct{981};
t682 = ct{982};
t685 = ct{983};
t688 = ct{984};
t691 = ct{985};
t693 = ct{986};
t694 = ct{987};
t695 = ct{988};
t696 = ct{989};
t697 = ct{990};
t698 = ct{991};
t699 = ct{992};
t7 = ct{993};
t702 = ct{994};
t703 = ct{995};
t704 = ct{996};
t705 = ct{997};
t708 = ct{998};
t71 = ct{999};
t710 = ct{1000};
t711 = ct{1001};
t712 = ct{1002};
t713 = ct{1003};
t716 = ct{1004};
t718 = ct{1005};
t721 = ct{1006};
t722 = ct{1007};
t723 = ct{1008};
t724 = ct{1009};
t725 = ct{1010};
t726 = ct{1011};
t727 = ct{1012};
t728 = ct{1013};
t729 = ct{1014};
t730 = ct{1015};
t731 = ct{1016};
t742 = ct{1017};
t743 = ct{1018};
t744 = ct{1019};
t75 = ct{1020};
t750 = ct{1021};
t752 = ct{1022};
t753 = ct{1023};
t754 = ct{1024};
t755 = ct{1025};
t757 = ct{1026};
t760 = ct{1027};
t765 = ct{1028};
t768 = ct{1029};
t773 = ct{1030};
t774 = ct{1031};
t775 = ct{1032};
t776 = ct{1033};
t777 = ct{1034};
t778 = ct{1035};
t782 = ct{1036};
t783 = ct{1037};
t784 = ct{1038};
t785 = ct{1039};
t786 = ct{1040};
t787 = ct{1041};
t788 = ct{1042};
t789 = ct{1043};
t79 = ct{1044};
t790 = ct{1045};
t791 = ct{1046};
t792 = ct{1047};
t793 = ct{1048};
t794 = ct{1049};
t795 = ct{1050};
t796 = ct{1051};
t798 = ct{1052};
t8 = ct{1053};
t801 = ct{1054};
t802 = ct{1055};
t803 = ct{1056};
t804 = ct{1057};
t805 = ct{1058};
t806 = ct{1059};
t809 = ct{1060};
t812 = ct{1061};
t813 = ct{1062};
t814 = ct{1063};
t815 = ct{1064};
t817 = ct{1065};
t818 = ct{1066};
t821 = ct{1067};
t822 = ct{1068};
t824 = ct{1069};
t825 = ct{1070};
t826 = ct{1071};
t827 = ct{1072};
t828 = ct{1073};
t829 = ct{1074};
t830 = ct{1075};
t831 = ct{1076};
t834 = ct{1077};
t835 = ct{1078};
t836 = ct{1079};
t837 = ct{1080};
t838 = ct{1081};
t852 = ct{1082};
t862 = ct{1083};
t871 = ct{1084};
t873 = ct{1085};
t874 = ct{1086};
t875 = ct{1087};
t876 = ct{1088};
t881 = ct{1089};
t882 = ct{1090};
t883 = ct{1091};
t884 = ct{1092};
t885 = ct{1093};
t887 = ct{1094};
t888 = ct{1095};
t889 = ct{1096};
t890 = ct{1097};
t891 = ct{1098};
t895 = ct{1099};
t896 = ct{1100};
t897 = ct{1101};
t898 = ct{1102};
t9 = ct{1103};
t900 = ct{1104};
t902 = ct{1105};
t903 = ct{1106};
t904 = ct{1107};
t905 = ct{1108};
t906 = ct{1109};
t907 = ct{1110};
t908 = ct{1111};
t909 = ct{1112};
t911 = ct{1113};
t912 = ct{1114};
t914 = ct{1115};
t915 = ct{1116};
t916 = ct{1117};
t917 = ct{1118};
t918 = ct{1119};
t919 = ct{1120};
t92 = ct{1121};
t923 = ct{1122};
t924 = ct{1123};
t926 = ct{1124};
t932 = ct{1125};
t934 = ct{1126};
t935 = ct{1127};
t936 = ct{1128};
t937 = ct{1129};
t938 = ct{1130};
t941 = ct{1131};
t942 = ct{1132};
t943 = ct{1133};
t948 = ct{1134};
t950 = ct{1135};
t952 = ct{1136};
t953 = ct{1137};
t955 = ct{1138};
t956 = ct{1139};
t962 = ct{1140};
t965 = ct{1141};
t966 = ct{1142};
t967 = ct{1143};
t968 = ct{1144};
t969 = ct{1145};
t970 = ct{1146};
t972 = ct{1147};
t973 = ct{1148};
t974 = ct{1149};
t975 = ct{1150};
t977 = ct{1151};
t979 = ct{1152};
t980 = ct{1153};
t981 = ct{1154};
t982 = ct{1155};
t983 = ct{1156};
t986 = ct{1157};
t987 = ct{1158};
t988 = ct{1159};
t989 = ct{1160};
t990 = ct{1161};
t991 = ct{1162};
t992 = ct{1163};
t993 = ct{1164};
t994 = ct{1165};
t995 = ct{1166};
t997 = ct{1167};
t998 = ct{1168};
t999 = ct{1169};
t2260 = t25.*(t703+t979-t1289-t1291+t192.*(-t268-t292+t331+t334+t393+t2.*t25.*(t60-t190)).*8.084033333333334e-4+t236.*(-t267-t293+t348+t352+t382+t8.*t25.*(t61-t239)).*8.084033333333334e-4).*(-1.0./2.0);
t2261 = t12.*t29.*(t703+t979-t1289-t1291+t192.*(-t268-t292+t331+t334+t393+t2.*t25.*(t60-t190)).*8.084033333333334e-4+t236.*(-t267-t293+t348+t352+t382+t8.*t25.*(t61-t239)).*8.084033333333334e-4).*(-1.0./2.0);
t2265 = -t8.*(t682+t941-t1378-t1624+t1370.*(t60-t190).*8.084033333333334e-4+t7.*t171.*(t289-t476+t171.*(t60-t190)).*8.084033333333334e-4);
t2267 = t8.*(t682+t941-t1378-t1624+t1370.*(t60-t190).*8.084033333333334e-4+t7.*t171.*(t289-t476+t171.*(t60-t190)).*8.084033333333334e-4).*(-1.0./2.0);
t2270 = t725+t1051+t1295+t1310+t1654+t1671;
t2271 = t728+t1048+t1296+t1311+t1660+t1682;
t2301 = t631+t871+t1413+t1417+t1754+t1760;
t2305 = -t2.*(t633-t852+t1418+t1752+t1545.*(t61-t239).*8.084033333333334e-4+t252.*(t289-t476+t171.*(t60-t190)).*8.084033333333334e-4);
t2308 = t2.*(t633-t852+t1418+t1752+t1545.*(t61-t239).*8.084033333333334e-4+t252.*(t289-t476+t171.*(t60-t190)).*8.084033333333334e-4).*(-1.0./2.0);
t2310 = (t2.*(t633-t852+t1418+t1752+t1545.*(t61-t239).*8.084033333333334e-4+t252.*(t289-t476+t171.*(t60-t190)).*8.084033333333334e-4))./2.0;
t2312 = -t8.*t29.*(t633-t852+t1418+t1752+t1545.*(t61-t239).*8.084033333333334e-4+t252.*(t289-t476+t171.*(t60-t190)).*8.084033333333334e-4);
t2314 = t8.*t29.*(t633-t852+t1418+t1752+t1545.*(t61-t239).*8.084033333333334e-4+t252.*(t289-t476+t171.*(t60-t190)).*8.084033333333334e-4).*(-1.0./2.0);
t2316 = -t132.*(t633-t852+t1418+t1752+t1545.*(t61-t239).*8.084033333333334e-4+t252.*(t289-t476+t171.*(t60-t190)).*8.084033333333334e-4);
t2318 = t132.*(t633-t852+t1418+t1752+t1545.*(t61-t239).*8.084033333333334e-4+t252.*(t289-t476+t171.*(t60-t190)).*8.084033333333334e-4).*(-1.0./2.0);
t1216 = t1193./2.0;
t1224 = -t1218;
t1320 = -t1312;
t1326 = -t1324;
t1379 = t1361./2.0;
t1399 = -t1388;
t1421 = -t1416;
t1492 = -t1488;
t1537 = -t1531;
t1567 = -t1562;
t1582 = -t1580;
t1586 = -t1583;
t1594 = t1588./2.0;
t1599 = -t1595;
t1600 = -t1596;
t1611 = -t1606;
t1613 = t1606./2.0;
t1650 = -t1644;
t1669 = -t1661;
t1707 = -t1702;
t1718 = -t1717;
t1740 = t1732./2.0;
t1743 = -t1741;
t1757 = -t1749;
t1771 = t1766./2.0;
t1773 = t1767./2.0;
t1780 = t530+t1087+t1094;
t1792 = t1249+t1272;
t1799 = -t1796;
t1802 = t211+t212+t444+t458+t1473;
t1805 = t1796./2.0;
t1810 = -t1806;
t1812 = t1804./2.0;
t1821 = t8.*t1819;
t1822 = t2.*t1820;
t1823 = t721.*t1680;
t1829 = t2.*t25.*t1819;
t1830 = t2.*t29.*t1819;
t1832 = -t1824;
t1836 = t1824./2.0;
t1840 = t26.*t29.*t1819;
t1843 = t8.*t25.*t1820;
t1844 = t1825./2.0;
t1846 = t8.*t29.*t1820;
t1854 = t29.*t30.*t1820;
t1862 = t133.*t1819;
t1864 = (t789.*t1680)./2.0;
t1869 = t171.*t1819;
t1871 = t132.*t1820;
t1876 = t170.*t1820;
t1887 = t1884./2.0;
t1890 = -t1888;
t1900 = t943.*t1680;
t1914 = -t1913;
t1915 = t1906./2.0;
t1923 = t1040.*t1680;
t1925 = -t1924;
t1927 = t1924./2.0;
t1934 = -t1933;
t1939 = t722.*t1793;
t1947 = t1937./2.0;
t1955 = -t1950;
t1959 = t1946./2.0;
t1971 = -t1966;
t1973 = -t1969;
t1974 = -t1972;
t1976 = -t1970;
t1979 = (t790.*t1793)./2.0;
t1981 = t1970./2.0;
t1982 = t29.*t1963;
t1985 = t1977./2.0;
t1986 = t12.*t25.*t1963;
t1996 = -t1991;
t2002 = t1994./2.0;
t2003 = -t2000;
t2004 = -t2001;
t2008 = t2005./2.0;
t2018 = t1263.*t1680;
t2021 = -t2015;
t2023 = -t2020;
t2028 = -t2026;
t2029 = t1680.*(t384+t472+t477+t26.*t29.*t132.*1.383e-1);
t2033 = t29.*t2027;
t2038 = t12.*t25.*t2027;
t2039 = t783+t1336+t1347;
t2040 = -t2037;
t2043 = t8.*t2034;
t2046 = -t2044;
t2050 = t1041.*t1793;
t2053 = t2.*t25.*t2034;
t2059 = t26.*t29.*t2034;
t2074 = t2072.*2.0;
t2076 = -t2072;
t2083 = (t1395.*t1680)./2.0;
t2088 = -t2085;
t2090 = t2085./2.0;
t2098 = t8.*t2094;
t2104 = t2.*t25.*t2094;
t2107 = t26.*t29.*t2094;
t2117 = t1503.*t1680;
t2119 = t1264.*t1793;
t2126 = t1534.*t1680;
t2133 = t2127./2.0;
t2146 = t1396.*t1793;
t2147 = t2143./2.0;
t2153 = t1602.*t1680;
t2156 = (t1496.*t1793)./2.0;
t2157 = (t1648.*t1680)./2.0;
t2166 = t2161./2.0;
t2168 = -t2167;
t2169 = t25.*t2165;
t2170 = t12.*t29.*t2165;
t2176 = t25.*t2174;
t2178 = t12.*t29.*t2174;
t2183 = t1680.*t1761;
t2186 = t2184./2.0;
t2190 = t1603.*t1793;
t2191 = t551+t1064+t1071+t1114+t1120;
t2192 = t552+t1061+t1113+t1115+t1121;
t2207 = t1681.*t1793;
t2220 = t1762.*t1793;
t2229 = t2228.*(-1.0./2.0);
t2241 = -t2239;
t2242 = t2239./2.0;
t2243 = t2240./2.0;
t2247 = t2245./2.0;
t2248 = t2246./2.0;
t2249 = t704+t705+t1092+t1103+t1223+t1226;
t2250 = t792+t804+t1142+t1149+t1285+t1293;
t2251 = t782+t817+t1150+t1163+t1276+t1281;
t2262 = t688+t950+t1376+t1378+t1624+t1629;
t2263 = t694+t938+t1365+t1367+t1630+t1637;
t2264 = t962+t965+t1277+t1278+t2154;
t2266 = -t2.*(t691+t934-t1367-t1630+t1371.*(t61-t239).*8.084033333333334e-4+t7.*t132.*(t289-t476+t171.*(t60-t190)).*8.084033333333334e-4);
t2268 = t2.*(t691+t934-t1367-t1630+t1371.*(t61-t239).*8.084033333333334e-4+t7.*t132.*(t289-t476+t171.*(t60-t190)).*8.084033333333334e-4).*(-1.0./2.0);
t2272 = t8.*t2270;
t2274 = t2.*t2271;
t2277 = t2.*t29.*t2270;
t2281 = t8.*t29.*t2271;
t2282 = t607+t775+t1382+t1391+t1722+t1736;
t2291 = t171.*t2270;
t2292 = t132.*t2271;
t2302 = t8.*t2301;
t2303 = t645+t852+t1404+t1425+t1755+t1769;
t2307 = t2.*t29.*t2301;
t2315 = t171.*t2301;
t1781 = t25.*t1780;
t1782 = t29.*t1780;
t1809 = -t1805;
t1831 = -t1823;
t1835 = t1823./2.0;
t1841 = -t1829;
t1842 = -t1830;
t1848 = -t1836;
t1850 = t1829./2.0;
t1855 = -t1843;
t1856 = t1840./2.0;
t1857 = t1843./2.0;
t1859 = -t1854;
t1860 = t1854./2.0;
t1870 = -t1862;
t1873 = t1862./2.0;
t1881 = -t1876;
t1882 = t1876./2.0;
t1889 = -t1887;
t1926 = t1923./2.0;
t1929 = -t1927;
t1938 = t721.*t1792;
t1943 = -t1939;
t1949 = t1939./2.0;
t1978 = (t789.*t1792)./2.0;
t1983 = -t1981;
t1987 = -t1985;
t1988 = t1982./2.0;
t1990 = -t1986;
t1995 = t1986./2.0;
t2013 = t943.*t1792;
t2030 = t2029./2.0;
t2042 = t2033./2.0;
t2045 = t2038./2.0;
t2047 = -t2043;
t2049 = t1040.*t1792;
t2052 = -t2050;
t2055 = t2050./2.0;
t2060 = -t2053;
t2063 = t2053./2.0;
t2065 = -t2059;
t2068 = t2059./2.0;
t2077 = -t2074;
t2092 = -t2090;
t2108 = -t2104;
t2109 = t2104./2.0;
t2113 = t2107./2.0;
t2118 = t1263.*t1792;
t2120 = -t2117;
t2121 = t2117./2.0;
t2123 = t1792.*(t384+t472+t477+t26.*t29.*t132.*1.383e-1);
t2132 = t2126./2.0;
t2145 = t1395.*t1792;
t2150 = t2146./2.0;
t2151 = -t2147;
t2155 = (t1495.*t1792)./2.0;
t2159 = t1503.*t1792;
t2171 = -t2169;
t2172 = t2169./2.0;
t2175 = t2170./2.0;
t2180 = t2176./2.0;
t2182 = t2178./2.0;
t2185 = t2183./2.0;
t2188 = -t2186;
t2189 = t1602.*t1792;
t2193 = (t8.*t2191)./2.0;
t2195 = t2.*t29.*t2191;
t2197 = (t2.*t2192)./2.0;
t2200 = t8.*t29.*t2192;
t2205 = t171.*t2191;
t2206 = t1680.*t1792;
t2208 = t132.*t2192;
t2219 = t1761.*t1792;
t2224 = t2220./2.0;
t2244 = -t2243;
t2253 = t2.*t2251;
t2256 = t608+t896+t1327+t1328+t1600+t1601;
t2269 = t786+t788+t1277+t1278+t2190;
t2273 = -t2272;
t2275 = t2272./2.0;
t2278 = t2274./2.0;
t2280 = -t2277;
t2283 = t2277./2.0;
t2285 = -t2281;
t2286 = t2281./2.0;
t2288 = t25.*t2282;
t2289 = t12.*t29.*t2282;
t2295 = -t2291;
t2297 = t2291./2.0;
t2298 = t2292./2.0;
t2300 = t874+t876+t1277+t1278+t2207;
t2304 = t2302./2.0;
t2309 = -t2307;
t2311 = t2307./2.0;
t2317 = t2315./2.0;
t2319 = t1493+t1494+t1821+t1822+t2153;
t2322 = t1647+t1663+t1764+t1930+t1931+t1977+t2302+t2305;
t1783 = t12.*t1781;
t1784 = t6.*t1782;
t1785 = t12.*t1782;
t1786 = -t1781;
t1787 = -t1782;
t1788 = t1782./2.0;
t1847 = -t1835;
t1853 = -t1850;
t1861 = -t1860;
t1875 = -t1873;
t1883 = -t1882;
t1928 = -t1926;
t1942 = -t1938;
t1948 = t1938./2.0;
t1954 = -t1949;
t1997 = -t1995;
t2032 = -t2030;
t2054 = t2049./2.0;
t2057 = -t2055;
t2066 = -t2063;
t2070 = -t2068;
t2111 = -t2109;
t2122 = -t2121;
t2124 = t2123./2.0;
t2136 = -t2132;
t2149 = t2145./2.0;
t2160 = -t2159;
t2163 = t2159./2.0;
t2173 = -t2172;
t2181 = -t2180;
t2187 = -t2185;
t2194 = -t2193;
t2196 = -t2195;
t2198 = t2195./2.0;
t2199 = -t2197;
t2202 = -t2200;
t2203 = t2200./2.0;
t2209 = t2205./2.0;
t2210 = -t2208;
t2211 = t2208./2.0;
t2223 = t2219./2.0;
t2255 = t2253./2.0;
t2276 = -t2275;
t2279 = -t2278;
t2284 = -t2283;
t2287 = -t2286;
t2290 = -t2288;
t2293 = t2288./2.0;
t2296 = t2289./2.0;
t2299 = -t2297;
t2306 = -t2304;
t2313 = -t2311;
t2320 = t1392+t1393+t1821+t1822+t2189;
t2321 = t1448+t1449+t1821+t1822+t2206;
t2325 = t1696+t2038+t2079+t2091+t2107+t2114+t2289+t2315+t2316;
t1790 = t1783./2.0;
t1791 = t1784./2.0;
t1953 = -t1948;
t2125 = -t2124;
t2152 = -t2149;
t2164 = -t2163;
t2201 = -t2198;
t2204 = -t2203;
t2212 = -t2211;
t2294 = -t2293;
t2326 = t1689+t2045+t2078+t2089+t2113+t2116+t2296+t2317+t2318;
t2329 = t1812+t1947+t1997+t2070+t2071+t2101+t2105+t2137+t2138+t2261+t2298+t2299;
t2332 = t1804+t1937+t2033+t2097+t2100+t2106+t2108+t2130+t2131+t2290+t2309+t2312;
t2323 = t1662+t1676+t1770+t1790+t1856+t1861+t1933+t1936+t1985+t2175+t2209+t2212;
t2327 = qd6.*t2326;
t2330 = qd6.*t2329;
t2324 = qd6.*t2323;
t2328 = -t2327;
t2331 = -t2330;
et1 = -qd3.*(t1431+qd2.*(t882+t897+t967+t968)+qd3.*(t967+t968-t8.*t342.*t502+t2.*t342.*t513))+qd1.*(qd3.*(t480+t502.*t708.*2.0-t513.*t702.*2.0)+qd2.*(t480-t606.*t702.*2.0+t605.*t708.*2.0)+qd4.*(t480-t25.*t744.*1.639e-1+t25.*t92.*t708))+qdd4.*t1415+qdd3.*t1532+qdd2.*t1590+qdd1.*(t35./5.0e+3+t36.*2.338600833333333e-3+t702.^2+t708.^2)-qd4.*(t1431+qd3.*(t663+t668+t1410)+qd2.*(t742+t768+t1410));
et2 = -qd2.*(t1431+qd3.*(t862+t881+t967+t968)-qd2.*(-t2.*t405.*t606+t8.*t405.*t605+t2.*t420.*t702+t8.*t420.*t708));
et3 = -qd5.*(-t380.*t1036-t602.*t1100+t371.*(t423-t716)+t1102.*(t241-t419)-t12.*t25.*t68.*2.031081666666667e-3+t2.*t29.*t1097+t8.*t29.*(t614-t638))+qd4.*(t1054-t1124-t1235-t1238+t1349-t1714-t1716+t1863+t575.*(t423-t716)+t1100.*(t421-t432-t619+t718))+qd3.*(t1054-t1124-t1235-t1238+t1499-t1714-t1716+t1863+t836.*(t423-t716)+t1100.*(t421-t432-t619+t718));
et4 = qd2.*(t1054-t1124-t1235-t1238+t1543-t1714-t1716+t1863+t916.*(t423-t716)+t1100.*(t421-t432-t619+t718));
et5 = qdd4.*(t1204+t1221+t1298+t1299)+qdd3.*(t1204+t1221+t1353+t1358)+qdd2.*(t1204+t1221+t1420+t1423)-qd4.*(qd4.*(t1305+t1307+t1686+t1699+t2.*t361.*t577-t8.*t361.*t575)+qd5.*(t679+t685+t1116+t1117-t1187-t1189)+qd3.*(t1072+t1081+t1305+t1307+t1686+t1699)+qd2.*(t1141+t1146+t1305+t1307+t1686+t1699))+qd3.*(qd3.*(t1362+t1363+t1687+t1698-t2.*t479.*t829+t8.*t479.*t836)-qd5.*(t776+t787+t1116+t1117-t1187-t1189)-qd4.*(t952+t966+t1305+t1307+t1686+t1699)+qd2.*(t1208+t1225+t1362+t1363+t1687+t1698));
et6 = qd1.*(qd4.*(t1073+t575.*t1100.*2.0-t577.*t1102.*2.0)+qd3.*(t1073-t829.*t1102.*2.0+t836.*t1100.*2.0)+qd2.*(t1073+t916.*t1100.*2.0-t918.*t1102.*2.0)-qd5.*(t12.*t68.*2.031081666666667e-3+t371.*t1100.*2.0+t380.*t1102.*2.0))+qdd1.*(t1009+t1100.^2+t1102.^2)+qd5.*(et3+et4)+qd2.*(qd2.*(t1687+t1698-t2.*t580.*t918+t8.*t580.*t916+t2.*t581.*t1102+t8.*t581.*t1100)-qd5.*(t873+t875+t1116+t1117-t1187-t1189)-qd4.*(t1006+t1030+t1305+t1307+t1686+t1699)+qd3.*(t1200+t1207+t1362+t1363+t1687+t1698))-qdd5.*(t1620+t1623+t25.*t1009+t2.*t29.*t1183+t8.*t29.*t1184);
et7 = -qd5.*(t1952-t1958-t6.*t1185+t133.*t1501-t132.*t1904+t171.*(t324-t344+t730-t731-t765+t12.*t39.*(t60-t190).*8.084033333333334e-4)-t170.*(t329+t834+t236.*(t61-t239).*8.084033333333334e-4)+t378.*(t426-t1001)+t370.*(t443-t1013)-t12.*t29.*t1242);
et8 = qd4.*(t1199-t1414+t1528+t1539+t1992-t1994+t2012+t2017+t574.*(t443-t1013)+t29.*t30.*(t329+t834+t236.*(t61-t239).*8.084033333333334e-4))+qd3.*(t1199-t1414+t1539+t1619+t1992-t1994+t2012+t2017+t835.*(t443-t1013)+t29.*t30.*(t329+t834+t236.*(t61-t239).*8.084033333333334e-4));
et9 = qd2.*(t1199-t1414+t1539+t1651+t1992-t1994+t2012+t2017+t915.*(t443-t1013)+t29.*t30.*(t329+t834+t236.*(t61-t239).*8.084033333333334e-4));
et10 = -qdd6.*(t12.*t1185+t171.*t1501-t132.*(t329+t834+t236.*(t61-t239).*8.084033333333334e-4)+t1101.*(t426-t1001)+t1099.*(t443-t1013))+qd4.*(qd3.*(t1337-t1338+t1525+t1526+t1944+t1946)+qd2.*(t1402-t1406+t1525+t1526+t1944+t1946)+qd4.*(t1525+t1526+t1944+t1946-t2.*t576.*t773+t8.*t574.*t773)-qd5.*(t1039+t1049+t1380+t1385+t1908+t1909))+qd3.*(qd4.*(t1246-t1247+t1525+t1526+t1944+t1946)+qd2.*(t1476-t1478+t1577+t1579+t1944+t1946)+qd3.*(t1577+t1579+t1944+t1946-t2.*t828.*t890+t8.*t835.*t890)-qd5.*(t1125+t1132+t1380+t1385+t1908+t1909));
et11 = qdd4.*(-t1518+t1522+t1523+t2.*(t329+t834+t236.*(t61-t239).*8.084033333333334e-4))+qdd3.*(-t1518+t1572+t1573+t2.*(t329+t834+t236.*(t61-t239).*8.084033333333334e-4))+qdd2.*(-t1518+t1591+t1592+t2.*(t329+t834+t236.*(t61-t239).*8.084033333333334e-4));
et12 = qdd1.*(t1164+t1099.^2+t1101.^2)-qd6.*(et7+et8+et9)+qd5.*(qd5.*(-t25.*t1242+t370.*t1321+t378.*t1314+t902.*t1099+t914.*t1101+t8.*t29.*t1904+t2.*t29.*(t324-t344+t730-t731-t765+t12.*t39.*(t60-t190).*8.084033333333334e-4))+qd4.*(t1185+t1398+t1541+t1542+t1568+t1575+t1967+t1976+t2082+t2086)+qd3.*(t1185+t1398+t1541+t1542+t1641+t1657+t1967+t1976+t2082+t2086)+qd2.*(t1185+t1398+t1541+t1542+t1691+t1713+t1967+t1976+t2082+t2086));
et13 = -qd1.*(qd4.*(t1354-t574.*t1099.*2.0+t576.*t1101.*2.0)+qd3.*(t1354+t828.*t1101.*2.0-t835.*t1099.*2.0)+qd2.*(t1354-t915.*t1099.*2.0+t917.*t1101.*2.0)+qd5.*(-t169+t662-t677+t370.*t1099.*2.0+t378.*t1101.*2.0))+qd2.*(qd2.*(t1944+t1946-t2.*t917.*t942+t8.*t915.*t942+t2.*t953.*t1101+t8.*t953.*t1099)+qd4.*(t1304-t1306+t1525+t1526+t1944+t1946)+qd3.*(t1465-t1468+t1577+t1579+t1944+t1946)-qd5.*(t1168+t1170+t1380+t1385+t1908+t1909))-qdd5.*(t1775+t1776+t25.*t1164+t2.*t29.*t1501+t8.*t29.*(t329+t834+t236.*(t61-t239).*8.084033333333334e-4));
et14 = t127+t220+qd2.*(qd1.*t1162+qd3.*(-t450-t453-t1066.*2.0+t1324+(t812.*(t2.*(t296-t2.*t9.*(1.53e+2./2.5e+2))+t8.*(t299-t8.*t9.*(1.53e+2./2.5e+2))))./2.0+t15.*t20.*t275.*8.5845e-1+t17.*t20.*t275.*8.5845e-1)+qd2.*(-t568.*t812+t15.*t274.*t275+t17.*t274.*t275))-qdd1.*t1128+qdd3.*t1802+qdd2.*(t211+t212+t15.*t300+t17.*t300+t812.^2)-qd1.*(t1000+qd2.*t1162+qd1.*((t146.*t448)./1.0e+4-t296.*t400));
et15 = qd3.*(t999+qd3.*(-t1066-t1193+t980.*(t2.*(t296-t2.*t9.*(1.53e+2./2.5e+2))+t8.*(t299-t8.*t9.*(1.53e+2./2.5e+2)))+t15.*t109.*t275+t17.*t109.*t275)+qd2.*(t450+t452+t453+t459+t1326+t1345));
et16 = t127+t220+t229+qdd1.*t1590+qdd3.*t2177+qdd4.*t2213+qdd2.*(t519+t521+t15.*t429+t17.*t429+t1274.^2)-qd4.*(qd3.*(t506+t508+t509+t512+t585+t588+t1778+t1801+t1803)+qd4.*(t585+t588+t1485+t1627+t1375.*(t936-t937))-qd2.*(-t586-t589+t594+t595+t1834+(t1108.*(t936-t937))./2.0)-qd1.*(t743-t760+t1411))-qd1.*(qd1.*(t487-t606.*t702+t605.*t708)-qd2.*t2095+qd3.*(t862+t881+t900-t903+t989+t990)+qd4.*(-t743+t760+t1411))+qd3.*(qd1.*(-t900+t903+t989+t990)+qd2.*(t750-t752+t753-t754+t1690+t1697)-qd4.*(t496+t499+t520+t522+t585+t588+t1352+t1485+t1801+t1808)-qd3.*(-t948.*t1274+t15.*t351.*t405+t17.*t351.*t405));
et17 = -qd2.*(qd1.*t2095+qd3.*(t750+t753+t1690-t948.*t1274.*(3.0./2.0)+t15.*t351.*t405.*(3.0./2.0)+t17.*t351.*t405.*(3.0./2.0))+qd4.*(t594+t595-t1480.*2.0+t1834+(t1108.*(t936-t937))./2.0+t15.*t29.*t405.*1.22925e-1+t17.*t29.*t405.*1.22925e-1)-qd2.*(t1108.*t1274+t15.*t405.*t420+t17.*t405.*t420));
et18 = qd2.*(t1179+t1300-t1301-t1377+t1753+t1763-t1893+t2188-t2242+t2243+t25.*(t527+t813)+t2.*t29.*(t551-t821)+t8.*t29.*(t552-t822)+(t8.*t581.*(t423-t716))./2.0)-qd1.*(t710+t729-t830-t969+t991-t1173+t1557+t1874+(t916.*(t423-t716))./2.0+(t1100.*(t421-t432-t619+t718))./2.0)+qd4.*(t1179+t1261+t1267+t1300-t1301+t1673+t1674-t1733+t1746+t2009-t2184+t2224-t2242+t2243+t25.*(t527+t813)+t8.*t580.*(t421-t432-t619+t718)+t2.*t29.*(t551-t821)+t8.*t29.*(t552-t822));
et19 = qd3.*(t1179+t1300-t1301-t1332+t1730+t1731+t1746-t1845+t2167-t2184-t2242+t2243+t25.*(t527+t813)+t8.*t580.*(t421-t432-t619+t718)+t2.*t29.*(t551-t821)+t8.*t29.*(t552-t822)+(t8.*t481.*(t423-t716))./2.0)-qd5.*(t1147+t1153+t1361+t1479+t1484+t1593+t1707+t1771+t1773+t1837+t1839+t2073+t2231+t2247+t2248-t790.*t1681-t8.*t580.*t602+t2.*t580.*(t241-t419));
et20 = t127+t220+t228+t256+t265+qd1.*(-qd4.*(t527+t813+t1006+t1030+t1151-t1156+t1316+t1318+t1706+t1708)-qd1.*(t235+t525+t549+t916.*t1100-t918.*t1102)+qd2.*(t1159+t1292+t1294+t1442+t1443+t1705+t1711)+qd3.*(t1159+t1200+t1207-t1227+t1230+t1384+t1386+t1705+t1711)+qd5.*(-t873-t875+t1074+t1131+t1187+t1189+t1251+t1252+t1335+t1561+t1565+t1724+t1725+t1877+t1878))+qd5.*(et18+et19);
et21 = -qd2.*(qd3.*(t992+t994+t1202+t1211+t2081-t1396.*t1681.*(3.0./2.0)-t15.*t481.*t580.*(3.0./2.0)-t17.*t481.*t580.*(3.0./2.0))+qd4.*(t884.*(3.0./2.0)+t885.*(3.0./2.0)+t905+t906+t1202+t1211-t1924.*2.0+t2156+t2158)-qd5.*(t1192+t1201+t1234+t1236+t1313+t1320+t1377+t1387+t1456+t1457+t1756+t1759-t1824.*2.0+t1893+t2186+t6.*t15.*t130.*t580+t6.*t17.*t130.*t580)-qd2.*(t1203+t1209+t1496.*t1681+t15.*t580.*t581+t17.*t580.*t581)+qd1.*(t553+t798+t1292+t1294+t1442+t1443))+qdd3.*t2264+qdd4.*t2300+qdd2.*(t1277+t1278+t15.*t587+t17.*t587+t1681.^2)+qdd5.*(t1302-t1303-t1356-t2019+t25.*(t530-t803)+t8.*t580.*(t423-t716))+qdd1.*(t1160+t1420+t1423);
et22 = qd4.*(-qd4.*(t884+t885+t1202+t1211+t1925+t2052+t1649.*t1793)+qd5.*(t558+t560+t723+t726+t1192+t1201+t1234+t1236+t1271+t1275+t1313+t1320+t1456+t1457+t1673+t1674+t1832+t1943+t2009+t2224)+qd1.*(t540+t814-t1151+t1156+t1316+t1318)+qd3.*(t824+t825+t826+t827-t884-t885+t1203+t1209+t2127-t2148+t2150)+qd2.*(t905+t906-t907-t908+t1203+t1209+t2156+t2158))+qd3.*(qd5.*(t669+t672+t723+t726+t1192+t1201+t1234+t1236+t1313+t1320+t1332+t1333+t1456+t1457+t1730+t1731+t1800+t1832+t1845+t2167)-qd1.*(t553+t798+t1227-t1230+t1384+t1386)-qd4.*(t824+t825+t826+t827+t884+t885+t1202+t1211+t1886+t1925+t2148+t2150)+qd2.*(t992+t993+t994+t995+t1203+t1209+t2081+t2084)+qd3.*(t1203+t1209+t1396.*t1681+t15.*t481.*t580+t17.*t481.*t580));
